simulink model "RealModel"  (R2016a)
(part 3 of 7)

x_dotdot = [x2, (0. + ((0.12348*cos(x1) - 0.9716*cos(x3))*(-0.4858*sin(2.*x1)*(0.12347999999999999*sin(x1) + 0.4858*cos(x3)*sin(2.*x1))*sin(x3)*(cos(x3)*(-0.0005*cos(2.*x1) - 0.7010000000000001*sin(2.*x1)) - 1.1102230246251565^-16*sin(x1)*sin(x3)) - 0.34006*sin(2.*x1)*sin(x3)*(cos(x3)*(-0.0005*cos(2.*x1) - 0.7010000000000001*sin(2.*x1)) - 1.1102230246251565^-16*sin(x1)*sin(x3))^2 + 0.34006*(2.0940000000000003 - 0.7010000000000001*cos(2.*x1) + 0.0005*sin(2.*x1))*sin(2.*x1)*sin(x3)*((1.7510000000000001 + 2.1684043449710084^-19*0) + cos(2.*x1)*((0.3505 - 5.421010862427521^-20*0) + (0.3505 - 5.421010862427521^-20*0)*cos(2.*x3)) + cos(2.*x3)*(0.343 - (0.00025 - 2.8760394919088917^-17*0)*sin(2.*x1)) - (0.00025 - 2.8760394919088917^-17*0)*sin(2.*x1) + 1.1102230246251562^-16*cos(x1)*sin(2.*x3)) + (2.0940000000000003 - 0.7010000000000001*cos(2.*x1) + 0.0005*sin(2.*x1))*(0.12347999999999999*sin(x1) + 0.4858*cos(x3)*sin(2.*x1))*(-0.12347999999999999*cos(x1)*sin(x3) + (-0.24289999999999998 - 0.24289999999999998*cos(2.*x1))*sin(2.*x3))) - (0. + (2.0940000000000003 - 0.7010000000000001*cos(2.*x1) + 0.0005*sin(2.*x1))*(-1.1102230246251565^-16*cos(x1)*cos(x3) - 1.4080000000000001*sin(x3)))*((0.8627035999999999 + cos(2.*x1)*(0.17003 - 0.17003*cos(2.*x3)) - 0.17003*cos(2.*x3))*(0.12347999999999999*sin(x1) + 0.4858*cos(x3)*sin(2.*x1)) + 0.34006*sin(2.*x1)*sin(x3)*(-0.12347999999999999*cos(x1)*sin(x3) - (0.2429 + 2.7105054312137602^-20*0)*(1. + 1.*cos(2.*x1))*sin(2.*x3))) - 0.12348*sin(x1)*sin(x3)*(-((0.8627035999999999 + cos(2.*x1)*(0.17003 - 0.17003*cos(2.*x3)) - 0.17003*cos(2.*x3))*(cos(x3)*(-0.0005*cos(2.*x1) - 0.7010000000000001*sin(2.*x1)) - 1.1102230246251565^-16*sin(x1)*sin(x3))^2) + (0.8627035999999999 + cos(2.*x1)*(0.17003 - 0.17003*cos(2.*x3)) - 0.17003*cos(2.*x3))*(2.0940000000000003 - 0.7010000000000001*cos(2.*x1) + 0.0005*sin(2.*x1))*((1.7510000000000001 + 2.1684043449710084^-19*0) + cos(2.*x1)*((0.3505 - 5.421010862427521^-20*0) + (0.3505 - 5.421010862427521^-20*0)*cos(2.*x3)) + cos(2.*x3)*(0.343 - (0.00025 - 2.8760394919088917^-17*0)*sin(2.*x1)) - (0.00025 - 2.8760394919088917^-17*0)*sin(2.*x1) + 1.1102230246251562^-16*cos(x1)*sin(2.*x3)) + 0.4858*sin(2.*x1)*sin(x3)*(cos(x3)*(-0.0005*cos(2.*x1) - 0.7010000000000001*sin(2.*x1)) - 1.1102230246251565^-16*sin(x1)*sin(x3))*(-0.12347999999999999*cos(x1)*sin(x3) - (0.2429 + 2.7105054312137602^-20*0)*(1. + 1.*cos(2.*x1))*sin(2.*x3)) - (2.0940000000000003 - 0.7010000000000001*cos(2.*x1) + 0.0005*sin(2.*x1))*(-0.12347999999999999*cos(x1)*sin(x3) + (-0.24289999999999998 - 0.24289999999999998*cos(2.*x1))*sin(2.*x3))*(-0.12347999999999999*cos(x1)*sin(x3) - (0.2429 + 2.7105054312137602^-20*0)*(1. + 1.*cos(2.*x1))*sin(2.*x3))))*((1.4288690166235203*cos(x1) + 1.6499158227686102*sin(x1))*u1 + 1.6499158227686104*sin(x1)*u2 + 1.6499158227686102*sin(x1)*u3 + 0.68012*sin(2.*x1)*x10*x2 + cos(x1)*(-1.4288690166235203*u3 - 0.12348*sin(x3)*x2^2) - 0.24696*cos(x3)*sin(x1)*x2*x4 - 0.9716000000000001*sin(2.*x1)*x2*x4 - 0.12348*cos(x1)*sin(x3)*x4^2 + ((0.12347999999999998*cos(x1) + 0.9716*cos(x1)^2*cos(x3) - 0.9716*cos(x3)*sin(x1)^2)*x2 - 0.4858*sin(2*x1)*sin(x3)*x4)*x6 + (-0.68012*cos(2.*x1)*sin(x3)*x2 - 0.34006*cos(x3)*sin(2.*x1)*x4)*x8) + (0.8627035999999999 + cos(2.*x1)*(0.17003 - 0.17003*cos(2.*x3)) - 0.17003*cos(2.*x3))*(-0.9715999999999999*cos(x1)^2 + 0.12347999999999999*cos(x1)*cos(x3) - 1.9431999999999998*sin(x1)^2)*(0.12347999999999999*sin(x1) + 0.4858*cos(x3)*sin(2.*x1))*(-1.1102230246251565^-16*cos(x1)*cos(x3) - 1.4080000000000001*sin(x3))*(-17.304840000000002*cos(x1)*sin(x3) + (-0.8164965809277263*cos(x1) - 0.9428090415820632*sin(x1))*u1 + (0.6123724356957947*cos(x1) - 0.9428090415820637*sin(x1))*u2 + 2.041241452319315*cos(x1)*u3 - 0.9428090415820632*sin(x1)*u3 - 0.9716*sin(2.*x1)*x10*x2 + 1.1102230246251565^-16*cos(x1)*x2^2 + (-1.3877787807814457^-17*cos(x1)*sin(x3)*x10 + (0.001*cos(2.*x1) + 1.4020000000000001*sin(2.*x1))*x2)*x4 + (-1.1102230246251565^-16*cos(x1)*cos(2.*x3) + ((0.343 - 1.4444474582904269^-34*0) + (0.35050000000000003 - 1.6263032587282571^-19*0)*cos(2.*x1) - (0.00025 - 1.3877787807814454^-16*0)*sin(2.*x1))*sin(2.*x3))*x6^2 + (0.34006000000000003*cos(x3)*sin(2.*x1)*x10 + (-0.9716 + 0.9716*cos(2.*x1))*sin(x3)*x2)*x8 + (-0.34006000000000003*cos(2.*x1)*cos(x3)*sin(x3) - 0.17003000000000001*sin(2.*x3))*x8^2 + x6*(0.4858*sin(2.*x1)*sin(x3)*x10 + (cos(x3)*(1.4080000000000001 - 1.4020000000000001*cos(2.*x1) + 0.001*sin(2.*x1)) - 2.220446049250313^-16*cos(x1)*sin(x3))*x2 + 1.1102230246251565^-16*sin(2.*x1)*sin(x3)*x4 + (0.12348*cos(x1)*cos(x3) + (0.4858 + 0.4858*cos(2.*x1))*cos(2.*x3))*x8)) + 0.4858*(0.12348*cos(x1) - 0.9716*cos(x3))*(0.12347999999999999 + 0.9715999999999999*cos(x1)*cos(x3))*sin(x1)*sin(2.*x1)*(0.12347999999999999*sin(x1) + 0.4858*cos(x3)*sin(2.*x1))*sin(x3)*(-17.304840000000002*cos(x1)*sin(x3) + (-0.8164965809277263*cos(x1) - 0.9428090415820632*sin(x1))*u1 + (0.6123724356957947*cos(x1) - 0.9428090415820637*sin(x1))*u2 + 2.041241452319315*cos(x1)*u3 - 0.9428090415820632*sin(x1)*u3 - 0.9716*sin(2.*x1)*x10*x2 + 1.1102230246251565^-16*cos(x1)*x2^2 + (-1.3877787807814457^-17*cos(x1)*sin(x3)*x10 + (0.001*cos(2.*x1) + 1.4020000000000001*sin(2.*x1))*x2)*x4 + (-1.1102230246251565^-16*cos(x1)*cos(2.*x3) + ((0.343 - 1.4444474582904269^-34*0) + (0.35050000000000003 - 1.6263032587282571^-19*0)*cos(2.*x1) - (0.00025 - 1.3877787807814454^-16*0)*sin(2.*x1))*sin(2.*x3))*x6^2 + (0.34006000000000003*cos(x3)*sin(2.*x1)*x10 + (-0.9716 + 0.9716*cos(2.*x1))*sin(x3)*x2)*x8 + (-0.34006000000000003*cos(2.*x1)*cos(x3)*sin(x3) - 0.17003000000000001*sin(2.*x3))*x8^2 + x6*(0.4858*sin(2.*x1)*sin(x3)*x10 + (cos(x3)*(1.4080000000000001 - 1.4020000000000001*cos(2.*x1) + 0.001*sin(2.*x1)) - 2.220446049250313^-16*cos(x1)*sin(x3))*x2 + 1.1102230246251565^-16*sin(2.*x1)*sin(x3)*x4 + (0.12348*cos(x1)*cos(x3) + (0.4858 + 0.4858*cos(2.*x1))*cos(2.*x3))*x8)) + 0.165201148*sin(2.*x1)^2*(0.12347999999999999*sin(x1) + 0.4858*cos(x3)*sin(2.*x1))*(-1.1102230246251565^-16*cos(x1)*cos(x3) - 1.4080000000000001*sin(x3))*sin(x3)^2*(-17.304840000000002*cos(x1)*sin(x3) + (-0.8164965809277263*cos(x1) - 0.9428090415820632*sin(x1))*u1 + (0.6123724356957947*cos(x1) - 0.9428090415820637*sin(x1))*u2 + 2.041241452319315*cos(x1)*u3 - 0.9428090415820632*sin(x1)*u3 - 0.9716*sin(2.*x1)*x10*x2 + 1.1102230246251565^-16*cos(x1)*x2^2 + (-1.3877787807814457^-17*cos(x1)*sin(x3)*x10 + (0.001*cos(2.*x1) + 1.4020000000000001*sin(2.*x1))*x2)*x4 + (-1.1102230246251565^-16*cos(x1)*cos(2.*x3) + ((0.343 - 1.4444474582904269^-34*0) + (0.35050000000000003 - 1.6263032587282571^-19*0)*cos(2.*x1) - (0.00025 - 1.3877787807814454^-16*0)*sin(2.*x1))*sin(2.*x3))*x6^2 + (0.34006000000000003*cos(x3)*sin(2.*x1)*x10 + (-0.9716 + 0.9716*cos(2.*x1))*sin(x3)*x2)*x8 + (-0.34006000000000003*cos(2.*x1)*cos(x3)*sin(x3) - 0.17003000000000001*sin(2.*x3))*x8^2 + x6*(0.4858*sin(2.*x1)*sin(x3)*x10 + (cos(x3)*(1.4080000000000001 - 1.4020000000000001*cos(2.*x1) + 0.001*sin(2.*x1)) - 2.220446049250313^-16*cos(x1)*sin(x3))*x2 + 1.1102230246251565^-16*sin(2.*x1)*sin(x3)*x4 + (0.12348*cos(x1)*cos(x3) + (0.4858 + 0.4858*cos(2.*x1))*cos(2.*x3))*x8)) - (1.0327336 - 0.34006*cos(2.*x1))*(0.8627035999999999 + cos(2.*x1)*(0.17003 - 0.17003*cos(2.*x3)) - 0.17003*cos(2.*x3))*(-1.1102230246251565^-16*cos(x1)*cos(x3) - 1.4080000000000001*sin(x3))*(cos(x3)*(-0.0005*cos(2.*x1) - 0.701*sin(2.*x1)) - 1.1102230246251564^-16*sin(x1)*sin(x3))*(-17.304840000000002*cos(x1)*sin(x3) + (-0.8164965809277263*cos(x1) - 0.9428090415820632*sin(x1))*u1 + (0.6123724356957947*cos(x1) - 0.9428090415820637*sin(x1))*u2 + 2.041241452319315*cos(x1)*u3 - 0.9428090415820632*sin(x1)*u3 - 0.9716*sin(2.*x1)*x10*x2 + 1.1102230246251565^-16*cos(x1)*x2^2 + (-1.3877787807814457^-17*cos(x1)*sin(x3)*x10 + (0.001*cos(2.*x1) + 1.4020000000000001*sin(2.*x1))*x2)*x4 + (-1.1102230246251565^-16*cos(x1)*cos(2.*x3) + ((0.343 - 1.4444474582904269^-34*0) + (0.35050000000000003 - 1.6263032587282571^-19*0)*cos(2.*x1) - (0.00025 - 1.3877787807814454^-16*0)*sin(2.*x1))*sin(2.*x3))*x6^2 + (0.34006000000000003*cos(x3)*sin(2.*x1)*x10 + (-0.9716 + 0.9716*cos(2.*x1))*sin(x3)*x2)*x8 + (-0.34006000000000003*cos(2.*x1)*cos(x3)*sin(x3) - 0.17003000000000001*sin(2.*x3))*x8^2 + x6*(0.4858*sin(2.*x1)*sin(x3)*x10 + (cos(x3)*(1.4080000000000001 - 1.4020000000000001*cos(2.*x1) + 0.001*sin(2.*x1)) - 2.220446049250313^-16*cos(x1)*sin(x3))*x2 + 1.1102230246251565^-16*sin(2.*x1)*sin(x3)*x4 + (0.12348*cos(x1)*cos(x3) + (0.4858 + 0.4858*cos(2.*x1))*cos(2.*x3))*x8)) - 0.12348*(0.12347999999999999 + 0.9715999999999999*cos(x1)*cos(x3))*(0.8627035999999999 + cos(2.*x1)*(0.17003 - 0.17003*cos(2.*x3)) - 0.17003*cos(2.*x3))*sin(x1)^2*sin(x3)*(cos(x3)*(-0.0005*cos(2.*x1) - 0.701*sin(2.*x1)) - 1.1102230246251564^-16*sin(x1)*sin(x3))*(-17.304840000000002*cos(x1)*sin(x3) + (-0.8164965809277263*cos(x1) - 0.9428090415820632*sin(x1))*u1 + (0.6123724356957947*cos(x1) - 0.9428090415820637*sin(x1))*u2 + 2.041241452319315*cos(x1)*u3 - 0.9428090415820632*sin(x1)*u3 - 0.9716*sin(2.*x1)*x10*x2 + 1.1102230246251565^-16*cos(x1)*x2^2 + (-1.3877787807814457^-17*cos(x1)*sin(x3)*x10 + (0.001*cos(2.*x1) + 1.4020000000000001*sin(2.*x1))*x2)*x4 + (-1.1102230246251565^-16*cos(x1)*cos(2.*x3) + ((0.343 - 1.4444474582904269^-34*0) + (0.35050000000000003 - 1.6263032587282571^-19*0)*cos(2.*x1) - (0.00025 - 1.3877787807814454^-16*0)*sin(2.*x1))*sin(2.*x3))*x6^2 + (0.34006000000000003*cos(x3)*sin(2.*x1)*x10 + (-0.9716 + 0.9716*cos(2.*x1))*sin(x3)*x2)*x8 + (-0.34006000000000003*cos(2.*x1)*cos(x3)*sin(x3) - 0.17003000000000001*sin(2.*x3))*x8^2 + x6*(0.4858*sin(2.*x1)*sin(x3)*x10 + (cos(x3)*(1.4080000000000001 - 1.4020000000000001*cos(2.*x1) + 0.001*sin(2.*x1)) - 2.220446049250313^-16*cos(x1)*sin(x3))*x2 + 1.1102230246251565^-16*sin(2.*x1)*sin(x3)*x4 + (0.12348*cos(x1)*cos(x3) + (0.4858 + 0.4858*cos(2.*x1))*cos(2.*x3))*x8)) + 0.34006*(0.12348*cos(x1) - 0.9716*cos(x3))*(0.12347999999999999 + 0.9715999999999999*cos(x1)*cos(x3))*sin(x1)*sin(2.*x1)*sin(x3)*(cos(x3)*(-0.0005*cos(2.*x1) - 0.701*sin(2.*x1)) - 1.1102230246251564^-16*sin(x1)*sin(x3))*(-17.304840000000002*cos(x1)*sin(x3) + (-0.8164965809277263*cos(x1) - 0.9428090415820632*sin(x1))*u1 + (0.6123724356957947*cos(x1) - 0.9428090415820637*sin(x1))*u2 + 2.041241452319315*cos(x1)*u3 - 0.9428090415820632*sin(x1)*u3 - 0.9716*sin(2.*x1)*x10*x2 + 1.1102230246251565^-16*cos(x1)*x2^2 + (-1.3877787807814457^-17*cos(x1)*sin(x3)*x10 + (0.001*cos(2.*x1) + 1.4020000000000001*sin(2.*x1))*x2)*x4 + (-1.1102230246251565^-16*cos(x1)*cos(2.*x3) + ((0.343 - 1.4444474582904269^-34*0) + (0.35050000000000003 - 1.6263032587282571^-19*0)*cos(2.*x1) - (0.00025 - 1.3877787807814454^-16*0)*sin(2.*x1))*sin(2.*x3))*x6^2 + (0.34006000000000003*cos(x3)*sin(2.*x1)*x10 + (-0.9716 + 0.9716*cos(2.*x1))*sin(x3)*x2)*x8 + (-0.34006000000000003*cos(2.*x1)*cos(x3)*sin(x3) - 0.17003000000000001*sin(2.*x3))*x8^2 + x6*(0.4858*sin(2.*x1)*sin(x3)*x10 + (cos(x3)*(1.4080000000000001 - 1.4020000000000001*cos(2.*x1) + 0.001*sin(2.*x1)) - 2.220446049250313^-16*cos(x1)*sin(x3))*x2 + 1.1102230246251565^-16*sin(2.*x1)*sin(x3)*x4 + (0.12348*cos(x1)*cos(x3) + (0.4858 + 0.4858*cos(2.*x1))*cos(2.*x3))*x8)) + 0.11564080359999998*sin(2.*x1)^2*(-1.1102230246251565^-16*cos(x1)*cos(x3) - 1.4080000000000001*sin(x3))*sin(x3)^2*(cos(x3)*(-0.0005*cos(2.*x1) - 0.701*sin(2.*x1)) - 1.1102230246251564^-16*sin(x1)*sin(x3))*(-17.304840000000002*cos(x1)*sin(x3) + (-0.8164965809277263*cos(x1) - 0.9428090415820632*sin(x1))*u1 + (0.6123724356957947*cos(x1) - 0.9428090415820637*sin(x1))*u2 + 2.041241452319315*cos(x1)*u3 - 0.9428090415820632*sin(x1)*u3 - 0.9716*sin(2.*x1)*x10*x2 + 1.1102230246251565^-16*cos(x1)*x2^2 + (-1.3877787807814457^-17*cos(x1)*sin(x3)*x10 + (0.001*cos(2.*x1) + 1.4020000000000001*sin(2.*x1))*x2)*x4 + (-1.1102230246251565^-16*cos(x1)*cos(2.*x3) + ((0.343 - 1.4444474582904269^-34*0) + (0.35050000000000003 - 1.6263032587282571^-19*0)*cos(2.*x1) - (0.00025 - 1.3877787807814454^-16*0)*sin(2.*x1))*sin(2.*x3))*x6^2 + (0.34006000000000003*cos(x3)*sin(2.*x1)*x10 + (-0.9716 + 0.9716*cos(2.*x1))*sin(x3)*x2)*x8 + (-0.34006000000000003*cos(2.*x1)*cos(x3)*sin(x3) - 0.17003000000000001*sin(2.*x3))*x8^2 + x6*(0.4858*sin(2.*x1)*sin(x3)*x10 + (cos(x3)*(1.4080000000000001 - 1.4020000000000001*cos(2.*x1) + 0.001*sin(2.*x1)) - 2.220446049250313^-16*cos(x1)*sin(x3))*x2 + 1.1102230246251565^-16*sin(2.*x1)*sin(x3)*x4 + (0.12348*cos(x1)*cos(x3) + (0.4858 + 0.4858*cos(2.*x1))*cos(2.*x3))*x8)) + 0.12348*(0.8627035999999999 + cos(2.*x1)*(0.17003 - 0.17003*cos(2.*x3)) - 0.17003*cos(2.*x3))*sin(x1)*(-0.9715999999999999*cos(x1)^2 + 0.12347999999999999*cos(x1)*cos(x3) - 1.9431999999999998*sin(x1)^2)*sin(x3)*((1.7510000000000001 + 2.1684043449710084^-19*0) + cos(2.*x1)*((0.3505 - 5.421010862427521^-20*0) + (0.3505 - 5.421010862427521^-20*0)*cos(2.*x3)) + cos(2.*x3)*(0.343 - (0.00025 - 2.8760394919088917^-17*0)*sin(2.*x1)) - (0.00025 - 2.8760394919088917^-17*0)*sin(2.*x1) + 1.1102230246251562^-16*cos(x1)*sin(2.*x3))*(-17.304840000000002*cos(x1)*sin(x3) + (-0.8164965809277263*cos(x1) - 0.9428090415820632*sin(x1))*u1 + (0.6123724356957947*cos(x1) - 0.9428090415820637*sin(x1))*u2 + 2.041241452319315*cos(x1)*u3 - 0.9428090415820632*sin(x1)*u3 - 0.9716*sin(2.*x1)*x10*x2 + 1.1102230246251565^-16*cos(x1)*x2^2 + (-1.3877787807814457^-17*cos(x1)*sin(x3)*x10 + (0.001*cos(2.*x1) + 1.4020000000000001*sin(2.*x1))*x2)*x4 + (-1.1102230246251565^-16*cos(x1)*cos(2.*x3) + ((0.343 - 1.4444474582904269^-34*0) + (0.35050000000000003 - 1.6263032587282571^-19*0)*cos(2.*x1) - (0.00025 - 1.3877787807814454^-16*0)*sin(2.*x1))*sin(2.*x3))*x6^2 + (0.34006000000000003*cos(x3)*sin(2.*x1)*x10 + (-0.9716 + 0.9716*cos(2.*x1))*sin(x3)*x2)*x8 + (-0.34006000000000003*cos(2.*x1)*cos(x3)*sin(x3) - 0.17003000000000001*sin(2.*x3))*x8^2 + x6*(0.4858*sin(2.*x1)*sin(x3)*x10 + (cos(x3)*(1.4080000000000001 - 1.4020000000000001*cos(2.*x1) + 0.001*sin(2.*x1)) - 2.220446049250313^-16*cos(x1)*sin(x3))*x2 + 1.1102230246251565^-16*sin(2.*x1)*sin(x3)*x4 + (0.12348*cos(x1)*cos(x3) + (0.4858 + 0.4858*cos(2.*x1))*cos(2.*x3))*x8)) - 0.4858*(1.0327336 - 0.34006*cos(2.*x1))*(0.12348*cos(x1) - 0.9716*cos(x3))*sin(2.*x1)*sin(x3)*((1.7510000000000001 + 2.1684043449710084^-19*0) + cos(2.*x1)*((0.3505 - 5.421010862427521^-20*0) + (0.3505 - 5.421010862427521^-20*0)*cos(2.*x3)) + cos(2.*x3)*(0.343 - (0.00025 - 2.8760394919088917^-17*0)*sin(2.*x1)) - (0.00025 - 2.8760394919088917^-17*0)*sin(2.*x1) + 1.1102230246251562^-16*cos(x1)*sin(2.*x3))*(-17.304840000000002*cos(x1)*sin(x3) + (-0.8164965809277263*cos(x1) - 0.9428090415820632*sin(x1))*u1 + (0.6123724356957947*cos(x1) - 0.9428090415820637*sin(x1))*u2 + 2.041241452319315*cos(x1)*u3 - 0.9428090415820632*sin(x1)*u3 - 0.9716*sin(2.*x1)*x10*x2 + 1.1102230246251565^-16*cos(x1)*x2^2 + (-1.3877787807814457^-17*cos(x1)*sin(x3)*x10 + (0.001*cos(2.*x1) + 1.4020000000000001*sin(2.*x1))*x2)*x4 + (-1.1102230246251565^-16*cos(x1)*cos(2.*x3) + ((0.343 - 1.4444474582904269^-34*0) + (0.35050000000000003 - 1.6263032587282571^-19*0)*cos(2.*x1) - (0.00025 - 1.3877787807814454^-16*0)*sin(2.*x1))*sin(2.*x3))*x6^2 + (0.34006000000000003*cos(x3)*sin(2.*x1)*x10 + (-0.9716 + 0.9716*cos(2.*x1))*sin(x3)*x2)*x8 + (-0.34006000000000003*cos(2.*x1)*cos(x3)*sin(x3) - 0.17003000000000001*sin(2.*x3))*x8^2 + x6*(0.4858*sin(2.*x1)*sin(x3)*x10 + (cos(x3)*(1.4080000000000001 - 1.4020000000000001*cos(2.*x1) + 0.001*sin(2.*x1)) - 2.220446049250313^-16*cos(x1)*sin(x3))*x2 + 1.1102230246251565^-16*sin(2.*x1)*sin(x3)*x4 + (0.12348*cos(x1)*cos(x3) + (0.4858 + 0.4858*cos(2.*x1))*cos(2.*x3))*x8)) - 0.34006*(0.12348*cos(x1) - 0.9716*cos(x3))*(-0.9715999999999999*cos(x1)^2 + 0.12347999999999999*cos(x1)*cos(x3) - 1.9431999999999998*sin(x1)^2)*sin(2.*x1)*sin(x3)*((1.7510000000000001 + 2.1684043449710084^-19*0) + cos(2.*x1)*((0.3505 - 5.421010862427521^-20*0) + (0.3505 - 5.421010862427521^-20*0)*cos(2.*x3)) + cos(2.*x3)*(0.343 - (0.00025 - 2.8760394919088917^-17*0)*sin(2.*x1)) - (0.00025 - 2.8760394919088917^-17*0)*sin(2.*x1) + 1.1102230246251562^-16*cos(x1)*sin(2.*x3))*(-17.304840000000002*cos(x1)*sin(x3) + (-0.8164965809277263*cos(x1) - 0.9428090415820632*sin(x1))*u1 + (0.6123724356957947*cos(x1) - 0.9428090415820637*sin(x1))*u2 + 2.041241452319315*cos(x1)*u3 - 0.9428090415820632*sin(x1)*u3 - 0.9716*sin(2.*x1)*x10*x2 + 1.1102230246251565^-16*cos(x1)*x2^2 + (-1.3877787807814457^-17*cos(x1)*sin(x3)*x10 + (0.001*cos(2.*x1) + 1.4020000000000001*sin(2.*x1))*x2)*x4 + (-1.1102230246251565^-16*cos(x1)*cos(2.*x3) + ((0.343 - 1.4444474582904269^-34*0) + (0.35050000000000003 - 1.6263032587282571^-19*0)*cos(2.*x1) - (0.00025 - 1.3877787807814454^-16*0)*sin(2.*x1))*sin(2.*x3))*x6^2 + (0.34006000000000003*cos(x3)*sin(2.*x1)*x10 + (-0.9716 + 0.9716*cos(2.*x1))*sin(x3)*x2)*x8 + (-0.34006000000000003*cos(2.*x1)*cos(x3)*sin(x3) - 0.17003000000000001*sin(2.*x3))*x8^2 + x6*(0.4858*sin(2.*x1)*sin(x3)*x10 + (cos(x3)*(1.4080000000000001 - 1.4020000000000001*cos(2.*x1) + 0.001*sin(2.*x1)) - 2.220446049250313^-16*cos(x1)*sin(x3))*x2 + 1.1102230246251565^-16*sin(2.*x1)*sin(x3)*x4 + (0.12348*cos(x1)*cos(x3) + (0.4858 + 0.4858*cos(2.*x1))*cos(2.*x3))*x8)) + 0.020399037755039998*sin(x1)*sin(2.*x1)^2*sin(x3)^3*((1.7510000000000001 + 2.1684043449710084^-19*0) + cos(2.*x1)*((0.3505 - 5.421010862427521^-20*0) + (0.3505 - 5.421010862427521^-20*0)*cos(2.*x3)) + cos(2.*x3)*(0.343 - (0.00025 - 2.8760394919088917^-17*0)*sin(2.*x1)) - (0.00025 - 2.8760394919088917^-17*0)*sin(2.*x1) + 1.1102230246251562^-16*cos(x1)*sin(2.*x3))*(-17.304840000000002*cos(x1)*sin(x3) + (-0.8164965809277263*cos(x1) - 0.9428090415820632*sin(x1))*u1 + (0.6123724356957947*cos(x1) - 0.9428090415820637*sin(x1))*u2 + 2.041241452319315*cos(x1)*u3 - 0.9428090415820632*sin(x1)*u3 - 0.9716*sin(2.*x1)*x10*x2 + 1.1102230246251565^-16*cos(x1)*x2^2 + (-1.3877787807814457^-17*cos(x1)*sin(x3)*x10 + (0.001*cos(2.*x1) + 1.4020000000000001*sin(2.*x1))*x2)*x4 + (-1.1102230246251565^-16*cos(x1)*cos(2.*x3) + ((0.343 - 1.4444474582904269^-34*0) + (0.35050000000000003 - 1.6263032587282571^-19*0)*cos(2.*x1) - (0.00025 - 1.3877787807814454^-16*0)*sin(2.*x1))*sin(2.*x3))*x6^2 + (0.34006000000000003*cos(x3)*sin(2.*x1)*x10 + (-0.9716 + 0.9716*cos(2.*x1))*sin(x3)*x2)*x8 + (-0.34006000000000003*cos(2.*x1)*cos(x3)*sin(x3) - 0.17003000000000001*sin(2.*x3))*x8^2 + x6*(0.4858*sin(2.*x1)*sin(x3)*x10 + (cos(x3)*(1.4080000000000001 - 1.4020000000000001*cos(2.*x1) + 0.001*sin(2.*x1)) - 2.220446049250313^-16*cos(x1)*sin(x3))*x2 + 1.1102230246251565^-16*sin(2.*x1)*sin(x3)*x4 + (0.12348*cos(x1)*cos(x3) + (0.4858 + 0.4858*cos(2.*x1))*cos(2.*x3))*x8)) - (0.12348*cos(x1) - 0.9716*cos(x3))*(-0.9715999999999999*cos(x1)^2 + 0.12347999999999999*cos(x1)*cos(x3) - 1.9431999999999998*sin(x1)^2)*(0.12347999999999999*sin(x1) + 0.4858*cos(x3)*sin(2.*x1))*(-0.12347999999999999*cos(x1)*sin(x3) + (-0.24289999999999998 - 0.24289999999999998*cos(2.*x1))*sin(2.*x3))*(-17.304840000000002*cos(x1)*sin(x3) + (-0.8164965809277263*cos(x1) - 0.9428090415820632*sin(x1))*u1 + (0.6123724356957947*cos(x1) - 0.9428090415820637*sin(x1))*u2 + 2.041241452319315*cos(x1)*u3 - 0.9428090415820632*sin(x1)*u3 - 0.9716*sin(2.*x1)*x10*x2 + 1.1102230246251565^-16*cos(x1)*x2^2 + (-1.3877787807814457^-17*cos(x1)*sin(x3)*x10 + (0.001*cos(2.*x1) + 1.4020000000000001*sin(2.*x1))*x2)*x4 + (-1.1102230246251565^-16*cos(x1)*cos(2.*x3) + ((0.343 - 1.4444474582904269^-34*0) + (0.35050000000000003 - 1.6263032587282571^-19*0)*cos(2.*x1) - (0.00025 - 1.3877787807814454^-16*0)*sin(2.*x1))*sin(2.*x3))*x6^2 + (0.34006000000000003*cos(x3)*sin(2.*x1)*x10 + (-0.9716 + 0.9716*cos(2.*x1))*sin(x3)*x2)*x8 + (-0.34006000000000003*cos(2.*x1)*cos(x3)*sin(x3) - 0.17003000000000001*sin(2.*x3))*x8^2 + x6*(0.4858*sin(2.*x1)*sin(x3)*x10 + (cos(x3)*(1.4080000000000001 - 1.4020000000000001*cos(2.*x1) + 0.001*sin(2.*x1)) - 2.220446049250313^-16*cos(x1)*sin(x3))*x2 + 1.1102230246251565^-16*sin(2.*x1)*sin(x3)*x4 + (0.12348*cos(x1)*cos(x3) + (0.4858 + 0.4858*cos(2.*x1))*cos(2.*x3))*x8)) + (1.0327336 - 0.34006*cos(2.*x1))*(0.12348*cos(x1) - 0.9716*cos(x3))*(cos(x3)*(-0.0005*cos(2.*x1) - 0.701*sin(2.*x1)) - 1.1102230246251564^-16*sin(x1)*sin(x3))*(-0.12347999999999999*cos(x1)*sin(x3) + (-0.24289999999999998 - 0.24289999999999998*cos(2.*x1))*sin(2.*x3))*(-17.304840000000002*cos(x1)*sin(x3) + (-0.8164965809277263*cos(x1) - 0.9428090415820632*sin(x1))*u1 + (0.6123724356957947*cos(x1) - 0.9428090415820637*sin(x1))*u2 + 2.041241452319315*cos(x1)*u3 - 0.9428090415820632*sin(x1)*u3 - 0.9716*sin(2.*x1)*x10*x2 + 1.1102230246251565^-16*cos(x1)*x2^2 + (-1.3877787807814457^-17*cos(x1)*sin(x3)*x10 + (0.001*cos(2.*x1) + 1.4020000000000001*sin(2.*x1))*x2)*x4 + (-1.1102230246251565^-16*cos(x1)*cos(2.*x3) + ((0.343 - 1.4444474582904269^-34*0) + (0.35050000000000003 - 1.6263032587282571^-19*0)*cos(2.*x1) - (0.00025 - 1.3877787807814454^-16*0)*sin(2.*x1))*sin(2.*x3))*x6^2 + (0.34006000000000003*cos(x3)*sin(2.*x1)*x10 + (-0.9716 + 0.9716*cos(2.*x1))*sin(x3)*x2)*x8 + (-0.34006000000000003*cos(2.*x1)*cos(x3)*sin(x3) - 0.17003000000000001*sin(2.*x3))*x8^2 + x6*(0.4858*sin(2.*x1)*sin(x3)*x10 + (cos(x3)*(1.4080000000000001 - 1.4020000000000001*cos(2.*x1) + 0.001*sin(2.*x1)) - 2.220446049250313^-16*cos(x1)*sin(x3))*x2 + 1.1102230246251565^-16*sin(2.*x1)*sin(x3)*x4 + (0.12348*cos(x1)*cos(x3) + (0.4858 + 0.4858*cos(2.*x1))*cos(2.*x3))*x8)) - 0.041990608799999996*sin(x1)*sin(2.*x1)*sin(x3)^2*(cos(x3)*(-0.0005*cos(2.*x1) - 0.701*sin(2.*x1)) - 1.1102230246251564^-16*sin(x1)*sin(x3))*(-0.12347999999999999*cos(x1)*sin(x3) + (-0.24289999999999998 - 0.24289999999999998*cos(2.*x1))*sin(2.*x3))*(-17.304840000000002*cos(x1)*sin(x3) + (-0.8164965809277263*cos(x1) - 0.9428090415820632*sin(x1))*u1 + (0.6123724356957947*cos(x1) - 0.9428090415820637*sin(x1))*u2 + 2.041241452319315*cos(x1)*u3 - 0.9428090415820632*sin(x1)*u3 - 0.9716*sin(2.*x1)*x10*x2 + 1.1102230246251565^-16*cos(x1)*x2^2 + (-1.3877787807814457^-17*cos(x1)*sin(x3)*x10 + (0.001*cos(2.*x1) + 1.4020000000000001*sin(2.*x1))*x2)*x4 + (-1.1102230246251565^-16*cos(x1)*cos(2.*x3) + ((0.343 - 1.4444474582904269^-34*0) + (0.35050000000000003 - 1.6263032587282571^-19*0)*cos(2.*x1) - (0.00025 - 1.3877787807814454^-16*0)*sin(2.*x1))*sin(2.*x3))*x6^2 + (0.34006000000000003*cos(x3)*sin(2.*x1)*x10 + (-0.9716 + 0.9716*cos(2.*x1))*sin(x3)*x2)*x8 + (-0.34006000000000003*cos(2.*x1)*cos(x3)*sin(x3) - 0.17003000000000001*sin(2.*x3))*x8^2 + x6*(0.4858*sin(2.*x1)*sin(x3)*x10 + (cos(x3)*(1.4080000000000001 - 1.4020000000000001*cos(2.*x1) + 0.001*sin(2.*x1)) - 2.220446049250313^-16*cos(x1)*sin(x3))*x2 + 1.1102230246251565^-16*sin(2.*x1)*sin(x3)*x4 + (0.12348*cos(x1)*cos(x3) + (0.4858 + 0.4858*cos(2.*x1))*cos(2.*x3))*x8)) + 0.4858*(1.0327336 - 0.34006*cos(2.*x1))*sin(2.*x1)*(-1.1102230246251565^-16*cos(x1)*cos(x3) - 1.4080000000000001*sin(x3))*sin(x3)*(-0.12347999999999999*cos(x1)*sin(x3) - (0.2429 + 2.7105054312137602^-20*0)*(1. + 1.*cos(2.*x1))*sin(2.*x3))*(-17.304840000000002*cos(x1)*sin(x3) + (-0.8164965809277263*cos(x1) - 0.9428090415820632*sin(x1))*u1 + (0.6123724356957947*cos(x1) - 0.9428090415820637*sin(x1))*u2 + 2.041241452319315*cos(x1)*u3 - 0.9428090415820632*sin(x1)*u3 - 0.9716*sin(2.*x1)*x10*x2 + 1.1102230246251565^-16*cos(x1)*x2^2 + (-1.3877787807814457^-17*cos(x1)*sin(x3)*x10 + (0.001*cos(2.*x1) + 1.4020000000000001*sin(2.*x1))*x2)*x4 + (-1.1102230246251565^-16*cos(x1)*cos(2.*x3) + ((0.343 - 1.4444474582904269^-34*0) + (0.35050000000000003 - 1.6263032587282571^-19*0)*cos(2.*x1) - (0.00025 - 1.3877787807814454^-16*0)*sin(2.*x1))*sin(2.*x3))*x6^2 + (0.34006000000000003*cos(x3)*sin(2.*x1)*x10 + (-0.9716 + 0.9716*cos(2.*x1))*sin(x3)*x2)*x8 + (-0.34006000000000003*cos(2.*x1)*cos(x3)*sin(x3) - 0.17003000000000001*sin(2.*x3))*x8^2 + x6*(0.4858*sin(2.*x1)*sin(x3)*x10 + (cos(x3)*(1.4080000000000001 - 1.4020000000000001*cos(2.*x1) + 0.001*sin(2.*x1)) - 2.220446049250313^-16*cos(x1)*sin(x3))*x2 + 1.1102230246251565^-16*sin(2.*x1)*sin(x3)*x4 + (0.12348*cos(x1)*cos(x3) + (0.4858 + 0.4858*cos(2.*x1))*cos(2.*x3))*x8)) + 0.34006*(-0.9715999999999999*cos(x1)^2 + 0.12347999999999999*cos(x1)*cos(x3) - 1.9431999999999998*sin(x1)^2)*sin(2.*x1)*(-1.1102230246251565^-16*cos(x1)*cos(x3) - 1.4080000000000001*sin(x3))*sin(x3)*(-0.12347999999999999*cos(x1)*sin(x3) - (0.2429 + 2.7105054312137602^-20*0)*(1. + 1.*cos(2.*x1))*sin(2.*x3))*(-17.304840000000002*cos(x1)*sin(x3) + (-0.8164965809277263*cos(x1) - 0.9428090415820632*sin(x1))*u1 + (0.6123724356957947*cos(x1) - 0.9428090415820637*sin(x1))*u2 + 2.041241452319315*cos(x1)*u3 - 0.9428090415820632*sin(x1)*u3 - 0.9716*sin(2.*x1)*x10*x2 + 1.1102230246251565^-16*cos(x1)*x2^2 + (-1.3877787807814457^-17*cos(x1)*sin(x3)*x10 + (0.001*cos(2.*x1) + 1.4020000000000001*sin(2.*x1))*x2)*x4 + (-1.1102230246251565^-16*cos(x1)*cos(2.*x3) + ((0.343 - 1.4444474582904269^-34*0) + (0.35050000000000003 - 1.6263032587282571^-19*0)*cos(2.*x1) - (0.00025 - 1.3877787807814454^-16*0)*sin(2.*x1))*sin(2.*x3))*x6^2 + (0.34006000000000003*cos(x3)*sin(2.*x1)*x10 + (-0.9716 + 0.9716*cos(2.*x1))*sin(x3)*x2)*x8 + (-0.34006000000000003*cos(2.*x1)*cos(x3)*sin(x3) - 0.17003000000000001*sin(2.*x3))*x8^2 + x6*(0.4858*sin(2.*x1)*sin(x3)*x10 + (cos(x3)*(1.4080000000000001 - 1.4020000000000001*cos(2.*x1) + 0.001*sin(2.*x1)) - 2.220446049250313^-16*cos(x1)*sin(x3))*x2 + 1.1102230246251565^-16*sin(2.*x1)*sin(x3)*x4 + (0.12348*cos(x1)*cos(x3) + (0.4858 + 0.4858*cos(2.*x1))*cos(2.*x3))*x8)) + 0.059986584*(0.12347999999999999 + 0.9715999999999999*cos(x1)*cos(x3))*sin(x1)^2*sin(2.*x1)*sin(x3)^2*(-0.12347999999999999*cos(x1)*sin(x3) - (0.2429 + 2.7105054312137602^-20*0)*(1. + 1.*cos(2.*x1))*sin(2.*x3))*(-17.304840000000002*cos(x1)*sin(x3) + (-0.8164965809277263*cos(x1) - 0.9428090415820632*sin(x1))*u1 + (0.6123724356957947*cos(x1) - 0.9428090415820637*sin(x1))*u2 + 2.041241452319315*cos(x1)*u3 - 0.9428090415820632*sin(x1)*u3 - 0.9716*sin(2.*x1)*x10*x2 + 1.1102230246251565^-16*cos(x1)*x2^2 + (-1.3877787807814457^-17*cos(x1)*sin(x3)*x10 + (0.001*cos(2.*x1) + 1.4020000000000001*sin(2.*x1))*x2)*x4 + (-1.1102230246251565^-16*cos(x1)*cos(2.*x3) + ((0.343 - 1.4444474582904269^-34*0) + (0.35050000000000003 - 1.6263032587282571^-19*0)*cos(2.*x1) - (0.00025 - 1.3877787807814454^-16*0)*sin(2.*x1))*sin(2.*x3))*x6^2 + (0.34006000000000003*cos(x3)*sin(2.*x1)*x10 + (-0.9716 + 0.9716*cos(2.*x1))*sin(x3)*x2)*x8 + (-0.34006000000000003*cos(2.*x1)*cos(x3)*sin(x3) - 0.17003000000000001*sin(2.*x3))*x8^2 + x6*(0.4858*sin(2.*x1)*sin(x3)*x10 + (cos(x3)*(1.4080000000000001 - 1.4020000000000001*cos(2.*x1) + 0.001*sin(2.*x1)) - 2.220446049250313^-16*cos(x1)*sin(x3))*x2 + 1.1102230246251565^-16*sin(2.*x1)*sin(x3)*x4 + (0.12348*cos(x1)*cos(x3) + (0.4858 + 0.4858*cos(2.*x1))*cos(2.*x3))*x8)) - 0.12348*sin(x1)*(-0.9715999999999999*cos(x1)^2 + 0.12347999999999999*cos(x1)*cos(x3) - 1.9431999999999998*sin(x1)^2)*sin(x3)*(-0.12347999999999999*cos(x1)*sin(x3) + (-0.24289999999999998 - 0.24289999999999998*cos(2.*x1))*sin(2.*x3))*(-0.12347999999999999*cos(x1)*sin(x3) - (0.2429 + 2.7105054312137602^-20*0)*(1. + 1.*cos(2.*x1))*sin(2.*x3))*(-17.304840000000002*cos(x1)*sin(x3) + (-0.8164965809277263*cos(x1) - 0.9428090415820632*sin(x1))*u1 + (0.6123724356957947*cos(x1) - 0.9428090415820637*sin(x1))*u2 + 2.041241452319315*cos(x1)*u3 - 0.9428090415820632*sin(x1)*u3 - 0.9716*sin(2.*x1)*x10*x2 + 1.1102230246251565^-16*cos(x1)*x2^2 + (-1.3877787807814457^-17*cos(x1)*sin(x3)*x10 + (0.001*cos(2.*x1) + 1.4020000000000001*sin(2.*x1))*x2)*x4 + (-1.1102230246251565^-16*cos(x1)*cos(2.*x3) + ((0.343 - 1.4444474582904269^-34*0) + (0.35050000000000003 - 1.6263032587282571^-19*0)*cos(2.*x1) - (0.00025 - 1.3877787807814454^-16*0)*sin(2.*x1))*sin(2.*x3))*x6^2 + (0.34006000000000003*cos(x3)*sin(2.*x1)*x10 + (-0.9716 + 0.9716*cos(2.*x1))*sin(x3)*x2)*x8 + (-0.34006000000000003*cos(2.*x1)*cos(x3)*sin(x3) - 0.17003000000000001*sin(2.*x3))*x8^2 + x6*(0.4858*sin(2.*x1)*sin(x3)*x10 + (cos(x3)*(1.4080000000000001 - 1.4020000000000001*cos(2.*x1) + 0.001*sin(2.*x1)) - 2.220446049250313^-16*cos(x1)*sin(x3))*x2 + 1.1102230246251565^-16*sin(2.*x1)*sin(x3)*x4 + (0.12348*cos(x1)*cos(x3) + (0.4858 + 0.4858*cos(2.*x1))*cos(2.*x3))*x8)) - (0.12348*cos(x1) - 0.9716*cos(x3))*(0.12347999999999999 + 0.9715999999999999*cos(x1)*cos(x3))*sin(x1)*(2.0940000000000003 - 0.7010000000000001*cos(2.*x1) + 0.0005*sin(2.*x1))*(0.12347999999999999*sin(x1) + 0.4858*cos(x3)*sin(2.*x1))*((0.8249579113843055*cos(x3) + (-1.649915822768611*cos(x1) + 1.4288690166235207*sin(x1))*sin(x3))*u1 + (-1.6499158227686117*cos(x3) - 1.6499158227686117*cos(x1)*sin(x3))*u2 + 0.8249579113843055*cos(x3)*u3 - 1.649915822768611*cos(x1)*sin(x3)*u3 - 1.4288690166235207*sin(x1)*sin(x3)*u3 - 0.68012*cos(2.*x1)*sin(x3)*x10*x2 - 0.12347999999999999*sin(x1)*x2^2 + 0.4858*cos(x3)*sin(2.*x1)*x4^2 + ((0.12347999999999999*sin(x1)*sin(x3) + 0.4858*sin(2.*x1)*sin(2.*x3))*x2 + (5.551115123125783^-17 - 0.12347999999999999*cos(x1)*cos(x3) + (-0.4858 - 0.4858*cos(2.*x1))*cos(2.*x3))*x4)*x6 - 0.68012*sin(2.*x1)*sin(x3)^2*x2*x8 + x4*(-0.34006*cos(x3)*sin(2.*x1)*x10 + (0.9716 + 0.9716*cos(2.*x1))*sin(x3)*x2 + (0.68012*cos(2.*x1)*cos(x3)*sin(x3) + 0.34006*sin(2*x3))*x8)) - 0.34006*(2.0940000000000003 - 0.7010000000000001*cos(2.*x1) + 0.0005*sin(2.*x1))*sin(2.*x1)*(0.12347999999999999*sin(x1) + 0.4858*cos(x3)*sin(2.*x1))*(-1.1102230246251565^-16*cos(x1)*cos(x3) - 1.4080000000000001*sin(x3))*sin(x3)*((0.8249579113843055*cos(x3) + (-1.649915822768611*cos(x1) + 1.4288690166235207*sin(x1))*sin(x3))*u1 + (-1.6499158227686117*cos(x3) - 1.6499158227686117*cos(x1)*sin(x3))*u2 + 0.8249579113843055*cos(x3)*u3 - 1.649915822768611*cos(x1)*sin(x3)*u3 - 1.4288690166235207*sin(x1)*sin(x3)*u3 - 0.68012*cos(2.*x1)*sin(x3)*x10*x2 - 0.12347999999999999*sin(x1)*x2^2 + 0.4858*cos(x3)*sin(2.*x1)*x4^2 + ((0.12347999999999999*sin(x1)*sin(x3) + 0.4858*sin(2.*x1)*sin(2.*x3))*x2 + (5.551115123125783^-17 - 0.12347999999999999*cos(x1)*cos(x3) + (-0.4858 - 0.4858*cos(2.*x1))*cos(2.*x3))*x4)*x6 - 0.68012*sin(2.*x1)*sin(x3)^2*x2*x8 + x4*(-0.34006*cos(x3)*sin(2.*x1)*x10 + (0.9716 + 0.9716*cos(2.*x1))*sin(x3)*x2 + (0.68012*cos(2.*x1)*cos(x3)*sin(x3) + 0.34006*sin(2*x3))*x8)) + (0.12348*cos(x1) - 0.9716*cos(x3))*(-0.9715999999999999*cos(x1)^2 + 0.12347999999999999*cos(x1)*cos(x3) - 1.9431999999999998*sin(x1)^2)*(0.12347999999999999*sin(x1) + 0.4858*cos(x3)*sin(2.*x1))*(cos(x3)*(-0.0005*cos(2.*x1) - 0.7010000000000001*sin(2.*x1)) - 1.1102230246251565^-16*sin(x1)*sin(x3))*((0.8249579113843055*cos(x3) + (-1.649915822768611*cos(x1) + 1.4288690166235207*sin(x1))*sin(x3))*u1 + (-1.6499158227686117*cos(x3) - 1.6499158227686117*cos(x1)*sin(x3))*u2 + 0.8249579113843055*cos(x3)*u3 - 1.649915822768611*cos(x1)*sin(x3)*u3 - 1.4288690166235207*sin(x1)*sin(x3)*u3 - 0.68012*cos(2.*x1)*sin(x3)*x10*x2 - 0.12347999999999999*sin(x1)*x2^2 + 0.4858*cos(x3)*sin(2.*x1)*x4^2 + ((0.12347999999999999*sin(x1)*sin(x3) + 0.4858*sin(2.*x1)*sin(2.*x3))*x2 + (5.551115123125783^-17 - 0.12347999999999999*cos(x1)*cos(x3) + (-0.4858 - 0.4858*cos(2.*x1))*cos(2.*x3))*x4)*x6 - 0.68012*sin(2.*x1)*sin(x3)^2*x2*x8 + x4*(-0.34006*cos(x3)*sin(2.*x1)*x10 + (0.9716 + 0.9716*cos(2.*x1))*sin(x3)*x2 + (0.68012*cos(2.*x1)*cos(x3)*sin(x3) + 0.34006*sin(2*x3))*x8)) - (1.0327336 - 0.34006*cos(2.*x1))*(0.12348*cos(x1) - 0.9716*cos(x3))*(cos(x3)*(-0.0005*cos(2.*x1) - 0.7010000000000001*sin(2.*x1)) - 1.1102230246251565^-16*sin(x1)*sin(x3))^2*((0.8249579113843055*cos(x3) + (-1.649915822768611*cos(x1) + 1.4288690166235207*sin(x1))*sin(x3))*u1 + (-1.6499158227686117*cos(x3) - 1.6499158227686117*cos(x1)*sin(x3))*u2 + 0.8249579113843055*cos(x3)*u3 - 1.649915822768611*cos(x1)*sin(x3)*u3 - 1.4288690166235207*sin(x1)*sin(x3)*u3 - 0.68012*cos(2.*x1)*sin(x3)*x10*x2 - 0.12347999999999999*sin(x1)*x2^2 + 0.4858*cos(x3)*sin(2.*x1)*x4^2 + ((0.12347999999999999*sin(x1)*sin(x3) + 0.4858*sin(2.*x1)*sin(2.*x3))*x2 + (5.551115123125783^-17 - 0.12347999999999999*cos(x1)*cos(x3) + (-0.4858 - 0.4858*cos(2.*x1))*cos(2.*x3))*x4)*x6 - 0.68012*sin(2.*x1)*sin(x3)^2*x2*x8 + x4*(-0.34006*cos(x3)*sin(2.*x1)*x10 + (0.9716 + 0.9716*cos(2.*x1))*sin(x3)*x2 + (0.68012*cos(2.*x1)*cos(x3)*sin(x3) + 0.34006*sin(2*x3))*x8)) + 0.041990608799999996*sin(x1)*sin(2.*x1)*sin(x3)^2*(cos(x3)*(-0.0005*cos(2.*x1) - 0.7010000000000001*sin(2.*x1)) - 1.1102230246251565^-16*sin(x1)*sin(x3))^2*((0.8249579113843055*cos(x3) + (-1.649915822768611*cos(x1) + 1.4288690166235207*sin(x1))*sin(x3))*u1 + (-1.6499158227686117*cos(x3) - 1.6499158227686117*cos(x1)*sin(x3))*u2 + 0.8249579113843055*cos(x3)*u3 - 1.649915822768611*cos(x1)*sin(x3)*u3 - 1.4288690166235207*sin(x1)*sin(x3)*u3 - 0.68012*cos(2.*x1)*sin(x3)*x10*x2 - 0.12347999999999999*sin(x1)*x2^2 + 0.4858*cos(x3)*sin(2.*x1)*x4^2 + ((0.12347999999999999*sin(x1)*sin(x3) + 0.4858*sin(2.*x1)*sin(2.*x3))*x2 + (5.551115123125783^-17 - 0.12347999999999999*cos(x1)*cos(x3) + (-0.4858 - 0.4858*cos(2.*x1))*cos(2.*x3))*x4)*x6 - 0.68012*sin(2.*x1)*sin(x3)^2*x2*x8 + x4*(-0.34006*cos(x3)*sin(2.*x1)*x10 + (0.9716 + 0.9716*cos(2.*x1))*sin(x3)*x2 + (0.68012*cos(2.*x1)*cos(x3)*sin(x3) + 0.34006*sin(2*x3))*x8)) + (1.0327336 - 0.34006*cos(2.*x1))*(0.12348*cos(x1) - 0.9716*cos(x3))*(2.0940000000000003 - 0.7010000000000001*cos(2.*x1) + 0.0005*sin(2.*x1))*((1.7510000000000001 + 2.1684043449710084^-19*0) + cos(2.*x1)*((0.3505 - 5.421010862427521^-20*0) + (0.3505 - 5.421010862427521^-20*0)*cos(2.*x3)) + cos(2.*x3)*(0.343 - (0.00025 - 2.8760394919088917^-17*0)*sin(2.*x1)) - (0.00025 - 2.8760394919088917^-17*0)*sin(2.*x1) + 1.1102230246251562^-16*cos(x1)*sin(2.*x3))*((0.8249579113843055*cos(x3) + (-1.649915822768611*cos(x1) + 1.4288690166235207*sin(x1))*sin(x3))*u1 + (-1.6499158227686117*cos(x3) - 1.6499158227686117*cos(x1)*sin(x3))*u2 + 0.8249579113843055*cos(x3)*u3 - 1.649915822768611*cos(x1)*sin(x3)*u3 - 1.4288690166235207*sin(x1)*sin(x3)*u3 - 0.68012*cos(2.*x1)*sin(x3)*x10*x2 - 0.12347999999999999*sin(x1)*x2^2 + 0.4858*cos(x3)*sin(2.*x1)*x4^2 + ((0.12347999999999999*sin(x1)*sin(x3) + 0.4858*sin(2.*x1)*sin(2.*x3))*x2 + (5.551115123125783^-17 - 0.12347999999999999*cos(x1)*cos(x3) + (-0.4858 - 0.4858*cos(2.*x1))*cos(2.*x3))*x4)*x6 - 0.68012*sin(2.*x1)*sin(x3)^2*x2*x8 + x4*(-0.34006*cos(x3)*sin(2.*x1)*x10 + (0.9716 + 0.9716*cos(2.*x1))*sin(x3)*x2 + (0.68012*cos(2.*x1)*cos(x3)*sin(x3) + 0.34006*sin(2*x3))*x8)) - 0.041990608799999996*sin(x1)*(2.0940000000000003 - 0.7010000000000001*cos(2.*x1) + 0.0005*sin(2.*x1))*sin(2.*x1)*sin(x3)^2*((1.7510000000000001 + 2.1684043449710084^-19*0) + cos(2.*x1)*((0.3505 - 5.421010862427521^-20*0) + (0.3505 - 5.421010862427521^-20*0)*cos(2.*x3)) + cos(2.*x3)*(0.343 - (0.00025 - 2.8760394919088917^-17*0)*sin(2.*x1)) - (0.00025 - 2.8760394919088917^-17*0)*sin(2.*x1) + 1.1102230246251562^-16*cos(x1)*sin(2.*x3))*((0.8249579113843055*cos(x3) + (-1.649915822768611*cos(x1) + 1.4288690166235207*sin(x1))*sin(x3))*u1 + (-1.6499158227686117*cos(x3) - 1.6499158227686117*cos(x1)*sin(x3))*u2 + 0.8249579113843055*cos(x3)*u3 - 1.649915822768611*cos(x1)*sin(x3)*u3 - 1.4288690166235207*sin(x1)*sin(x3)*u3 - 0.68012*cos(2.*x1)*sin(x3)*x10*x2 - 0.12347999999999999*sin(x1)*x2^2 + 0.4858*cos(x3)*sin(2.*x1)*x4^2 + ((0.12347999999999999*sin(x1)*sin(x3) + 0.4858*sin(2.*x1)*sin(2.*x3))*x2 + (5.551115123125783^-17 - 0.12347999999999999*cos(x1)*cos(x3) + (-0.4858 - 0.4858*cos(2.*x1))*cos(2.*x3))*x4)*x6 - 0.68012*sin(2.*x1)*sin(x3)^2*x2*x8 + x4*(-0.34006*cos(x3)*sin(2.*x1)*x10 + (0.9716 + 0.9716*cos(2.*x1))*sin(x3)*x2 + (0.68012*cos(2.*x1)*cos(x3)*sin(x3) + 0.34006*sin(2*x3))*x8)) - (1.0327336 - 0.34006*cos(2.*x1))*(2.0940000000000003 - 0.7010000000000001*cos(2.*x1) + 0.0005*sin(2.*x1))*(-1.1102230246251565^-16*cos(x1)*cos(x3) - 1.4080000000000001*sin(x3))*(-0.12347999999999999*cos(x1)*sin(x3) - (0.2429 + 2.7105054312137602^-20*0)*(1. + 1.*cos(2.*x1))*sin(2.*x3))*((0.8249579113843055*cos(x3) + (-1.649915822768611*cos(x1) + 1.4288690166235207*sin(x1))*sin(x3))*u1 + (-1.6499158227686117*cos(x3) - 1.6499158227686117*cos(x1)*sin(x3))*u2 + 0.8249579113843055*cos(x3)*u3 - 1.649915822768611*cos(x1)*sin(x3)*u3 - 1.4288690166235207*sin(x1)*sin(x3)*u3 - 0.68012*cos(2.*x1)*sin(x3)*x10*x2 - 0.12347999999999999*sin(x1)*x2^2 + 0.4858*cos(x3)*sin(2.*x1)*x4^2 + ((0.12347999999999999*sin(x1)*sin(x3) + 0.4858*sin(2.*x1)*sin(2.*x3))*x2 + (5.551115123125783^-17 - 0.12347999999999999*cos(x1)*cos(x3) + (-0.4858 - 0.4858*cos(2.*x1))*cos(2.*x3))*x4)*x6 - 0.68012*sin(2.*x1)*sin(x3)^2*x2*x8 + x4*(-0.34006*cos(x3)*sin(2.*x1)*x10 + (0.9716 + 0.9716*cos(2.*x1))*sin(x3)*x2 + (0.68012*cos(2.*x1)*cos(x3)*sin(x3) + 0.34006*sin(2*x3))*x8)) - 0.12348*(0.12347999999999999 + 0.9715999999999999*cos(x1)*cos(x3))*sin(x1)^2*(2.0940000000000003 - 0.7010000000000001*cos(2.*x1) + 0.0005*sin(2.*x1))*sin(x3)*(-0.12347999999999999*cos(x1)*sin(x3) - (0.2429 + 2.7105054312137602^-20*0)*(1. + 1.*cos(2.*x1))*sin(2.*x3))*((0.8249579113843055*cos(x3) + (-1.649915822768611*cos(x1) + 1.4288690166235207*sin(x1))*sin(x3))*u1 + (-1.6499158227686117*cos(x3) - 1.6499158227686117*cos(x1)*sin(x3))*u2 + 0.8249579113843055*cos(x3)*u3 - 1.649915822768611*cos(x1)*sin(x3)*u3 - 1.4288690166235207*sin(x1)*sin(x3)*u3 - 0.68012*cos(2.*x1)*sin(x3)*x10*x2 - 0.12347999999999999*sin(x1)*x2^2 + 0.4858*cos(x3)*sin(2.*x1)*x4^2 + ((0.12347999999999999*sin(x1)*sin(x3) + 0.4858*sin(2.*x1)*sin(2.*x3))*x2 + (5.551115123125783^-17 - 0.12347999999999999*cos(x1)*cos(x3) + (-0.4858 - 0.4858*cos(2.*x1))*cos(2.*x3))*x4)*x6 - 0.68012*sin(2.*x1)*sin(x3)^2*x2*x8 + x4*(-0.34006*cos(x3)*sin(2.*x1)*x10 + (0.9716 + 0.9716*cos(2.*x1))*sin(x3)*x2 + (0.68012*cos(2.*x1)*cos(x3)*sin(x3) + 0.34006*sin(2*x3))*x8)) + 0.12348*sin(x1)*(-0.9715999999999999*cos(x1)^2 + 0.12347999999999999*cos(x1)*cos(x3) - 1.9431999999999998*sin(x1)^2)*sin(x3)*(cos(x3)*(-0.0005*cos(2.*x1) - 0.7010000000000001*sin(2.*x1)) - 1.1102230246251565^-16*sin(x1)*sin(x3))*(-0.12347999999999999*cos(x1)*sin(x3) - (0.2429 + 2.7105054312137602^-20*0)*(1. + 1.*cos(2.*x1))*sin(2.*x3))*((0.8249579113843055*cos(x3) + (-1.649915822768611*cos(x1) + 1.4288690166235207*sin(x1))*sin(x3))*u1 + (-1.6499158227686117*cos(x3) - 1.6499158227686117*cos(x1)*sin(x3))*u2 + 0.8249579113843055*cos(x3)*u3 - 1.649915822768611*cos(x1)*sin(x3)*u3 - 1.4288690166235207*sin(x1)*sin(x3)*u3 - 0.68012*cos(2.*x1)*sin(x3)*x10*x2 - 0.12347999999999999*sin(x1)*x2^2 + 0.4858*cos(x3)*sin(2.*x1)*x4^2 + ((0.12347999999999999*sin(x1)*sin(x3) + 0.4858*sin(2.*x1)*sin(2.*x3))*x2 + (5.551115123125783^-17 - 0.12347999999999999*cos(x1)*cos(x3) + (-0.4858 - 0.4858*cos(2.*x1))*cos(2.*x3))*x4)*x6 - 0.68012*sin(2.*x1)*sin(x3)^2*x2*x8 + x4*(-0.34006*cos(x3)*sin(2.*x1)*x10 + (0.9716 + 0.9716*cos(2.*x1))*sin(x3)*x2 + (0.68012*cos(2.*x1)*cos(x3)*sin(x3) + 0.34006*sin(2*x3))*x8)) + (1.0327336 - 0.34006*cos(2.*x1))*(0.8627035999999999 + cos(2.*x1)*(0.17003 - 0.17003*cos(2.*x3)) - 0.17003*cos(2.*x3))*(2.0940000000000003 - 0.7010000000000001*cos(2.*x1) + 0.0005*sin(2.*x1))*(-1.1102230246251565^-16*cos(x1)*cos(x3) - 1.4080000000000001*sin(x3))*((cos(x3)*(0.942809041582063*cos(x1) - 0.8164965809277258*sin(x1)) + 0.4714045207910315*sin(x3))*u1 + (cos(x3)*(0.9428090415820635*cos(x1) + 0.6123724356957942*sin(x1)) - 2.0034692133618845*sin(x3))*u2 + (cos(x3)*(0.942809041582063*cos(x1) + 2.0412414523193148*sin(x1)) + 0.4714045207910315*sin(x3))*u3 + 1.1102230246251563^-16*cos(x3)*sin(x1)*x2^2 + (-1.1102230246251563^-16*cos(x3)*sin(x1) + (0.0004999999999999999*cos(2.*x1) + 0.701*sin(2.*x1))*sin(x3))*x4^2 + ((cos(2.*x1)*((-0.0004999999999999999 + 5.752078983817783^-17*0) - (0.0004999999999999999 - 5.752078983817783^-17*0)*cos(2.*x3)) - (0.701 - 1.0842021724855044^-19*0)*(1. + 1.*cos(2.*x3))*sin(2.*x1) - 1.110223024625156^-16*sin(x1)*sin(2.*x3))*x2 + (2.220446049250312^-16*cos(x1)*cos(2.*x3) + ((-0.6859999999999999 - 1.0842021724855043^-19*0) - (0.701 - 1.0842021724855044^-19*0)*cos(2.*x1) + (0.0004999999999999999 - 5.752078983817783^-17*0)*sin(2.*x1))*sin(2.*x3))*x4)*x6 + x4*(-0.4858*sin(2.*x1)*sin(x3)*x10 + cos(x3)*(-1.408 - 1.402*cos(2.*x1) + 0.0009999999999999998*sin(2.*x1))*x2 + (-0.12347999999999998*cos(x1)*cos(x3) + (-0.4858 - 0.4858*cos(2.*x1))*cos(2.*x3))*x8) + x2*((0.12347999999999996*cos(x1) + 0.9716*cos(2.*x1)*cos(x3))*x10 + (0.12347999999999996*sin(x1)*sin(x3) + 0.4858*sin(2*x1)*sin(2*x3))*x8)) + 0.12348*(0.12347999999999999 + 0.9715999999999999*cos(x1)*cos(x3))*(0.8627035999999999 + cos(2.*x1)*(0.17003 - 0.17003*cos(2.*x3)) - 0.17003*cos(2.*x3))*sin(x1)^2*(2.0940000000000003 - 0.7010000000000001*cos(2.*x1) + 0.0005*sin(2.*x1))*sin(x3)*((cos(x3)*(0.942809041582063*cos(x1) - 0.8164965809277258*sin(x1)) + 0.4714045207910315*sin(x3))*u1 + (cos(x3)*(0.9428090415820635*cos(x1) + 0.6123724356957942*sin(x1)) - 2.0034692133618845*sin(x3))*u2 + (cos(x3)*(0.942809041582063*cos(x1) + 2.0412414523193148*sin(x1)) + 0.4714045207910315*sin(x3))*u3 + 1.1102230246251563^-16*cos(x3)*sin(x1)*x2^2 + (-1.1102230246251563^-16*cos(x3)*sin(x1) + (0.0004999999999999999*cos(2.*x1) + 0.701*sin(2.*x1))*sin(x3))*x4^2 + ((cos(2.*x1)*((-0.0004999999999999999 + 5.752078983817783^-17*0) - (0.0004999999999999999 - 5.752078983817783^-17*0)*cos(2.*x3)) - (0.701 - 1.0842021724855044^-19*0)*(1. + 1.*cos(2.*x3))*sin(2.*x1) - 1.110223024625156^-16*sin(x1)*sin(2.*x3))*x2 + (2.220446049250312^-16*cos(x1)*cos(2.*x3) + ((-0.6859999999999999 - 1.0842021724855043^-19*0) - (0.701 - 1.0842021724855044^-19*0)*cos(2.*x1) + (0.0004999999999999999 - 5.752078983817783^-17*0)*sin(2.*x1))*sin(2.*x3))*x4)*x6 + x4*(-0.4858*sin(2.*x1)*sin(x3)*x10 + cos(x3)*(-1.408 - 1.402*cos(2.*x1) + 0.0009999999999999998*sin(2.*x1))*x2 + (-0.12347999999999998*cos(x1)*cos(x3) + (-0.4858 - 0.4858*cos(2.*x1))*cos(2.*x3))*x8) + x2*((0.12347999999999996*cos(x1) + 0.9716*cos(2.*x1)*cos(x3))*x10 + (0.12347999999999996*sin(x1)*sin(x3) + 0.4858*sin(2*x1)*sin(2*x3))*x8)) - 0.34006*(0.12348*cos(x1) - 0.9716*cos(x3))*(0.12347999999999999 + 0.9715999999999999*cos(x1)*cos(x3))*sin(x1)*(2.0940000000000003 - 0.7010000000000001*cos(2.*x1) + 0.0005*sin(2.*x1))*sin(2.*x1)*sin(x3)*((cos(x3)*(0.942809041582063*cos(x1) - 0.8164965809277258*sin(x1)) + 0.4714045207910315*sin(x3))*u1 + (cos(x3)*(0.9428090415820635*cos(x1) + 0.6123724356957942*sin(x1)) - 2.0034692133618845*sin(x3))*u2 + (cos(x3)*(0.942809041582063*cos(x1) + 2.0412414523193148*sin(x1)) + 0.4714045207910315*sin(x3))*u3 + 1.1102230246251563^-16*cos(x3)*sin(x1)*x2^2 + (-1.1102230246251563^-16*cos(x3)*sin(x1) + (0.0004999999999999999*cos(2.*x1) + 0.701*sin(2.*x1))*sin(x3))*x4^2 + ((cos(2.*x1)*((-0.0004999999999999999 + 5.752078983817783^-17*0) - (0.0004999999999999999 - 5.752078983817783^-17*0)*cos(2.*x3)) - (0.701 - 1.0842021724855044^-19*0)*(1. + 1.*cos(2.*x3))*sin(2.*x1) - 1.110223024625156^-16*sin(x1)*sin(2.*x3))*x2 + (2.220446049250312^-16*cos(x1)*cos(2.*x3) + ((-0.6859999999999999 - 1.0842021724855043^-19*0) - (0.701 - 1.0842021724855044^-19*0)*cos(2.*x1) + (0.0004999999999999999 - 5.752078983817783^-17*0)*sin(2.*x1))*sin(2.*x3))*x4)*x6 + x4*(-0.4858*sin(2.*x1)*sin(x3)*x10 + cos(x3)*(-1.408 - 1.402*cos(2.*x1) + 0.0009999999999999998*sin(2.*x1))*x2 + (-0.12347999999999998*cos(x1)*cos(x3) + (-0.4858 - 0.4858*cos(2.*x1))*cos(2.*x3))*x8) + x2*((0.12347999999999996*cos(x1) + 0.9716*cos(2.*x1)*cos(x3))*x10 + (0.12347999999999996*sin(x1)*sin(x3) + 0.4858*sin(2*x1)*sin(2*x3))*x8)) - 0.11564080359999998*(2.0940000000000003 - 0.7010000000000001*cos(2.*x1) + 0.0005*sin(2.*x1))*sin(2.*x1)^2*(-1.1102230246251565^-16*cos(x1)*cos(x3) - 1.4080000000000001*sin(x3))*sin(x3)^2*((cos(x3)*(0.942809041582063*cos(x1) - 0.8164965809277258*sin(x1)) + 0.4714045207910315*sin(x3))*u1 + (cos(x3)*(0.9428090415820635*cos(x1) + 0.6123724356957942*sin(x1)) - 2.0034692133618845*sin(x3))*u2 + (cos(x3)*(0.942809041582063*cos(x1) + 2.0412414523193148*sin(x1)) + 0.4714045207910315*sin(x3))*u3 + 1.1102230246251563^-16*cos(x3)*sin(x1)*x2^2 + (-1.1102230246251563^-16*cos(x3)*sin(x1) + (0.0004999999999999999*cos(2.*x1) + 0.701*sin(2.*x1))*sin(x3))*x4^2 + ((cos(2.*x1)*((-0.0004999999999999999 + 5.752078983817783^-17*0) - (0.0004999999999999999 - 5.752078983817783^-17*0)*cos(2.*x3)) - (0.701 - 1.0842021724855044^-19*0)*(1. + 1.*cos(2.*x3))*sin(2.*x1) - 1.110223024625156^-16*sin(x1)*sin(2.*x3))*x2 + (2.220446049250312^-16*cos(x1)*cos(2.*x3) + ((-0.6859999999999999 - 1.0842021724855043^-19*0) - (0.701 - 1.0842021724855044^-19*0)*cos(2.*x1) + (0.0004999999999999999 - 5.752078983817783^-17*0)*sin(2.*x1))*sin(2.*x3))*x4)*x6 + x4*(-0.4858*sin(2.*x1)*sin(x3)*x10 + cos(x3)*(-1.408 - 1.402*cos(2.*x1) + 0.0009999999999999998*sin(2.*x1))*x2 + (-0.12347999999999998*cos(x1)*cos(x3) + (-0.4858 - 0.4858*cos(2.*x1))*cos(2.*x3))*x8) + x2*((0.12347999999999996*cos(x1) + 0.9716*cos(2.*x1)*cos(x3))*x10 + (0.12347999999999996*sin(x1)*sin(x3) + 0.4858*sin(2*x1)*sin(2*x3))*x8)) - 0.12348*(0.8627035999999999 + cos(2.*x1)*(0.17003 - 0.17003*cos(2.*x3)) - 0.17003*cos(2.*x3))*sin(x1)*(-0.9715999999999999*cos(x1)^2 + 0.12347999999999999*cos(x1)*cos(x3) - 1.9431999999999998*sin(x1)^2)*sin(x3)*(cos(x3)*(-0.0005*cos(2.*x1) - 0.7010000000000001*sin(2.*x1)) - 1.1102230246251565^-16*sin(x1)*sin(x3))*((cos(x3)*(0.942809041582063*cos(x1) - 0.8164965809277258*sin(x1)) + 0.4714045207910315*sin(x3))*u1 + (cos(x3)*(0.9428090415820635*cos(x1) + 0.6123724356957942*sin(x1)) - 2.0034692133618845*sin(x3))*u2 + (cos(x3)*(0.942809041582063*cos(x1) + 2.0412414523193148*sin(x1)) + 0.4714045207910315*sin(x3))*u3 + 1.1102230246251563^-16*cos(x3)*sin(x1)*x2^2 + (-1.1102230246251563^-16*cos(x3)*sin(x1) + (0.0004999999999999999*cos(2.*x1) + 0.701*sin(2.*x1))*sin(x3))*x4^2 + ((cos(2.*x1)*((-0.0004999999999999999 + 5.752078983817783^-17*0) - (0.0004999999999999999 - 5.752078983817783^-17*0)*cos(2.*x3)) - (0.701 - 1.0842021724855044^-19*0)*(1. + 1.*cos(2.*x3))*sin(2.*x1) - 1.110223024625156^-16*sin(x1)*sin(2.*x3))*x2 + (2.220446049250312^-16*cos(x1)*cos(2.*x3) + ((-0.6859999999999999 - 1.0842021724855043^-19*0) - (0.701 - 1.0842021724855044^-19*0)*cos(2.*x1) + (0.0004999999999999999 - 5.752078983817783^-17*0)*sin(2.*x1))*sin(2.*x3))*x4)*x6 + x4*(-0.4858*sin(2.*x1)*sin(x3)*x10 + cos(x3)*(-1.408 - 1.402*cos(2.*x1) + 0.0009999999999999998*sin(2.*x1))*x2 + (-0.12347999999999998*cos(x1)*cos(x3) + (-0.4858 - 0.4858*cos(2.*x1))*cos(2.*x3))*x8) + x2*((0.12347999999999996*cos(x1) + 0.9716*cos(2.*x1)*cos(x3))*x10 + (0.12347999999999996*sin(x1)*sin(x3) + 0.4858*sin(2*x1)*sin(2*x3))*x8)) + 0.4858*(1.0327336 - 0.34006*cos(2.*x1))*(0.12348*cos(x1) - 0.9716*cos(x3))*sin(2.*x1)*sin(x3)*(cos(x3)*(-0.0005*cos(2.*x1) - 0.7010000000000001*sin(2.*x1)) - 1.1102230246251565^-16*sin(x1)*sin(x3))*((cos(x3)*(0.942809041582063*cos(x1) - 0.8164965809277258*sin(x1)) + 0.4714045207910315*sin(x3))*u1 + (cos(x3)*(0.9428090415820635*cos(x1) + 0.6123724356957942*sin(x1)) - 2.0034692133618845*sin(x3))*u2 + (cos(x3)*(0.942809041582063*cos(x1) + 2.0412414523193148*sin(x1)) + 0.4714045207910315*sin(x3))*u3 + 1.1102230246251563^-16*cos(x3)*sin(x1)*x2^2 + (-1.1102230246251563^-16*cos(x3)*sin(x1) + (0.0004999999999999999*cos(2.*x1) + 0.701*sin(2.*x1))*sin(x3))*x4^2 + ((cos(2.*x1)*((-0.0004999999999999999 + 5.752078983817783^-17*0) - (0.0004999999999999999 - 5.752078983817783^-17*0)*cos(2.*x3)) - (0.701 - 1.0842021724855044^-19*0)*(1. + 1.*cos(2.*x3))*sin(2.*x1) - 1.110223024625156^-16*sin(x1)*sin(2.*x3))*x2 + (2.220446049250312^-16*cos(x1)*cos(2.*x3) + ((-0.6859999999999999 - 1.0842021724855043^-19*0) - (0.701 - 1.0842021724855044^-19*0)*cos(2.*x1) + (0.0004999999999999999 - 5.752078983817783^-17*0)*sin(2.*x1))*sin(2.*x3))*x4)*x6 + x4*(-0.4858*sin(2.*x1)*sin(x3)*x10 + cos(x3)*(-1.408 - 1.402*cos(2.*x1) + 0.0009999999999999998*sin(2.*x1))*x2 + (-0.12347999999999998*cos(x1)*cos(x3) + (-0.4858 - 0.4858*cos(2.*x1))*cos(2.*x3))*x8) + x2*((0.12347999999999996*cos(x1) + 0.9716*cos(2.*x1)*cos(x3))*x10 + (0.12347999999999996*sin(x1)*sin(x3) + 0.4858*sin(2*x1)*sin(2*x3))*x8)) + 0.34006*(0.12348*cos(x1) - 0.9716*cos(x3))*(-0.9715999999999999*cos(x1)^2 + 0.12347999999999999*cos(x1)*cos(x3) - 1.9431999999999998*sin(x1)^2)*sin(2.*x1)*sin(x3)*(cos(x3)*(-0.0005*cos(2.*x1) - 0.7010000000000001*sin(2.*x1)) - 1.1102230246251565^-16*sin(x1)*sin(x3))*((cos(x3)*(0.942809041582063*cos(x1) - 0.8164965809277258*sin(x1)) + 0.4714045207910315*sin(x3))*u1 + (cos(x3)*(0.9428090415820635*cos(x1) + 0.6123724356957942*sin(x1)) - 2.0034692133618845*sin(x3))*u2 + (cos(x3)*(0.942809041582063*cos(x1) + 2.0412414523193148*sin(x1)) + 0.4714045207910315*sin(x3))*u3 + 1.1102230246251563^-16*cos(x3)*sin(x1)*x2^2 + (-1.1102230246251563^-16*cos(x3)*sin(x1) + (0.0004999999999999999*cos(2.*x1) + 0.701*sin(2.*x1))*sin(x3))*x4^2 + ((cos(2.*x1)*((-0.0004999999999999999 + 5.752078983817783^-17*0) - (0.0004999999999999999 - 5.752078983817783^-17*0)*cos(2.*x3)) - (0.701 - 1.0842021724855044^-19*0)*(1. + 1.*cos(2.*x3))*sin(2.*x1) - 1.110223024625156^-16*sin(x1)*sin(2.*x3))*x2 + (2.220446049250312^-16*cos(x1)*cos(2.*x3) + ((-0.6859999999999999 - 1.0842021724855043^-19*0) - (0.701 - 1.0842021724855044^-19*0)*cos(2.*x1) + (0.0004999999999999999 - 5.752078983817783^-17*0)*sin(2.*x1))*sin(2.*x3))*x4)*x6 + x4*(-0.4858*sin(2.*x1)*sin(x3)*x10 + cos(x3)*(-1.408 - 1.402*cos(2.*x1) + 0.0009999999999999998*sin(2.*x1))*x2 + (-0.12347999999999998*cos(x1)*cos(x3) + (-0.4858 - 0.4858*cos(2.*x1))*cos(2.*x3))*x8) + x2*((0.12347999999999996*cos(x1) + 0.9716*cos(2.*x1)*cos(x3))*x10 + (0.12347999999999996*sin(x1)*sin(x3) + 0.4858*sin(2*x1)*sin(2*x3))*x8)) - 0.020399037755039998*sin(x1)*sin(2.*x1)^2*sin(x3)^3*(cos(x3)*(-0.0005*cos(2.*x1) - 0.7010000000000001*sin(2.*x1)) - 1.1102230246251565^-16*sin(x1)*sin(x3))*((cos(x3)*(0.942809041582063*cos(x1) - 0.8164965809277258*sin(x1)) + 0.4714045207910315*sin(x3))*u1 + (cos(x3)*(0.9428090415820635*cos(x1) + 0.6123724356957942*sin(x1)) - 2.0034692133618845*sin(x3))*u2 + (cos(x3)*(0.942809041582063*cos(x1) + 2.0412414523193148*sin(x1)) + 0.4714045207910315*sin(x3))*u3 + 1.1102230246251563^-16*cos(x3)*sin(x1)*x2^2 + (-1.1102230246251563^-16*cos(x3)*sin(x1) + (0.0004999999999999999*cos(2.*x1) + 0.701*sin(2.*x1))*sin(x3))*x4^2 + ((cos(2.*x1)*((-0.0004999999999999999 + 5.752078983817783^-17*0) - (0.0004999999999999999 - 5.752078983817783^-17*0)*cos(2.*x3)) - (0.701 - 1.0842021724855044^-19*0)*(1. + 1.*cos(2.*x3))*sin(2.*x1) - 1.110223024625156^-16*sin(x1)*sin(2.*x3))*x2 + (2.220446049250312^-16*cos(x1)*cos(2.*x3) + ((-0.6859999999999999 - 1.0842021724855043^-19*0) - (0.701 - 1.0842021724855044^-19*0)*cos(2.*x1) + (0.0004999999999999999 - 5.752078983817783^-17*0)*sin(2.*x1))*sin(2.*x3))*x4)*x6 + x4*(-0.4858*sin(2.*x1)*sin(x3)*x10 + cos(x3)*(-1.408 - 1.402*cos(2.*x1) + 0.0009999999999999998*sin(2.*x1))*x2 + (-0.12347999999999998*cos(x1)*cos(x3) + (-0.4858 - 0.4858*cos(2.*x1))*cos(2.*x3))*x8) + x2*((0.12347999999999996*cos(x1) + 0.9716*cos(2.*x1)*cos(x3))*x10 + (0.12347999999999996*sin(x1)*sin(x3) + 0.4858*sin(2*x1)*sin(2*x3))*x8)) - (1.0327336 - 0.34006*cos(2.*x1))*(0.12348*cos(x1) - 0.9716*cos(x3))*(2.0940000000000003 - 0.7010000000000001*cos(2.*x1) + 0.0005*sin(2.*x1))*(-0.12347999999999999*cos(x1)*sin(x3) + (-0.24289999999999998 - 0.24289999999999998*cos(2.*x1))*sin(2.*x3))*((cos(x3)*(0.942809041582063*cos(x1) - 0.8164965809277258*sin(x1)) + 0.4714045207910315*sin(x3))*u1 + (cos(x3)*(0.9428090415820635*cos(x1) + 0.6123724356957942*sin(x1)) - 2.0034692133618845*sin(x3))*u2 + (cos(x3)*(0.942809041582063*cos(x1) + 2.0412414523193148*sin(x1)) + 0.4714045207910315*sin(x3))*u3 + 1.1102230246251563^-16*cos(x3)*sin(x1)*x2^2 + (-1.1102230246251563^-16*cos(x3)*sin(x1) + (0.0004999999999999999*cos(2.*x1) + 0.701*sin(2.*x1))*sin(x3))*x4^2 + ((cos(2.*x1)*((-0.0004999999999999999 + 5.752078983817783^-17*0) - (0.0004999999999999999 - 5.752078983817783^-17*0)*cos(2.*x3)) - (0.701 - 1.0842021724855044^-19*0)*(1. + 1.*cos(2.*x3))*sin(2.*x1) - 1.110223024625156^-16*sin(x1)*sin(2.*x3))*x2 + (2.220446049250312^-16*cos(x1)*cos(2.*x3) + ((-0.6859999999999999 - 1.0842021724855043^-19*0) - (0.701 - 1.0842021724855044^-19*0)*cos(2.*x1) + (0.0004999999999999999 - 5.752078983817783^-17*0)*sin(2.*x1))*sin(2.*x3))*x4)*x6 + x4*(-0.4858*sin(2.*x1)*sin(x3)*x10 + cos(x3)*(-1.408 - 1.402*cos(2.*x1) + 0.0009999999999999998*sin(2.*x1))*x2 + (-0.12347999999999998*cos(x1)*cos(x3) + (-0.4858 - 0.4858*cos(2.*x1))*cos(2.*x3))*x8) + x2*((0.12347999999999996*cos(x1) + 0.9716*cos(2.*x1)*cos(x3))*x10 + (0.12347999999999996*sin(x1)*sin(x3) + 0.4858*sin(2*x1)*sin(2*x3))*x8)) + 0.041990608799999996*sin(x1)*(2.0940000000000003 - 0.7010000000000001*cos(2.*x1) + 0.0005*sin(2.*x1))*sin(2.*x1)*sin(x3)^2*(-0.12347999999999999*cos(x1)*sin(x3) + (-0.24289999999999998 - 0.24289999999999998*cos(2.*x1))*sin(2.*x3))*((cos(x3)*(0.942809041582063*cos(x1) - 0.8164965809277258*sin(x1)) + 0.4714045207910315*sin(x3))*u1 + (cos(x3)*(0.9428090415820635*cos(x1) + 0.6123724356957942*sin(x1)) - 2.0034692133618845*sin(x3))*u2 + (cos(x3)*(0.942809041582063*cos(x1) + 2.0412414523193148*sin(x1)) + 0.4714045207910315*sin(x3))*u3 + 1.1102230246251563^-16*cos(x3)*sin(x1)*x2^2 + (-1.1102230246251563^-16*cos(x3)*sin(x1) + (0.0004999999999999999*cos(2.*x1) + 0.701*sin(2.*x1))*sin(x3))*x4^2 + ((cos(2.*x1)*((-0.0004999999999999999 + 5.752078983817783^-17*0) - (0.0004999999999999999 - 5.752078983817783^-17*0)*cos(2.*x3)) - (0.701 - 1.0842021724855044^-19*0)*(1. + 1.*cos(2.*x3))*sin(2.*x1) - 1.110223024625156^-16*sin(x1)*sin(2.*x3))*x2 + (2.220446049250312^-16*cos(x1)*cos(2.*x3) + ((-0.6859999999999999 - 1.0842021724855043^-19*0) - (0.701 - 1.0842021724855044^-19*0)*cos(2.*x1) + (0.0004999999999999999 - 5.752078983817783^-17*0)*sin(2.*x1))*sin(2.*x3))*x4)*x6 + x4*(-0.4858*sin(2.*x1)*sin(x3)*x10 + cos(x3)*(-1.408 - 1.402*cos(2.*x1) + 0.0009999999999999998*sin(2.*x1))*x2 + (-0.12347999999999998*cos(x1)*cos(x3) + (-0.4858 - 0.4858*cos(2.*x1))*cos(2.*x3))*x8) + x2*((0.12347999999999996*cos(x1) + 0.9716*cos(2.*x1)*cos(x3))*x10 + (0.12347999999999996*sin(x1)*sin(x3) + 0.4858*sin(2*x1)*sin(2*x3))*x8)) + (0.12347999999999999 + 0.9715999999999999*cos(x1)*cos(x3))*(0.8627035999999999 + cos(2.*x1)*(0.17003 - 0.17003*cos(2.*x3)) - 0.17003*cos(2.*x3))*sin(x1)*(2.0940000000000003 - 0.7010000000000001*cos(2.*x1) + 0.0005*sin(2.*x1))*(0.12347999999999999*sin(x1) + 0.4858*cos(x3)*sin(2.*x1))*(-17.30484*cos(x3)*sin(x1) - 0.47140452079103157*u1 + 2.003469213361885*u2 - 0.47140452079103157*u3 - 0.34006000000000003*sin(2.*x1)*x10^2 + ((-1.3877787807814455^-17*cos(x3)*sin(x1) + 0.9715999999999999*sin(2.*x1))*x10 - 1.1102230246251564^-16*cos(x1)*x2)*x4 + (-0.0005*cos(2.*x1) - 0.701*sin(2.*x1))*x4^2 + (0.0005*cos(x1)^2*cos(x3)^2 + 1.4019999999999997*cos(x1)*cos(x3)^2*sin(x1) + sin(x1)*(-0.0005*cos(x3)^2*sin(x1) + 5.551115123125783^-17*sin(2.*x3)))*x6^2 + sin(x3)*(cos(2.*x1)*(0.6801200000000001*x10 - 0.9715999999999999*x4) + 0.9715999999999999*x4)*x8 + 0.34006000000000003*sin(2.*x1)*sin(x3)^2*x8^2 + x6*((-0.12347999999999999*cos(x1) - 0.9715999999999999*cos(2.*x1)*cos(x3))*x10 + (cos(x3)*(-1.408 + 1.4019999999999997*cos(2*x1) - 0.001*sin(2*x1)) + 2.220446049250313^-16*cos(x1)*sin(x3))*x4 + (-0.12347999999999999*sin(x1)*sin(x3) - 0.48579999999999995*sin(2.*x1)*sin(2.*x3))*x8)) - (0.8627035999999999 + cos(2.*x1)*(0.17003 - 0.17003*cos(2.*x3)) - 0.17003*cos(2.*x3))*(-0.9715999999999999*cos(x1)^2 + 0.12347999999999999*cos(x1)*cos(x3) - 1.9431999999999998*sin(x1)^2)*(0.12347999999999999*sin(x1) + 0.4858*cos(x3)*sin(2.*x1))*(cos(x3)*(-0.0005*cos(2.*x1) - 0.7010000000000001*sin(2.*x1)) - 1.1102230246251565^-16*sin(x1)*sin(x3))*(-17.30484*cos(x3)*sin(x1) - 0.47140452079103157*u1 + 2.003469213361885*u2 - 0.47140452079103157*u3 - 0.34006000000000003*sin(2.*x1)*x10^2 + ((-1.3877787807814455^-17*cos(x3)*sin(x1) + 0.9715999999999999*sin(2.*x1))*x10 - 1.1102230246251564^-16*cos(x1)*x2)*x4 + (-0.0005*cos(2.*x1) - 0.701*sin(2.*x1))*x4^2 + (0.0005*cos(x1)^2*cos(x3)^2 + 1.4019999999999997*cos(x1)*cos(x3)^2*sin(x1) + sin(x1)*(-0.0005*cos(x3)^2*sin(x1) + 5.551115123125783^-17*sin(2.*x3)))*x6^2 + sin(x3)*(cos(2.*x1)*(0.6801200000000001*x10 - 0.9715999999999999*x4) + 0.9715999999999999*x4)*x8 + 0.34006000000000003*sin(2.*x1)*sin(x3)^2*x8^2 + x6*((-0.12347999999999999*cos(x1) - 0.9715999999999999*cos(2.*x1)*cos(x3))*x10 + (cos(x3)*(-1.408 + 1.4019999999999997*cos(2*x1) - 0.001*sin(2*x1)) + 2.220446049250313^-16*cos(x1)*sin(x3))*x4 + (-0.12347999999999999*sin(x1)*sin(x3) - 0.48579999999999995*sin(2.*x1)*sin(2.*x3))*x8)) - 0.165201148*sin(2.*x1)^2*(0.12347999999999999*sin(x1) + 0.4858*cos(x3)*sin(2.*x1))*sin(x3)^2*(cos(x3)*(-0.0005*cos(2.*x1) - 0.7010000000000001*sin(2.*x1)) - 1.1102230246251565^-16*sin(x1)*sin(x3))*(-17.30484*cos(x3)*sin(x1) - 0.47140452079103157*u1 + 2.003469213361885*u2 - 0.47140452079103157*u3 - 0.34006000000000003*sin(2.*x1)*x10^2 + ((-1.3877787807814455^-17*cos(x3)*sin(x1) + 0.9715999999999999*sin(2.*x1))*x10 - 1.1102230246251564^-16*cos(x1)*x2)*x4 + (-0.0005*cos(2.*x1) - 0.701*sin(2.*x1))*x4^2 + (0.0005*cos(x1)^2*cos(x3)^2 + 1.4019999999999997*cos(x1)*cos(x3)^2*sin(x1) + sin(x1)*(-0.0005*cos(x3)^2*sin(x1) + 5.551115123125783^-17*sin(2.*x3)))*x6^2 + sin(x3)*(cos(2.*x1)*(0.6801200000000001*x10 - 0.9715999999999999*x4) + 0.9715999999999999*x4)*x8 + 0.34006000000000003*sin(2.*x1)*sin(x3)^2*x8^2 + x6*((-0.12347999999999999*cos(x1) - 0.9715999999999999*cos(2.*x1)*cos(x3))*x10 + (cos(x3)*(-1.408 + 1.4019999999999997*cos(2*x1) - 0.001*sin(2*x1)) + 2.220446049250313^-16*cos(x1)*sin(x3))*x4 + (-0.12347999999999999*sin(x1)*sin(x3) - 0.48579999999999995*sin(2.*x1)*sin(2.*x3))*x8)) + (1.0327336 - 0.34006*cos(2.*x1))*(0.8627035999999999 + cos(2.*x1)*(0.17003 - 0.17003*cos(2.*x3)) - 0.17003*cos(2.*x3))*(cos(x3)*(-0.0005*cos(2.*x1) - 0.7010000000000001*sin(2.*x1)) - 1.1102230246251565^-16*sin(x1)*sin(x3))^2*(-17.30484*cos(x3)*sin(x1) - 0.47140452079103157*u1 + 2.003469213361885*u2 - 0.47140452079103157*u3 - 0.34006000000000003*sin(2.*x1)*x10^2 + ((-1.3877787807814455^-17*cos(x3)*sin(x1) + 0.9715999999999999*sin(2.*x1))*x10 - 1.1102230246251564^-16*cos(x1)*x2)*x4 + (-0.0005*cos(2.*x1) - 0.701*sin(2.*x1))*x4^2 + (0.0005*cos(x1)^2*cos(x3)^2 + 1.4019999999999997*cos(x1)*cos(x3)^2*sin(x1) + sin(x1)*(-0.0005*cos(x3)^2*sin(x1) + 5.551115123125783^-17*sin(2.*x3)))*x6^2 + sin(x3)*(cos(2.*x1)*(0.6801200000000001*x10 - 0.9715999999999999*x4) + 0.9715999999999999*x4)*x8 + 0.34006000000000003*sin(2.*x1)*sin(x3)^2*x8^2 + x6*((-0.12347999999999999*cos(x1) - 0.9715999999999999*cos(2.*x1)*cos(x3))*x10 + (cos(x3)*(-1.408 + 1.4019999999999997*cos(2*x1) - 0.001*sin(2*x1)) + 2.220446049250313^-16*cos(x1)*sin(x3))*x4 + (-0.12347999999999999*sin(x1)*sin(x3) - 0.48579999999999995*sin(2.*x1)*sin(2.*x3))*x8)) - 0.11564080359999998*sin(2.*x1)^2*sin(x3)^2*(cos(x3)*(-0.0005*cos(2.*x1) - 0.7010000000000001*sin(2.*x1)) - 1.1102230246251565^-16*sin(x1)*sin(x3))^2*(-17.30484*cos(x3)*sin(x1) - 0.47140452079103157*u1 + 2.003469213361885*u2 - 0.47140452079103157*u3 - 0.34006000000000003*sin(2.*x1)*x10^2 + ((-1.3877787807814455^-17*cos(x3)*sin(x1) + 0.9715999999999999*sin(2.*x1))*x10 - 1.1102230246251564^-16*cos(x1)*x2)*x4 + (-0.0005*cos(2.*x1) - 0.701*sin(2.*x1))*x4^2 + (0.0005*cos(x1)^2*cos(x3)^2 + 1.4019999999999997*cos(x1)*cos(x3)^2*sin(x1) + sin(x1)*(-0.0005*cos(x3)^2*sin(x1) + 5.551115123125783^-17*sin(2.*x3)))*x6^2 + sin(x3)*(cos(2.*x1)*(0.6801200000000001*x10 - 0.9715999999999999*x4) + 0.9715999999999999*x4)*x8 + 0.34006000000000003*sin(2.*x1)*sin(x3)^2*x8^2 + x6*((-0.12347999999999999*cos(x1) - 0.9715999999999999*cos(2.*x1)*cos(x3))*x10 + (cos(x3)*(-1.408 + 1.4019999999999997*cos(2*x1) - 0.001*sin(2*x1)) + 2.220446049250313^-16*cos(x1)*sin(x3))*x4 + (-0.12347999999999999*sin(x1)*sin(x3) - 0.48579999999999995*sin(2.*x1)*sin(2.*x3))*x8)) - (1.0327336 - 0.34006*cos(2.*x1))*(0.8627035999999999 + cos(2.*x1)*(0.17003 - 0.17003*cos(2.*x3)) - 0.17003*cos(2.*x3))*(2.0940000000000003 - 0.7010000000000001*cos(2.*x1) + 0.0005*sin(2.*x1))*((1.7510000000000001 + 2.1684043449710084^-19*0) + cos(2.*x1)*((0.3505 - 5.421010862427521^-20*0) + (0.3505 - 5.421010862427521^-20*0)*cos(2.*x3)) + cos(2.*x3)*(0.343 - (0.00025 - 2.8760394919088917^-17*0)*sin(2.*x1)) - (0.00025 - 2.8760394919088917^-17*0)*sin(2.*x1) + 1.1102230246251562^-16*cos(x1)*sin(2.*x3))*(-17.30484*cos(x3)*sin(x1) - 0.47140452079103157*u1 + 2.003469213361885*u2 - 0.47140452079103157*u3 - 0.34006000000000003*sin(2.*x1)*x10^2 + ((-1.3877787807814455^-17*cos(x3)*sin(x1) + 0.9715999999999999*sin(2.*x1))*x10 - 1.1102230246251564^-16*cos(x1)*x2)*x4 + (-0.0005*cos(2.*x1) - 0.701*sin(2.*x1))*x4^2 + (0.0005*cos(x1)^2*cos(x3)^2 + 1.4019999999999997*cos(x1)*cos(x3)^2*sin(x1) + sin(x1)*(-0.0005*cos(x3)^2*sin(x1) + 5.551115123125783^-17*sin(2.*x3)))*x6^2 + sin(x3)*(cos(2.*x1)*(0.6801200000000001*x10 - 0.9715999999999999*x4) + 0.9715999999999999*x4)*x8 + 0.34006000000000003*sin(2.*x1)*sin(x3)^2*x8^2 + x6*((-0.12347999999999999*cos(x1) - 0.9715999999999999*cos(2.*x1)*cos(x3))*x10 + (cos(x3)*(-1.408 + 1.4019999999999997*cos(2*x1) - 0.001*sin(2*x1)) + 2.220446049250313^-16*cos(x1)*sin(x3))*x4 + (-0.12347999999999999*sin(x1)*sin(x3) - 0.48579999999999995*sin(2.*x1)*sin(2.*x3))*x8)) + 0.11564080359999998*(2.0940000000000003 - 0.7010000000000001*cos(2.*x1) + 0.0005*sin(2.*x1))*sin(2.*x1)^2*sin(x3)^2*((1.7510000000000001 + 2.1684043449710084^-19*0) + cos(2.*x1)*((0.3505 - 5.421010862427521^-20*0) + (0.3505 - 5.421010862427521^-20*0)*cos(2.*x3)) + cos(2.*x3)*(0.343 - (0.00025 - 2.8760394919088917^-17*0)*sin(2.*x1)) - (0.00025 - 2.8760394919088917^-17*0)*sin(2.*x1) + 1.1102230246251562^-16*cos(x1)*sin(2.*x3))*(-17.30484*cos(x3)*sin(x1) - 0.47140452079103157*u1 + 2.003469213361885*u2 - 0.47140452079103157*u3 - 0.34006000000000003*sin(2.*x1)*x10^2 + ((-1.3877787807814455^-17*cos(x3)*sin(x1) + 0.9715999999999999*sin(2.*x1))*x10 - 1.1102230246251564^-16*cos(x1)*x2)*x4 + (-0.0005*cos(2.*x1) - 0.701*sin(2.*x1))*x4^2 + (0.0005*cos(x1)^2*cos(x3)^2 + 1.4019999999999997*cos(x1)*cos(x3)^2*sin(x1) + sin(x1)*(-0.0005*cos(x3)^2*sin(x1) + 5.551115123125783^-17*sin(2.*x3)))*x6^2 + sin(x3)*(cos(2.*x1)*(0.6801200000000001*x10 - 0.9715999999999999*x4) + 0.9715999999999999*x4)*x8 + 0.34006000000000003*sin(2.*x1)*sin(x3)^2*x8^2 + x6*((-0.12347999999999999*cos(x1) - 0.9715999999999999*cos(2.*x1)*cos(x3))*x10 + (cos(x3)*(-1.408 + 1.4019999999999997*cos(2*x1) - 0.001*sin(2*x1)) + 2.220446049250313^-16*cos(x1)*sin(x3))*x4 + (-0.12347999999999999*sin(x1)*sin(x3) - 0.48579999999999995*sin(2.*x1)*sin(2.*x3))*x8)) + 0.34006*(2.0940000000000003 - 0.7010000000000001*cos(2.*x1) + 0.0005*sin(2.*x1))*sin(2.*x1)*(0.12347999999999999*sin(x1) + 0.4858*cos(x3)*sin(2.*x1))*sin(x3)*(-0.12347999999999999*cos(x1)*sin(x3) + (-0.24289999999999998 - 0.24289999999999998*cos(2.*x1))*sin(2.*x3))*(-17.30484*cos(x3)*sin(x1) - 0.47140452079103157*u1 + 2.003469213361885*u2 - 0.47140452079103157*u3 - 0.34006000000000003*sin(2.*x1)*x10^2 + ((-1.3877787807814455^-17*cos(x3)*sin(x1) + 0.9715999999999999*sin(2.*x1))*x10 - 1.1102230246251564^-16*cos(x1)*x2)*x4 + (-0.0005*cos(2.*x1) - 0.701*sin(2.*x1))*x4^2 + (0.0005*cos(x1)^2*cos(x3)^2 + 1.4019999999999997*cos(x1)*cos(x3)^2*sin(x1) + sin(x1)*(-0.0005*cos(x3)^2*sin(x1) + 5.551115123125783^-17*sin(2.*x3)))*x6^2 + sin(x3)*(cos(2.*x1)*(0.6801200000000001*x10 - 0.9715999999999999*x4) + 0.9715999999999999*x4)*x8 + 0.34006000000000003*sin(2.*x1)*sin(x3)^2*x8^2 + x6*((-0.12347999999999999*cos(x1) - 0.9715999999999999*cos(2.*x1)*cos(x3))*x10 + (cos(x3)*(-1.408 + 1.4019999999999997*cos(2*x1) - 0.001*sin(2*x1)) + 2.220446049250313^-16*cos(x1)*sin(x3))*x4 + (-0.12347999999999999*sin(x1)*sin(x3) - 0.48579999999999995*sin(2.*x1)*sin(2.*x3))*x8)) + 0.34006*(0.12347999999999999 + 0.9715999999999999*cos(x1)*cos(x3))*sin(x1)*(2.0940000000000003 - 0.7010000000000001*cos(2.*x1) + 0.0005*sin(2.*x1))*sin(2.*x1)*sin(x3)*(-0.12347999999999999*cos(x1)*sin(x3) - (0.2429 + 2.7105054312137602^-20*0)*(1. + 1.*cos(2.*x1))*sin(2.*x3))*(-17.30484*cos(x3)*sin(x1) - 0.47140452079103157*u1 + 2.003469213361885*u2 - 0.47140452079103157*u3 - 0.34006000000000003*sin(2.*x1)*x10^2 + ((-1.3877787807814455^-17*cos(x3)*sin(x1) + 0.9715999999999999*sin(2.*x1))*x10 - 1.1102230246251564^-16*cos(x1)*x2)*x4 + (-0.0005*cos(2.*x1) - 0.701*sin(2.*x1))*x4^2 + (0.0005*cos(x1)^2*cos(x3)^2 + 1.4019999999999997*cos(x1)*cos(x3)^2*sin(x1) + sin(x1)*(-0.0005*cos(x3)^2*sin(x1) + 5.551115123125783^-17*sin(2.*x3)))*x6^2 + sin(x3)*(cos(2.*x1)*(0.6801200000000001*x10 - 0.9715999999999999*x4) + 0.9715999999999999*x4)*x8 + 0.34006000000000003*sin(2.*x1)*sin(x3)^2*x8^2 + x6*((-0.12347999999999999*cos(x1) - 0.9715999999999999*cos(2.*x1)*cos(x3))*x10 + (cos(x3)*(-1.408 + 1.4019999999999997*cos(2*x1) - 0.001*sin(2*x1)) + 2.220446049250313^-16*cos(x1)*sin(x3))*x4 + (-0.12347999999999999*sin(x1)*sin(x3) - 0.48579999999999995*sin(2.*x1)*sin(2.*x3))*x8)) - 0.4858*(1.0327336 - 0.34006*cos(2.*x1))*sin(2.*x1)*sin(x3)*(cos(x3)*(-0.0005*cos(2.*x1) - 0.7010000000000001*sin(2.*x1)) - 1.1102230246251565^-16*sin(x1)*sin(x3))*(-0.12347999999999999*cos(x1)*sin(x3) - (0.2429 + 2.7105054312137602^-20*0)*(1. + 1.*cos(2.*x1))*sin(2.*x3))*(-17.30484*cos(x3)*sin(x1) - 0.47140452079103157*u1 + 2.003469213361885*u2 - 0.47140452079103157*u3 - 0.34006000000000003*sin(2.*x1)*x10^2 + ((-1.3877787807814455^-17*cos(x3)*sin(x1) + 0.9715999999999999*sin(2.*x1))*x10 - 1.1102230246251564^-16*cos(x1)*x2)*x4 + (-0.0005*cos(2.*x1) - 0.701*sin(2.*x1))*x4^2 + (0.0005*cos(x1)^2*cos(x3)^2 + 1.4019999999999997*cos(x1)*cos(x3)^2*sin(x1) + sin(x1)*(-0.0005*cos(x3)^2*sin(x1) + 5.551115123125783^-17*sin(2.*x3)))*x6^2 + sin(x3)*(cos(2.*x1)*(0.6801200000000001*x10 - 0.9715999999999999*x4) + 0.9715999999999999*x4)*x8 + 0.34006000000000003*sin(2.*x1)*sin(x3)^2*x8^2 + x6*((-0.12347999999999999*cos(x1) - 0.9715999999999999*cos(2.*x1)*cos(x3))*x10 + (cos(x3)*(-1.408 + 1.4019999999999997*cos(2*x1) - 0.001*sin(2*x1)) + 2.220446049250313^-16*cos(x1)*sin(x3))*x4 + (-0.12347999999999999*sin(x1)*sin(x3) - 0.48579999999999995*sin(2.*x1)*sin(2.*x3))*x8)) - 0.34006*(-0.9715999999999999*cos(x1)^2 + 0.12347999999999999*cos(x1)*cos(x3) - 1.9431999999999998*sin(x1)^2)*sin(2.*x1)*sin(x3)*(cos(x3)*(-0.0005*cos(2.*x1) - 0.7010000000000001*sin(2.*x1)) - 1.1102230246251565^-16*sin(x1)*sin(x3))*(-0.12347999999999999*cos(x1)*sin(x3) - (0.2429 + 2.7105054312137602^-20*0)*(1. + 1.*cos(2.*x1))*sin(2.*x3))*(-17.30484*cos(x3)*sin(x1) - 0.47140452079103157*u1 + 2.003469213361885*u2 - 0.47140452079103157*u3 - 0.34006000000000003*sin(2.*x1)*x10^2 + ((-1.3877787807814455^-17*cos(x3)*sin(x1) + 0.9715999999999999*sin(2.*x1))*x10 - 1.1102230246251564^-16*cos(x1)*x2)*x4 + (-0.0005*cos(2.*x1) - 0.701*sin(2.*x1))*x4^2 + (0.0005*cos(x1)^2*cos(x3)^2 + 1.4019999999999997*cos(x1)*cos(x3)^2*sin(x1) + sin(x1)*(-0.0005*cos(x3)^2*sin(x1) + 5.551115123125783^-17*sin(2.*x3)))*x6^2 + sin(x3)*(cos(2.*x1)*(0.6801200000000001*x10 - 0.9715999999999999*x4) + 0.9715999999999999*x4)*x8 + 0.34006000000000003*sin(2.*x1)*sin(x3)^2*x8^2 + x6*((-0.12347999999999999*cos(x1) - 0.9715999999999999*cos(2.*x1)*cos(x3))*x10 + (cos(x3)*(-1.408 + 1.4019999999999997*cos(2*x1) - 0.001*sin(2*x1)) + 2.220446049250313^-16*cos(x1)*sin(x3))*x4 + (-0.12347999999999999*sin(x1)*sin(x3) - 0.48579999999999995*sin(2.*x1)*sin(2.*x3))*x8)) + (1.0327336 - 0.34006*cos(2.*x1))*(2.0940000000000003 - 0.7010000000000001*cos(2.*x1) + 0.0005*sin(2.*x1))*(-0.12347999999999999*cos(x1)*sin(x3) + (-0.24289999999999998 - 0.24289999999999998*cos(2.*x1))*sin(2.*x3))*(-0.12347999999999999*cos(x1)*sin(x3) - (0.2429 + 2.7105054312137602^-20*0)*(1. + 1.*cos(2.*x1))*sin(2.*x3))*(-17.30484*cos(x3)*sin(x1) - 0.47140452079103157*u1 + 2.003469213361885*u2 - 0.47140452079103157*u3 - 0.34006000000000003*sin(2.*x1)*x10^2 + ((-1.3877787807814455^-17*cos(x3)*sin(x1) + 0.9715999999999999*sin(2.*x1))*x10 - 1.1102230246251564^-16*cos(x1)*x2)*x4 + (-0.0005*cos(2.*x1) - 0.701*sin(2.*x1))*x4^2 + (0.0005*cos(x1)^2*cos(x3)^2 + 1.4019999999999997*cos(x1)*cos(x3)^2*sin(x1) + sin(x1)*(-0.0005*cos(x3)^2*sin(x1) + 5.551115123125783^-17*sin(2.*x3)))*x6^2 + sin(x3)*(cos(2.*x1)*(0.6801200000000001*x10 - 0.9715999999999999*x4) + 0.9715999999999999*x4)*x8 + 0.34006000000000003*sin(2.*x1)*sin(x3)^2*x8^2 + x6*((-0.12347999999999999*cos(x1) - 0.9715999999999999*cos(2.*x1)*cos(x3))*x10 + (cos(x3)*(-1.408 + 1.4019999999999997*cos(2*x1) - 0.001*sin(2*x1)) + 2.220446049250313^-16*cos(x1)*sin(x3))*x4 + (-0.12347999999999999*sin(x1)*sin(x3) - 0.48579999999999995*sin(2.*x1)*sin(2.*x3))*x8)) + (-1.4574 + 0.4858*cos(2.*x1) + 0.12348*cos(x1)*cos(x3))*(0. + (0.8627035999999999 + cos(2.*x1)*(0.17003 - 0.17003*cos(2.*x3)) - 0.17003*cos(2.*x3))*(-1.1102230246251565^-16*cos(x1)*cos(x3) - 1.4080000000000001*sin(x3))*(cos(x3)*(-0.0005*cos(2.*x1) - 0.701*sin(2.*x1)) - 1.1102230246251564^-16*sin(x1)*sin(x3))*((1.4288690166235203*cos(x1) + 1.6499158227686102*sin(x1))*u1 + 1.6499158227686104*sin(x1)*u2 + 1.6499158227686102*sin(x1)*u3 + 0.68012*sin(2.*x1)*x10*x2 + cos(x1)*(-1.4288690166235203*u3 - 0.12348*sin(x3)*x2^2) - 0.24696*cos(x3)*sin(x1)*x2*x4 - 0.9716000000000001*sin(2.*x1)*x2*x4 - 0.12348*cos(x1)*sin(x3)*x4^2 + ((0.12347999999999998*cos(x1) + 0.9716*cos(x1)^2*cos(x3) - 0.9716*cos(x3)*sin(x1)^2)*x2 - 0.4858*sin(2*x1)*sin(x3)*x4)*x6 + (-0.68012*cos(2.*x1)*sin(x3)*x2 - 0.34006*cos(x3)*sin(2.*x1)*x4)*x8) - (0.12348*cos(x1) - 0.9716*cos(x3))*(cos(x3)*(-0.0005*cos(2.*x1) - 0.701*sin(2.*x1)) - 1.1102230246251564^-16*sin(x1)*sin(x3))*(-0.12347999999999999*cos(x1)*sin(x3) + (-0.24289999999999998 - 0.24289999999999998*cos(2.*x1))*sin(2.*x3))*((1.4288690166235203*cos(x1) + 1.6499158227686102*sin(x1))*u1 + 1.6499158227686104*sin(x1)*u2 + 1.6499158227686102*sin(x1)*u3 + 0.68012*sin(2.*x1)*x10*x2 + cos(x1)*(-1.4288690166235203*u3 - 0.12348*sin(x3)*x2^2) - 0.24696*cos(x3)*sin(x1)*x2*x4 - 0.9716000000000001*sin(2.*x1)*x2*x4 - 0.12348*cos(x1)*sin(x3)*x4^2 + ((0.12347999999999998*cos(x1) + 0.9716*cos(x1)^2*cos(x3) - 0.9716*cos(x3)*sin(x1)^2)*x2 - 0.4858*sin(2*x1)*sin(x3)*x4)*x6 + (-0.68012*cos(2.*x1)*sin(x3)*x2 - 0.34006*cos(x3)*sin(2.*x1)*x4)*x8) + (0.12348*cos(x1) - 0.9716*cos(x3))*(0.12347999999999999 + 0.9715999999999999*cos(x1)*cos(x3))*sin(x1)*(cos(x3)*(-0.0005*cos(2.*x1) - 0.701*sin(2.*x1)) - 1.1102230246251564^-16*sin(x1)*sin(x3))*((0.8249579113843055*cos(x3) + (-1.649915822768611*cos(x1) + 1.4288690166235207*sin(x1))*sin(x3))*u1 + (-1.6499158227686117*cos(x3) - 1.6499158227686117*cos(x1)*sin(x3))*u2 + 0.8249579113843055*cos(x3)*u3 - 1.649915822768611*cos(x1)*sin(x3)*u3 - 1.4288690166235207*sin(x1)*sin(x3)*u3 - 0.68012*cos(2.*x1)*sin(x3)*x10*x2 - 0.12347999999999999*sin(x1)*x2^2 + 0.4858*cos(x3)*sin(2.*x1)*x4^2 + ((0.12347999999999999*sin(x1)*sin(x3) + 0.4858*sin(2.*x1)*sin(2.*x3))*x2 + (5.551115123125783^-17 - 0.12347999999999999*cos(x1)*cos(x3) + (-0.4858 - 0.4858*cos(2.*x1))*cos(2.*x3))*x4)*x6 - 0.68012*sin(2.*x1)*sin(x3)^2*x2*x8 + x4*(-0.34006*cos(x3)*sin(2.*x1)*x10 + (0.9716 + 0.9716*cos(2.*x1))*sin(x3)*x2 + (0.68012*cos(2.*x1)*cos(x3)*sin(x3) + 0.34006*sin(2*x3))*x8)) + 0.34006*sin(2.*x1)*(-1.1102230246251565^-16*cos(x1)*cos(x3) - 1.4080000000000001*sin(x3))*sin(x3)*(cos(x3)*(-0.0005*cos(2.*x1) - 0.701*sin(2.*x1)) - 1.1102230246251564^-16*sin(x1)*sin(x3))*((0.8249579113843055*cos(x3) + (-1.649915822768611*cos(x1) + 1.4288690166235207*sin(x1))*sin(x3))*u1 + (-1.6499158227686117*cos(x3) - 1.6499158227686117*cos(x1)*sin(x3))*u2 + 0.8249579113843055*cos(x3)*u3 - 1.649915822768611*cos(x1)*sin(x3)*u3 - 1.4288690166235207*sin(x1)*sin(x3)*u3 - 0.68012*cos(2.*x1)*sin(x3)*x10*x2 - 0.12347999999999999*sin(x1)*x2^2 + 0.4858*cos(x3)*sin(2.*x1)*x4^2 + ((0.12347999999999999*sin(x1)*sin(x3) + 0.4858*sin(2.*x1)*sin(2.*x3))*x2 + (5.551115123125783^-17 - 0.12347999999999999*cos(x1)*cos(x3) + (-0.4858 - 0.4858*cos(2.*x1))*cos(2.*x3))*x4)*x6 - 0.68012*sin(2.*x1)*sin(x3)^2*x2*x8 + x4*(-0.34006*cos(x3)*sin(2.*x1)*x10 + (0.9716 + 0.9716*cos(2.*x1))*sin(x3)*x2 + (0.68012*cos(2.*x1)*cos(x3)*sin(x3) + 0.34006*sin(2*x3))*x8)) - (0.8627035999999999 + cos(2.*x1)*(0.17003 - 0.17003*cos(2.*x3)) - 0.17003*cos(2.*x3))*(-0.9715999999999999*cos(x1)^2 + 0.12347999999999999*cos(x1)*cos(x3) - 1.9431999999999998*sin(x1)^2)*(-1.1102230246251565^-16*cos(x1)*cos(x3) - 1.4080000000000001*sin(x3))*((cos(x3)*(0.942809041582063*cos(x1) - 0.8164965809277258*sin(x1)) + 0.4714045207910315*sin(x3))*u1 + (cos(x3)*(0.9428090415820635*cos(x1) + 0.6123724356957942*sin(x1)) - 2.0034692133618845*sin(x3))*u2 + (cos(x3)*(0.942809041582063*cos(x1) + 2.0412414523193148*sin(x1)) + 0.4714045207910315*sin(x3))*u3 + 1.1102230246251563^-16*cos(x3)*sin(x1)*x2^2 + (-1.1102230246251563^-16*cos(x3)*sin(x1) + (0.0004999999999999999*cos(2.*x1) + 0.701*sin(2.*x1))*sin(x3))*x4^2 + ((cos(2.*x1)*((-0.0004999999999999999 + 5.752078983817783^-17*0) - (0.0004999999999999999 - 5.752078983817783^-17*0)*cos(2.*x3)) - (0.701 - 1.0842021724855044^-19*0)*(1. + 1.*cos(2.*x3))*sin(2.*x1) - 1.110223024625156^-16*sin(x1)*sin(2.*x3))*x2 + (2.220446049250312^-16*cos(x1)*cos(2.*x3) + ((-0.6859999999999999 - 1.0842021724855043^-19*0) - (0.701 - 1.0842021724855044^-19*0)*cos(2.*x1) + (0.0004999999999999999 - 5.752078983817783^-17*0)*sin(2.*x1))*sin(2.*x3))*x4)*x6 + x4*(-0.4858*sin(2.*x1)*sin(x3)*x10 + cos(x3)*(-1.408 - 1.402*cos(2.*x1) + 0.0009999999999999998*sin(2.*x1))*x2 + (-0.12347999999999998*cos(x1)*cos(x3) + (-0.4858 - 0.4858*cos(2.*x1))*cos(2.*x3))*x8) + x2*((0.12347999999999996*cos(x1) + 0.9716*cos(2.*x1)*cos(x3))*x10 + (0.12347999999999996*sin(x1)*sin(x3) + 0.4858*sin(2*x1)*sin(2*x3))*x8)) - 0.4858*(0.12348*cos(x1) - 0.9716*cos(x3))*(0.12347999999999999 + 0.9715999999999999*cos(x1)*cos(x3))*sin(x1)*sin(2.*x1)*sin(x3)*((cos(x3)*(0.942809041582063*cos(x1) - 0.8164965809277258*sin(x1)) + 0.4714045207910315*sin(x3))*u1 + (cos(x3)*(0.9428090415820635*cos(x1) + 0.6123724356957942*sin(x1)) - 2.0034692133618845*sin(x3))*u2 + (cos(x3)*(0.942809041582063*cos(x1) + 2.0412414523193148*sin(x1)) + 0.4714045207910315*sin(x3))*u3 + 1.1102230246251563^-16*cos(x3)*sin(x1)*x2^2 + (-1.1102230246251563^-16*cos(x3)*sin(x1) + (0.0004999999999999999*cos(2.*x1) + 0.701*sin(2.*x1))*sin(x3))*x4^2 + ((cos(2.*x1)*((-0.0004999999999999999 + 5.752078983817783^-17*0) - (0.0004999999999999999 - 5.752078983817783^-17*0)*cos(2.*x3)) - (0.701 - 1.0842021724855044^-19*0)*(1. + 1.*cos(2.*x3))*sin(2.*x1) - 1.110223024625156^-16*sin(x1)*sin(2.*x3))*x2 + (2.220446049250312^-16*cos(x1)*cos(2.*x3) + ((-0.6859999999999999 - 1.0842021724855043^-19*0) - (0.701 - 1.0842021724855044^-19*0)*cos(2.*x1) + (0.0004999999999999999 - 5.752078983817783^-17*0)*sin(2.*x1))*sin(2.*x3))*x4)*x6 + x4*(-0.4858*sin(2.*x1)*sin(x3)*x10 + cos(x3)*(-1.408 - 1.402*cos(2.*x1) + 0.0009999999999999998*sin(2.*x1))*x2 + (-0.12347999999999998*cos(x1)*cos(x3) + (-0.4858 - 0.4858*cos(2.*x1))*cos(2.*x3))*x8) + x2*((0.12347999999999996*cos(x1) + 0.9716*cos(2.*x1)*cos(x3))*x10 + (0.12347999999999996*sin(x1)*sin(x3) + 0.4858*sin(2*x1)*sin(2*x3))*x8)) - 0.165201148*sin(2.*x1)^2*(-1.1102230246251565^-16*cos(x1)*cos(x3) - 1.4080000000000001*sin(x3))*sin(x3)^2*((cos(x3)*(0.942809041582063*cos(x1) - 0.8164965809277258*sin(x1)) + 0.4714045207910315*sin(x3))*u1 + (cos(x3)*(0.9428090415820635*cos(x1) + 0.6123724356957942*sin(x1)) - 2.0034692133618845*sin(x3))*u2 + (cos(x3)*(0.942809041582063*cos(x1) + 2.0412414523193148*sin(x1)) + 0.4714045207910315*sin(x3))*u3 + 1.1102230246251563^-16*cos(x3)*sin(x1)*x2^2 + (-1.1102230246251563^-16*cos(x3)*sin(x1) + (0.0004999999999999999*cos(2.*x1) + 0.701*sin(2.*x1))*sin(x3))*x4^2 + ((cos(2.*x1)*((-0.0004999999999999999 + 5.752078983817783^-17*0) - (0.0004999999999999999 - 5.752078983817783^-17*0)*cos(2.*x3)) - (0.701 - 1.0842021724855044^-19*0)*(1. + 1.*cos(2.*x3))*sin(2.*x1) - 1.110223024625156^-16*sin(x1)*sin(2.*x3))*x2 + (2.220446049250312^-16*cos(x1)*cos(2.*x3) + ((-0.6859999999999999 - 1.0842021724855043^-19*0) - (0.701 - 1.0842021724855044^-19*0)*cos(2.*x1) + (0.0004999999999999999 - 5.752078983817783^-17*0)*sin(2.*x1))*sin(2.*x3))*x4)*x6 + x4*(-0.4858*sin(2.*x1)*sin(x3)*x10 + cos(x3)*(-1.408 - 1.402*cos(2.*x1) + 0.0009999999999999998*sin(2.*x1))*x2 + (-0.12347999999999998*cos(x1)*cos(x3) + (-0.4858 - 0.4858*cos(2.*x1))*cos(2.*x3))*x8) + x2*((0.12347999999999996*cos(x1) + 0.9716*cos(2.*x1)*cos(x3))*x10 + (0.12347999999999996*sin(x1)*sin(x3) + 0.4858*sin(2*x1)*sin(2*x3))*x8)) + (0.12348*cos(x1) - 0.9716*cos(x3))*(-0.9715999999999999*cos(x1)^2 + 0.12347999999999999*cos(x1)*cos(x3) - 1.9431999999999998*sin(x1)^2)*(-0.12347999999999999*cos(x1)*sin(x3) + (-0.24289999999999998 - 0.24289999999999998*cos(2.*x1))*sin(2.*x3))*((cos(x3)*(0.942809041582063*cos(x1) - 0.8164965809277258*sin(x1)) + 0.4714045207910315*sin(x3))*u1 + (cos(x3)*(0.9428090415820635*cos(x1) + 0.6123724356957942*sin(x1)) - 2.0034692133618845*sin(x3))*u2 + (cos(x3)*(0.942809041582063*cos(x1) + 2.0412414523193148*sin(x1)) + 0.4714045207910315*sin(x3))*u3 + 1.1102230246251563^-16*cos(x3)*sin(x1)*x2^2 + (-1.1102230246251563^-16*cos(x3)*sin(x1) + (0.0004999999999999999*cos(2.*x1) + 0.701*sin(2.*x1))*sin(x3))*x4^2 + ((cos(2.*x1)*((-0.0004999999999999999 + 5.752078983817783^-17*0) - (0.0004999999999999999 - 5.752078983817783^-17*0)*cos(2.*x3)) - (0.701 - 1.0842021724855044^-19*0)*(1. + 1.*cos(2.*x3))*sin(2.*x1) - 1.110223024625156^-16*sin(x1)*sin(2.*x3))*x2 + (2.220446049250312^-16*cos(x1)*cos(2.*x3) + ((-0.6859999999999999 - 1.0842021724855043^-19*0) - (0.701 - 1.0842021724855044^-19*0)*cos(2.*x1) + (0.0004999999999999999 - 5.752078983817783^-17*0)*sin(2.*x1))*sin(2.*x3))*x4)*x6 + x4*(-0.4858*sin(2.*x1)*sin(x3)*x10 + cos(x3)*(-1.408 - 1.402*cos(2.*x1) + 0.0009999999999999998*sin(2.*x1))*x2 + (-0.12347999999999998*cos(x1)*cos(x3) + (-0.4858 - 0.4858*cos(2.*x1))*cos(2.*x3))*x8) + x2*((0.12347999999999996*cos(x1) + 0.9716*cos(2.*x1)*cos(x3))*x10 + (0.12347999999999996*sin(x1)*sin(x3) + 0.4858*sin(2*x1)*sin(2*x3))*x8)) - (0.12347999999999999 + 0.9715999999999999*cos(x1)*cos(x3))*(0.8627035999999999 + cos(2.*x1)*(0.17003 - 0.17003*cos(2.*x3)) - 0.17003*cos(2.*x3))*sin(x1)*(cos(x3)*(-0.0005*cos(2.*x1) - 0.701*sin(2.*x1)) - 1.1102230246251564^-16*sin(x1)*sin(x3))*(-17.30484*cos(x3)*sin(x1) - 0.47140452079103157*u1 + 2.003469213361885*u2 - 0.47140452079103157*u3 - 0.34006000000000003*sin(2.*x1)*x10^2 + ((-1.3877787807814455^-17*cos(x3)*sin(x1) + 0.9715999999999999*sin(2.*x1))*x10 - 1.1102230246251564^-16*cos(x1)*x2)*x4 + (-0.0005*cos(2.*x1) - 0.701*sin(2.*x1))*x4^2 + (0.0005*cos(x1)^2*cos(x3)^2 + 1.4019999999999997*cos(x1)*cos(x3)^2*sin(x1) + sin(x1)*(-0.0005*cos(x3)^2*sin(x1) + 5.551115123125783^-17*sin(2.*x3)))*x6^2 + sin(x3)*(cos(2.*x1)*(0.6801200000000001*x10 - 0.9715999999999999*x4) + 0.9715999999999999*x4)*x8 + 0.34006000000000003*sin(2.*x1)*sin(x3)^2*x8^2 + x6*((-0.12347999999999999*cos(x1) - 0.9715999999999999*cos(2.*x1)*cos(x3))*x10 + (cos(x3)*(-1.408 + 1.4019999999999997*cos(2*x1) - 0.001*sin(2*x1)) + 2.220446049250313^-16*cos(x1)*sin(x3))*x4 + (-0.12347999999999999*sin(x1)*sin(x3) - 0.48579999999999995*sin(2.*x1)*sin(2.*x3))*x8)) - 0.34006*sin(2.*x1)*sin(x3)*(cos(x3)*(-0.0005*cos(2.*x1) - 0.701*sin(2.*x1)) - 1.1102230246251564^-16*sin(x1)*sin(x3))*(-0.12347999999999999*cos(x1)*sin(x3) + (-0.24289999999999998 - 0.24289999999999998*cos(2.*x1))*sin(2.*x3))*(-17.30484*cos(x3)*sin(x1) - 0.47140452079103157*u1 + 2.003469213361885*u2 - 0.47140452079103157*u3 - 0.34006000000000003*sin(2.*x1)*x10^2 + ((-1.3877787807814455^-17*cos(x3)*sin(x1) + 0.9715999999999999*sin(2.*x1))*x10 - 1.1102230246251564^-16*cos(x1)*x2)*x4 + (-0.0005*cos(2.*x1) - 0.701*sin(2.*x1))*x4^2 + (0.0005*cos(x1)^2*cos(x3)^2 + 1.4019999999999997*cos(x1)*cos(x3)^2*sin(x1) + sin(x1)*(-0.0005*cos(x3)^2*sin(x1) + 5.551115123125783^-17*sin(2.*x3)))*x6^2 + sin(x3)*(cos(2.*x1)*(0.6801200000000001*x10 - 0.9715999999999999*x4) + 0.9715999999999999*x4)*x8 + 0.34006000000000003*sin(2.*x1)*sin(x3)^2*x8^2 + x6*((-0.12347999999999999*cos(x1) - 0.9715999999999999*cos(2.*x1)*cos(x3))*x10 + (cos(x3)*(-1.408 + 1.4019999999999997*cos(2*x1) - 0.001*sin(2*x1)) + 2.220446049250313^-16*cos(x1)*sin(x3))*x4 + (-0.12347999999999999*sin(x1)*sin(x3) - 0.48579999999999995*sin(2.*x1)*sin(2.*x3))*x8)) + ((1.7510000000000001 + 2.1684043449710084^-19*0) + cos(2.*x1)*((0.3505 - 5.421010862427521^-20*0) + (0.3505 - 5.421010862427521^-20*0)*cos(2.*x3)) + cos(2.*x3)*(0.343 - (0.00025 - 2.8760394919088917^-17*0)*sin(2.*x1)) - (0.00025 - 2.8760394919088917^-17*0)*sin(2.*x1) + 1.1102230246251562^-16*cos(x1)*sin(2.*x3))*(0. + 0.4858*(0.12348*cos(x1) - 0.9716*cos(x3))*sin(2.*x1)*sin(x3)*((1.4288690166235203*cos(x1) + 1.6499158227686102*sin(x1))*u1 + 1.6499158227686104*sin(x1)*u2 + 1.6499158227686102*sin(x1)*u3 + 0.68012*sin(2.*x1)*x10*x2 + cos(x1)*(-1.4288690166235203*u3 - 0.12348*sin(x3)*x2^2) - 0.24696*cos(x3)*sin(x1)*x2*x4 - 0.9716000000000001*sin(2.*x1)*x2*x4 - 0.12348*cos(x1)*sin(x3)*x4^2 + ((0.12347999999999998*cos(x1) + 0.9716*cos(x1)^2*cos(x3) - 0.9716*cos(x3)*sin(x1)^2)*x2 - 0.4858*sin(2*x1)*sin(x3)*x4)*x6 + (-0.68012*cos(2.*x1)*sin(x3)*x2 - 0.34006*cos(x3)*sin(2.*x1)*x4)*x8) - (0.12348*cos(x1) - 0.9716*cos(x3))*(-0.9715999999999999*cos(x1)^2 + 0.12347999999999999*cos(x1)*cos(x3) - 1.9431999999999998*sin(x1)^2)*((0.8249579113843055*cos(x3) + (-1.649915822768611*cos(x1) + 1.4288690166235207*sin(x1))*sin(x3))*u1 + (-1.6499158227686117*cos(x3) - 1.6499158227686117*cos(x1)*sin(x3))*u2 + 0.8249579113843055*cos(x3)*u3 - 1.649915822768611*cos(x1)*sin(x3)*u3 - 1.4288690166235207*sin(x1)*sin(x3)*u3 - 0.68012*cos(2.*x1)*sin(x3)*x10*x2 - 0.12347999999999999*sin(x1)*x2^2 + 0.4858*cos(x3)*sin(2.*x1)*x4^2 + ((0.12347999999999999*sin(x1)*sin(x3) + 0.4858*sin(2.*x1)*sin(2.*x3))*x2 + (5.551115123125783^-17 - 0.12347999999999999*cos(x1)*cos(x3) + (-0.4858 - 0.4858*cos(2.*x1))*cos(2.*x3))*x4)*x6 - 0.68012*sin(2.*x1)*sin(x3)^2*x2*x8 + x4*(-0.34006*cos(x3)*sin(2.*x1)*x10 + (0.9716 + 0.9716*cos(2.*x1))*sin(x3)*x2 + (0.68012*cos(2.*x1)*cos(x3)*sin(x3) + 0.34006*sin(2*x3))*x8)) + (0.8627035999999999 + cos(2.*x1)*(0.17003 - 0.17003*cos(2.*x3)) - 0.17003*cos(2.*x3))*(-0.9715999999999999*cos(x1)^2 + 0.12347999999999999*cos(x1)*cos(x3) - 1.9431999999999998*sin(x1)^2)*(-17.30484*cos(x3)*sin(x1) - 0.47140452079103157*u1 + 2.003469213361885*u2 - 0.47140452079103157*u3 - 0.34006000000000003*sin(2.*x1)*x10^2 + ((-1.3877787807814455^-17*cos(x3)*sin(x1) + 0.9715999999999999*sin(2.*x1))*x10 - 1.1102230246251564^-16*cos(x1)*x2)*x4 + (-0.0005*cos(2.*x1) - 0.701*sin(2.*x1))*x4^2 + (0.0005*cos(x1)^2*cos(x3)^2 + 1.4019999999999997*cos(x1)*cos(x3)^2*sin(x1) + sin(x1)*(-0.0005*cos(x3)^2*sin(x1) + 5.551115123125783^-17*sin(2.*x3)))*x6^2 + sin(x3)*(cos(2.*x1)*(0.6801200000000001*x10 - 0.9715999999999999*x4) + 0.9715999999999999*x4)*x8 + 0.34006000000000003*sin(2.*x1)*sin(x3)^2*x8^2 + x6*((-0.12347999999999999*cos(x1) - 0.9715999999999999*cos(2.*x1)*cos(x3))*x10 + (cos(x3)*(-1.408 + 1.4019999999999997*cos(2*x1) - 0.001*sin(2*x1)) + 2.220446049250313^-16*cos(x1)*sin(x3))*x4 + (-0.12347999999999999*sin(x1)*sin(x3) - 0.48579999999999995*sin(2.*x1)*sin(2.*x3))*x8)) + 0.165201148*sin(2.*x1)^2*sin(x3)^2*(-17.30484*cos(x3)*sin(x1) - 0.47140452079103157*u1 + 2.003469213361885*u2 - 0.47140452079103157*u3 - 0.34006000000000003*sin(2.*x1)*x10^2 + ((-1.3877787807814455^-17*cos(x3)*sin(x1) + 0.9715999999999999*sin(2.*x1))*x10 - 1.1102230246251564^-16*cos(x1)*x2)*x4 + (-0.0005*cos(2.*x1) - 0.701*sin(2.*x1))*x4^2 + (0.0005*cos(x1)^2*cos(x3)^2 + 1.4019999999999997*cos(x1)*cos(x3)^2*sin(x1) + sin(x1)*(-0.0005*cos(x3)^2*sin(x1) + 5.551115123125783^-17*sin(2.*x3)))*x6^2 + sin(x3)*(cos(2.*x1)*(0.6801200000000001*x10 - 0.9715999999999999*x4) + 0.9715999999999999*x4)*x8 + 0.34006000000000003*sin(2.*x1)*sin(x3)^2*x8^2 + x6*((-0.12347999999999999*cos(x1) - 0.9715999999999999*cos(2.*x1)*cos(x3))*x10 + (cos(x3)*(-1.408 + 1.4019999999999997*cos(2*x1) - 0.001*sin(2*x1)) + 2.220446049250313^-16*cos(x1)*sin(x3))*x4 + (-0.12347999999999999*sin(x1)*sin(x3) - 0.48579999999999995*sin(2.*x1)*sin(2.*x3))*x8))) + (-0.12347999999999999*cos(x1)*sin(x3) - (0.2429 + 2.7105054312137602^-20*0)*(1. + 1.*cos(2.*x1))*sin(2.*x3))*(0. - 0.4858*sin(2.*x1)*(-1.1102230246251565^-16*cos(x1)*cos(x3) - 1.4080000000000001*sin(x3))*sin(x3)*((1.4288690166235203*cos(x1) + 1.6499158227686102*sin(x1))*u1 + 1.6499158227686104*sin(x1)*u2 + 1.6499158227686102*sin(x1)*u3 + 0.68012*sin(2.*x1)*x10*x2 + cos(x1)*(-1.4288690166235203*u3 - 0.12348*sin(x3)*x2^2) - 0.24696*cos(x3)*sin(x1)*x2*x4 - 0.9716000000000001*sin(2.*x1)*x2*x4 - 0.12348*cos(x1)*sin(x3)*x4^2 + ((0.12347999999999998*cos(x1) + 0.9716*cos(x1)^2*cos(x3) - 0.9716*cos(x3)*sin(x1)^2)*x2 - 0.4858*sin(2*x1)*sin(x3)*x4)*x6 + (-0.68012*cos(2.*x1)*sin(x3)*x2 - 0.34006*cos(x3)*sin(2.*x1)*x4)*x8) + (-0.9715999999999999*cos(x1)^2 + 0.12347999999999999*cos(x1)*cos(x3) - 1.9431999999999998*sin(x1)^2)*(-1.1102230246251565^-16*cos(x1)*cos(x3) - 1.4080000000000001*sin(x3))*((0.8249579113843055*cos(x3) + (-1.649915822768611*cos(x1) + 1.4288690166235207*sin(x1))*sin(x3))*u1 + (-1.6499158227686117*cos(x3) - 1.6499158227686117*cos(x1)*sin(x3))*u2 + 0.8249579113843055*cos(x3)*u3 - 1.649915822768611*cos(x1)*sin(x3)*u3 - 1.4288690166235207*sin(x1)*sin(x3)*u3 - 0.68012*cos(2.*x1)*sin(x3)*x10*x2 - 0.12347999999999999*sin(x1)*x2^2 + 0.4858*cos(x3)*sin(2.*x1)*x4^2 + ((0.12347999999999999*sin(x1)*sin(x3) + 0.4858*sin(2.*x1)*sin(2.*x3))*x2 + (5.551115123125783^-17 - 0.12347999999999999*cos(x1)*cos(x3) + (-0.4858 - 0.4858*cos(2.*x1))*cos(2.*x3))*x4)*x6 - 0.68012*sin(2.*x1)*sin(x3)^2*x2*x8 + x4*(-0.34006*cos(x3)*sin(2.*x1)*x10 + (0.9716 + 0.9716*cos(2.*x1))*sin(x3)*x2 + (0.68012*cos(2.*x1)*cos(x3)*sin(x3) + 0.34006*sin(2*x3))*x8)) + 0.4858*(0.12347999999999999 + 0.9715999999999999*cos(x1)*cos(x3))*sin(x1)*sin(2.*x1)*sin(x3)*(-17.30484*cos(x3)*sin(x1) - 0.47140452079103157*u1 + 2.003469213361885*u2 - 0.47140452079103157*u3 - 0.34006000000000003*sin(2.*x1)*x10^2 + ((-1.3877787807814455^-17*cos(x3)*sin(x1) + 0.9715999999999999*sin(2.*x1))*x10 - 1.1102230246251564^-16*cos(x1)*x2)*x4 + (-0.0005*cos(2.*x1) - 0.701*sin(2.*x1))*x4^2 + (0.0005*cos(x1)^2*cos(x3)^2 + 1.4019999999999997*cos(x1)*cos(x3)^2*sin(x1) + sin(x1)*(-0.0005*cos(x3)^2*sin(x1) + 5.551115123125783^-17*sin(2.*x3)))*x6^2 + sin(x3)*(cos(2.*x1)*(0.6801200000000001*x10 - 0.9715999999999999*x4) + 0.9715999999999999*x4)*x8 + 0.34006000000000003*sin(2.*x1)*sin(x3)^2*x8^2 + x6*((-0.12347999999999999*cos(x1) - 0.9715999999999999*cos(2.*x1)*cos(x3))*x10 + (cos(x3)*(-1.408 + 1.4019999999999997*cos(2*x1) - 0.001*sin(2*x1)) + 2.220446049250313^-16*cos(x1)*sin(x3))*x4 + (-0.12347999999999999*sin(x1)*sin(x3) - 0.48579999999999995*sin(2.*x1)*sin(2.*x3))*x8)) - (-0.9715999999999999*cos(x1)^2 + 0.12347999999999999*cos(x1)*cos(x3) - 1.9431999999999998*sin(x1)^2)*(-0.12347999999999999*cos(x1)*sin(x3) + (-0.24289999999999998 - 0.24289999999999998*cos(2.*x1))*sin(2.*x3))*(-17.30484*cos(x3)*sin(x1) - 0.47140452079103157*u1 + 2.003469213361885*u2 - 0.47140452079103157*u3 - 0.34006000000000003*sin(2.*x1)*x10^2 + ((-1.3877787807814455^-17*cos(x3)*sin(x1) + 0.9715999999999999*sin(2.*x1))*x10 - 1.1102230246251564^-16*cos(x1)*x2)*x4 + (-0.0005*cos(2.*x1) - 0.701*sin(2.*x1))*x4^2 + (0.0005*cos(x1)^2*cos(x3)^2 + 1.4019999999999997*cos(x1)*cos(x3)^2*sin(x1) + sin(x1)*(-0.0005*cos(x3)^2*sin(x1) + 5.551115123125783^-17*sin(2.*x3)))*x6^2 + sin(x3)*(cos(2.*x1)*(0.6801200000000001*x10 - 0.9715999999999999*x4) + 0.9715999999999999*x4)*x8 + 0.34006000000000003*sin(2.*x1)*sin(x3)^2*x8^2 + x6*((-0.12347999999999999*cos(x1) - 0.9715999999999999*cos(2.*x1)*cos(x3))*x10 + (cos(x3)*(-1.408 + 1.4019999999999997*cos(2*x1) - 0.001*sin(2*x1)) + 2.220446049250313^-16*cos(x1)*sin(x3))*x4 + (-0.12347999999999999*sin(x1)*sin(x3) - 0.48579999999999995*sin(2.*x1)*sin(2.*x3))*x8)))) + 0.4858*sin(2.*x1)*sin(x3)*(0. + 0.34006*sin(2.*x1)*(-1.1102230246251565^-16*cos(x1)*cos(x3) - 1.4080000000000001*sin(x3))*sin(x3)*(cos(x3)*(-0.0005*cos(2.*x1) - 0.701*sin(2.*x1)) - 1.1102230246251564^-16*sin(x1)*sin(x3))*((1.4288690166235203*cos(x1) + 1.6499158227686102*sin(x1))*u1 + 1.6499158227686104*sin(x1)*u2 + 1.6499158227686102*sin(x1)*u3 + 0.68012*sin(2.*x1)*x10*x2 + cos(x1)*(-1.4288690166235203*u3 - 0.12348*sin(x3)*x2^2) - 0.24696*cos(x3)*sin(x1)*x2*x4 - 0.9716000000000001*sin(2.*x1)*x2*x4 - 0.12348*cos(x1)*sin(x3)*x4^2 + ((0.12347999999999998*cos(x1) + 0.9716*cos(x1)^2*cos(x3) - 0.9716*cos(x3)*sin(x1)^2)*x2 - 0.4858*sin(2*x1)*sin(x3)*x4)*x6 + (-0.68012*cos(2.*x1)*sin(x3)*x2 - 0.34006*cos(x3)*sin(2.*x1)*x4)*x8) - 0.12348*sin(x1)*sin(x3)*(cos(x3)*(-0.0005*cos(2.*x1) - 0.701*sin(2.*x1)) - 1.1102230246251564^-16*sin(x1)*sin(x3))*(-0.12347999999999999*cos(x1)*sin(x3) + (-0.24289999999999998 - 0.24289999999999998*cos(2.*x1))*sin(2.*x3))*((1.4288690166235203*cos(x1) + 1.6499158227686102*sin(x1))*u1 + 1.6499158227686104*sin(x1)*u2 + 1.6499158227686102*sin(x1)*u3 + 0.68012*sin(2.*x1)*x10*x2 + cos(x1)*(-1.4288690166235203*u3 - 0.12348*sin(x3)*x2^2) - 0.24696*cos(x3)*sin(x1)*x2*x4 - 0.9716000000000001*sin(2.*x1)*x2*x4 - 0.12348*cos(x1)*sin(x3)*x4^2 + ((0.12347999999999998*cos(x1) + 0.9716*cos(x1)^2*cos(x3) - 0.9716*cos(x3)*sin(x1)^2)*x2 - 0.4858*sin(2*x1)*sin(x3)*x4)*x6 + (-0.68012*cos(2.*x1)*sin(x3)*x2 - 0.34006*cos(x3)*sin(2.*x1)*x4)*x8) + (1.0327336 - 0.34006*cos(2.*x1))*(-1.1102230246251565^-16*cos(x1)*cos(x3) - 1.4080000000000001*sin(x3))*(cos(x3)*(-0.0005*cos(2.*x1) - 0.701*sin(2.*x1)) - 1.1102230246251564^-16*sin(x1)*sin(x3))*((0.8249579113843055*cos(x3) + (-1.649915822768611*cos(x1) + 1.4288690166235207*sin(x1))*sin(x3))*u1 + (-1.6499158227686117*cos(x3) - 1.6499158227686117*cos(x1)*sin(x3))*u2 + 0.8249579113843055*cos(x3)*u3 - 1.649915822768611*cos(x1)*sin(x3)*u3 - 1.4288690166235207*sin(x1)*sin(x3)*u3 - 0.68012*cos(2.*x1)*sin(x3)*x10*x2 - 0.12347999999999999*sin(x1)*x2^2 + 0.4858*cos(x3)*sin(2.*x1)*x4^2 + ((0.12347999999999999*sin(x1)*sin(x3) + 0.4858*sin(2.*x1)*sin(2.*x3))*x2 + (5.551115123125783^-17 - 0.12347999999999999*cos(x1)*cos(x3) + (-0.4858 - 0.4858*cos(2.*x1))*cos(2.*x3))*x4)*x6 - 0.68012*sin(2.*x1)*sin(x3)^2*x2*x8 + x4*(-0.34006*cos(x3)*sin(2.*x1)*x10 + (0.9716 + 0.9716*cos(2.*x1))*sin(x3)*x2 + (0.68012*cos(2.*x1)*cos(x3)*sin(x3) + 0.34006*sin(2*x3))*x8)) + 0.12348*(0.12347999999999999 + 0.9715999999999999*cos(x1)*cos(x3))*sin(x1)^2*sin(x3)*(cos(x3)*(-0.0005*cos(2.*x1) - 0.701*sin(2.*x1)) - 1.1102230246251564^-16*sin(x1)*sin(x3))*((0.8249579113843055*cos(x3) + (-1.649915822768611*cos(x1) + 1.4288690166235207*sin(x1))*sin(x3))*u1 + (-1.6499158227686117*cos(x3) - 1.6499158227686117*cos(x1)*sin(x3))*u2 + 0.8249579113843055*cos(x3)*u3 - 1.649915822768611*cos(x1)*sin(x3)*u3 - 1.4288690166235207*sin(x1)*sin(x3)*u3 - 0.68012*cos(2.*x1)*sin(x3)*x10*x2 - 0.12347999999999999*sin(x1)*x2^2 + 0.4858*cos(x3)*sin(2.*x1)*x4^2 + ((0.12347999999999999*sin(x1)*sin(x3) + 0.4858*sin(2.*x1)*sin(2.*x3))*x2 + (5.551115123125783^-17 - 0.12347999999999999*cos(x1)*cos(x3) + (-0.4858 - 0.4858*cos(2.*x1))*cos(2.*x3))*x4)*x6 - 0.68012*sin(2.*x1)*sin(x3)^2*x2*x8 + x4*(-0.34006*cos(x3)*sin(2.*x1)*x10 + (0.9716 + 0.9716*cos(2.*x1))*sin(x3)*x2 + (0.68012*cos(2.*x1)*cos(x3)*sin(x3) + 0.34006*sin(2*x3))*x8)) - 0.4858*(1.0327336 - 0.34006*cos(2.*x1))*sin(2.*x1)*(-1.1102230246251565^-16*cos(x1)*cos(x3) - 1.4080000000000001*sin(x3))*sin(x3)*((cos(x3)*(0.942809041582063*cos(x1) - 0.8164965809277258*sin(x1)) + 0.4714045207910315*sin(x3))*u1 + (cos(x3)*(0.9428090415820635*cos(x1) + 0.6123724356957942*sin(x1)) - 2.0034692133618845*sin(x3))*u2 + (cos(x3)*(0.942809041582063*cos(x1) + 2.0412414523193148*sin(x1)) + 0.4714045207910315*sin(x3))*u3 + 1.1102230246251563^-16*cos(x3)*sin(x1)*x2^2 + (-1.1102230246251563^-16*cos(x3)*sin(x1) + (0.0004999999999999999*cos(2.*x1) + 0.701*sin(2.*x1))*sin(x3))*x4^2 + ((cos(2.*x1)*((-0.0004999999999999999 + 5.752078983817783^-17*0) - (0.0004999999999999999 - 5.752078983817783^-17*0)*cos(2.*x3)) - (0.701 - 1.0842021724855044^-19*0)*(1. + 1.*cos(2.*x3))*sin(2.*x1) - 1.110223024625156^-16*sin(x1)*sin(2.*x3))*x2 + (2.220446049250312^-16*cos(x1)*cos(2.*x3) + ((-0.6859999999999999 - 1.0842021724855043^-19*0) - (0.701 - 1.0842021724855044^-19*0)*cos(2.*x1) + (0.0004999999999999999 - 5.752078983817783^-17*0)*sin(2.*x1))*sin(2.*x3))*x4)*x6 + x4*(-0.4858*sin(2.*x1)*sin(x3)*x10 + cos(x3)*(-1.408 - 1.402*cos(2.*x1) + 0.0009999999999999998*sin(2.*x1))*x2 + (-0.12347999999999998*cos(x1)*cos(x3) + (-0.4858 - 0.4858*cos(2.*x1))*cos(2.*x3))*x8) + x2*((0.12347999999999996*cos(x1) + 0.9716*cos(2.*x1)*cos(x3))*x10 + (0.12347999999999996*sin(x1)*sin(x3) + 0.4858*sin(2*x1)*sin(2*x3))*x8)) - 0.34006*(-0.9715999999999999*cos(x1)^2 + 0.12347999999999999*cos(x1)*cos(x3) - 1.9431999999999998*sin(x1)^2)*sin(2.*x1)*(-1.1102230246251565^-16*cos(x1)*cos(x3) - 1.4080000000000001*sin(x3))*sin(x3)*((cos(x3)*(0.942809041582063*cos(x1) - 0.8164965809277258*sin(x1)) + 0.4714045207910315*sin(x3))*u1 + (cos(x3)*(0.9428090415820635*cos(x1) + 0.6123724356957942*sin(x1)) - 2.0034692133618845*sin(x3))*u2 + (cos(x3)*(0.942809041582063*cos(x1) + 2.0412414523193148*sin(x1)) + 0.4714045207910315*sin(x3))*u3 + 1.1102230246251563^-16*cos(x3)*sin(x1)*x2^2 + (-1.1102230246251563^-16*cos(x3)*sin(x1) + (0.0004999999999999999*cos(2.*x1) + 0.701*sin(2.*x1))*sin(x3))*x4^2 + ((cos(2.*x1)*((-0.0004999999999999999 + 5.752078983817783^-17*0) - (0.0004999999999999999 - 5.752078983817783^-17*0)*cos(2.*x3)) - (0.701 - 1.0842021724855044^-19*0)*(1. + 1.*cos(2.*x3))*sin(2.*x1) - 1.110223024625156^-16*sin(x1)*sin(2.*x3))*x2 + (2.220446049250312^-16*cos(x1)*cos(2.*x3) + ((-0.6859999999999999 - 1.0842021724855043^-19*0) - (0.701 - 1.0842021724855044^-19*0)*cos(2.*x1) + (0.0004999999999999999 - 5.752078983817783^-17*0)*sin(2.*x1))*sin(2.*x3))*x4)*x6 + x4*(-0.4858*sin(2.*x1)*sin(x3)*x10 + cos(x3)*(-1.408 - 1.402*cos(2.*x1) + 0.0009999999999999998*sin(2.*x1))*x2 + (-0.12347999999999998*cos(x1)*cos(x3) + (-0.4858 - 0.4858*cos(2.*x1))*cos(2.*x3))*x8) + x2*((0.12347999999999996*cos(x1) + 0.9716*cos(2.*x1)*cos(x3))*x10 + (0.12347999999999996*sin(x1)*sin(x3) + 0.4858*sin(2*x1)*sin(2*x3))*x8)) - 0.059986584*(0.12347999999999999 + 0.9715999999999999*cos(x1)*cos(x3))*sin(x1)^2*sin(2.*x1)*sin(x3)^2*((cos(x3)*(0.942809041582063*cos(x1) - 0.8164965809277258*sin(x1)) + 0.4714045207910315*sin(x3))*u1 + (cos(x3)*(0.9428090415820635*cos(x1) + 0.6123724356957942*sin(x1)) - 2.0034692133618845*sin(x3))*u2 + (cos(x3)*(0.942809041582063*cos(x1) + 2.0412414523193148*sin(x1)) + 0.4714045207910315*sin(x3))*u3 + 1.1102230246251563^-16*cos(x3)*sin(x1)*x2^2 + (-1.1102230246251563^-16*cos(x3)*sin(x1) + (0.0004999999999999999*cos(2.*x1) + 0.701*sin(2.*x1))*sin(x3))*x4^2 + ((cos(2.*x1)*((-0.0004999999999999999 + 5.752078983817783^-17*0) - (0.0004999999999999999 - 5.752078983817783^-17*0)*cos(2.*x3)) - (0.701 - 1.0842021724855044^-19*0)*(1. + 1.*cos(2.*x3))*sin(2.*x1) - 1.110223024625156^-16*sin(x1)*sin(2.*x3))*x2 + (2.220446049250312^-16*cos(x1)*cos(2.*x3) + ((-0.6859999999999999 - 1.0842021724855043^-19*0) - (0.701 - 1.0842021724855044^-19*0)*cos(2.*x1) + (0.0004999999999999999 - 5.752078983817783^-17*0)*sin(2.*x1))*sin(2.*x3))*x4)*x6 + x4*(-0.4858*sin(2.*x1)*sin(x3)*x10 + cos(x3)*(-1.408 - 1.402*cos(2.*x1) + 0.0009999999999999998*sin(2.*x1))*x2 + (-0.12347999999999998*cos(x1)*cos(x3) + (-0.4858 - 0.4858*cos(2.*x1))*cos(2.*x3))*x8) + x2*((0.12347999999999996*cos(x1) + 0.9716*cos(2.*x1)*cos(x3))*x10 + (0.12347999999999996*sin(x1)*sin(x3) + 0.4858*sin(2*x1)*sin(2*x3))*x8)) + 0.12348*sin(x1)*(-0.9715999999999999*cos(x1)^2 + 0.12347999999999999*cos(x1)*cos(x3) - 1.9431999999999998*sin(x1)^2)*sin(x3)*(-0.12347999999999999*cos(x1)*sin(x3) + (-0.24289999999999998 - 0.24289999999999998*cos(2.*x1))*sin(2.*x3))*((cos(x3)*(0.942809041582063*cos(x1) - 0.8164965809277258*sin(x1)) + 0.4714045207910315*sin(x3))*u1 + (cos(x3)*(0.9428090415820635*cos(x1) + 0.6123724356957942*sin(x1)) - 2.0034692133618845*sin(x3))*u2 + (cos(x3)*(0.942809041582063*cos(x1) + 2.0412414523193148*sin(x1)) + 0.4714045207910315*sin(x3))*u3 + 1.1102230246251563^-16*cos(x3)*sin(x1)*x2^2 + (-1.1102230246251563^-16*cos(x3)*sin(x1) + (0.0004999999999999999*cos(2.*x1) + 0.701*sin(2.*x1))*sin(x3))*x4^2 + ((cos(2.*x1)*((-0.0004999999999999999 + 5.752078983817783^-17*0) - (0.0004999999999999999 - 5.752078983817783^-17*0)*cos(2.*x3)) - (0.701 - 1.0842021724855044^-19*0)*(1. + 1.*cos(2.*x3))*sin(2.*x1) - 1.110223024625156^-16*sin(x1)*sin(2.*x3))*x2 + (2.220446049250312^-16*cos(x1)*cos(2.*x3) + ((-0.6859999999999999 - 1.0842021724855043^-19*0) - (0.701 - 1.0842021724855044^-19*0)*cos(2.*x1) + (0.0004999999999999999 - 5.752078983817783^-17*0)*sin(2.*x1))*sin(2.*x3))*x4)*x6 + x4*(-0.4858*sin(2.*x1)*sin(x3)*x10 + cos(x3)*(-1.408 - 1.402*cos(2.*x1) + 0.0009999999999999998*sin(2.*x1))*x2 + (-0.12347999999999998*cos(x1)*cos(x3) + (-0.4858 - 0.4858*cos(2.*x1))*cos(2.*x3))*x8) + x2*((0.12347999999999996*cos(x1) + 0.9716*cos(2.*x1)*cos(x3))*x10 + (0.12347999999999996*sin(x1)*sin(x3) + 0.4858*sin(2*x1)*sin(2*x3))*x8)) - 0.34006*(0.12347999999999999 + 0.9715999999999999*cos(x1)*cos(x3))*sin(x1)*sin(2.*x1)*sin(x3)*(cos(x3)*(-0.0005*cos(2.*x1) - 0.701*sin(2.*x1)) - 1.1102230246251564^-16*sin(x1)*sin(x3))*(-17.30484*cos(x3)*sin(x1) - 0.47140452079103157*u1 + 2.003469213361885*u2 - 0.47140452079103157*u3 - 0.34006000000000003*sin(2.*x1)*x10^2 + ((-1.3877787807814455^-17*cos(x3)*sin(x1) + 0.9715999999999999*sin(2.*x1))*x10 - 1.1102230246251564^-16*cos(x1)*x2)*x4 + (-0.0005*cos(2.*x1) - 0.701*sin(2.*x1))*x4^2 + (0.0005*cos(x1)^2*cos(x3)^2 + 1.4019999999999997*cos(x1)*cos(x3)^2*sin(x1) + sin(x1)*(-0.0005*cos(x3)^2*sin(x1) + 5.551115123125783^-17*sin(2.*x3)))*x6^2 + sin(x3)*(cos(2.*x1)*(0.6801200000000001*x10 - 0.9715999999999999*x4) + 0.9715999999999999*x4)*x8 + 0.34006000000000003*sin(2.*x1)*sin(x3)^2*x8^2 + x6*((-0.12347999999999999*cos(x1) - 0.9715999999999999*cos(2.*x1)*cos(x3))*x10 + (cos(x3)*(-1.408 + 1.4019999999999997*cos(2*x1) - 0.001*sin(2*x1)) + 2.220446049250313^-16*cos(x1)*sin(x3))*x4 + (-0.12347999999999999*sin(x1)*sin(x3) - 0.48579999999999995*sin(2.*x1)*sin(2.*x3))*x8)) - (1.0327336 - 0.34006*cos(2.*x1))*(cos(x3)*(-0.0005*cos(2.*x1) - 0.701*sin(2.*x1)) - 1.1102230246251564^-16*sin(x1)*sin(x3))*(-0.12347999999999999*cos(x1)*sin(x3) + (-0.24289999999999998 - 0.24289999999999998*cos(2.*x1))*sin(2.*x3))*(-17.30484*cos(x3)*sin(x1) - 0.47140452079103157*u1 + 2.003469213361885*u2 - 0.47140452079103157*u3 - 0.34006000000000003*sin(2.*x1)*x10^2 + ((-1.3877787807814455^-17*cos(x3)*sin(x1) + 0.9715999999999999*sin(2.*x1))*x10 - 1.1102230246251564^-16*cos(x1)*x2)*x4 + (-0.0005*cos(2.*x1) - 0.701*sin(2.*x1))*x4^2 + (0.0005*cos(x1)^2*cos(x3)^2 + 1.4019999999999997*cos(x1)*cos(x3)^2*sin(x1) + sin(x1)*(-0.0005*cos(x3)^2*sin(x1) + 5.551115123125783^-17*sin(2.*x3)))*x6^2 + sin(x3)*(cos(2.*x1)*(0.6801200000000001*x10 - 0.9715999999999999*x4) + 0.9715999999999999*x4)*x8 + 0.34006000000000003*sin(2.*x1)*sin(x3)^2*x8^2 + x6*((-0.12347999999999999*cos(x1) - 0.9715999999999999*cos(2.*x1)*cos(x3))*x10 + (cos(x3)*(-1.408 + 1.4019999999999997*cos(2*x1) - 0.001*sin(2*x1)) + 2.220446049250313^-16*cos(x1)*sin(x3))*x4 + (-0.12347999999999999*sin(x1)*sin(x3) - 0.48579999999999995*sin(2.*x1)*sin(2.*x3))*x8)) + ((1.7510000000000001 + 2.1684043449710084^-19*0) + cos(2.*x1)*((0.3505 - 5.421010862427521^-20*0) + (0.3505 - 5.421010862427521^-20*0)*cos(2.*x3)) + cos(2.*x3)*(0.343 - (0.00025 - 2.8760394919088917^-17*0)*sin(2.*x1)) - (0.00025 - 2.8760394919088917^-17*0)*sin(2.*x1) + 1.1102230246251562^-16*cos(x1)*sin(2.*x3))*(0. + 0.059986584*sin(x1)*sin(2.*x1)*sin(x3)^2*((1.4288690166235203*cos(x1) + 1.6499158227686102*sin(x1))*u1 + 1.6499158227686104*sin(x1)*u2 + 1.6499158227686102*sin(x1)*u3 + 0.68012*sin(2.*x1)*x10*x2 + cos(x1)*(-1.4288690166235203*u3 - 0.12348*sin(x3)*x2^2) - 0.24696*cos(x3)*sin(x1)*x2*x4 - 0.9716000000000001*sin(2.*x1)*x2*x4 - 0.12348*cos(x1)*sin(x3)*x4^2 + ((0.12347999999999998*cos(x1) + 0.9716*cos(x1)^2*cos(x3) - 0.9716*cos(x3)*sin(x1)^2)*x2 - 0.4858*sin(2*x1)*sin(x3)*x4)*x6 + (-0.68012*cos(2.*x1)*sin(x3)*x2 - 0.34006*cos(x3)*sin(2.*x1)*x4)*x8) - 0.12348*sin(x1)*(-0.9715999999999999*cos(x1)^2 + 0.12347999999999999*cos(x1)*cos(x3) - 1.9431999999999998*sin(x1)^2)*sin(x3)*((0.8249579113843055*cos(x3) + (-1.649915822768611*cos(x1) + 1.4288690166235207*sin(x1))*sin(x3))*u1 + (-1.6499158227686117*cos(x3) - 1.6499158227686117*cos(x1)*sin(x3))*u2 + 0.8249579113843055*cos(x3)*u3 - 1.649915822768611*cos(x1)*sin(x3)*u3 - 1.4288690166235207*sin(x1)*sin(x3)*u3 - 0.68012*cos(2.*x1)*sin(x3)*x10*x2 - 0.12347999999999999*sin(x1)*x2^2 + 0.4858*cos(x3)*sin(2.*x1)*x4^2 + ((0.12347999999999999*sin(x1)*sin(x3) + 0.4858*sin(2.*x1)*sin(2.*x3))*x2 + (5.551115123125783^-17 - 0.12347999999999999*cos(x1)*cos(x3) + (-0.4858 - 0.4858*cos(2.*x1))*cos(2.*x3))*x4)*x6 - 0.68012*sin(2.*x1)*sin(x3)^2*x2*x8 + x4*(-0.34006*cos(x3)*sin(2.*x1)*x10 + (0.9716 + 0.9716*cos(2.*x1))*sin(x3)*x2 + (0.68012*cos(2.*x1)*cos(x3)*sin(x3) + 0.34006*sin(2*x3))*x8)) + 0.4858*(1.0327336 - 0.34006*cos(2.*x1))*sin(2.*x1)*sin(x3)*(-17.30484*cos(x3)*sin(x1) - 0.47140452079103157*u1 + 2.003469213361885*u2 - 0.47140452079103157*u3 - 0.34006000000000003*sin(2.*x1)*x10^2 + ((-1.3877787807814455^-17*cos(x3)*sin(x1) + 0.9715999999999999*sin(2.*x1))*x10 - 1.1102230246251564^-16*cos(x1)*x2)*x4 + (-0.0005*cos(2.*x1) - 0.701*sin(2.*x1))*x4^2 + (0.0005*cos(x1)^2*cos(x3)^2 + 1.4019999999999997*cos(x1)*cos(x3)^2*sin(x1) + sin(x1)*(-0.0005*cos(x3)^2*sin(x1) + 5.551115123125783^-17*sin(2.*x3)))*x6^2 + sin(x3)*(cos(2.*x1)*(0.6801200000000001*x10 - 0.9715999999999999*x4) + 0.9715999999999999*x4)*x8 + 0.34006000000000003*sin(2.*x1)*sin(x3)^2*x8^2 + x6*((-0.12347999999999999*cos(x1) - 0.9715999999999999*cos(2.*x1)*cos(x3))*x10 + (cos(x3)*(-1.408 + 1.4019999999999997*cos(2*x1) - 0.001*sin(2*x1)) + 2.220446049250313^-16*cos(x1)*sin(x3))*x4 + (-0.12347999999999999*sin(x1)*sin(x3) - 0.48579999999999995*sin(2.*x1)*sin(2.*x3))*x8)) + 0.34006*(-0.9715999999999999*cos(x1)^2 + 0.12347999999999999*cos(x1)*cos(x3) - 1.9431999999999998*sin(x1)^2)*sin(2.*x1)*sin(x3)*(-17.30484*cos(x3)*sin(x1) - 0.47140452079103157*u1 + 2.003469213361885*u2 - 0.47140452079103157*u3 - 0.34006000000000003*sin(2.*x1)*x10^2 + ((-1.3877787807814455^-17*cos(x3)*sin(x1) + 0.9715999999999999*sin(2.*x1))*x10 - 1.1102230246251564^-16*cos(x1)*x2)*x4 + (-0.0005*cos(2.*x1) - 0.701*sin(2.*x1))*x4^2 + (0.0005*cos(x1)^2*cos(x3)^2 + 1.4019999999999997*cos(x1)*cos(x3)^2*sin(x1) + sin(x1)*(-0.0005*cos(x3)^2*sin(x1) + 5.551115123125783^-17*sin(2.*x3)))*x6^2 + sin(x3)*(cos(2.*x1)*(0.6801200000000001*x10 - 0.9715999999999999*x4) + 0.9715999999999999*x4)*x8 + 0.34006000000000003*sin(2.*x1)*sin(x3)^2*x8^2 + x6*((-0.12347999999999999*cos(x1) - 0.9715999999999999*cos(2.*x1)*cos(x3))*x10 + (cos(x3)*(-1.408 + 1.4019999999999997*cos(2*x1) - 0.001*sin(2*x1)) + 2.220446049250313^-16*cos(x1)*sin(x3))*x4 + (-0.12347999999999999*sin(x1)*sin(x3) - 0.48579999999999995*sin(2.*x1)*sin(2.*x3))*x8))) + (0.12347999999999999*sin(x1) + 0.4858*cos(x3)*sin(2.*x1))*(0. + 0.4858*sin(2.*x1)*(-1.1102230246251565^-16*cos(x1)*cos(x3) - 1.4080000000000001*sin(x3))*sin(x3)*((1.4288690166235203*cos(x1) + 1.6499158227686102*sin(x1))*u1 + 1.6499158227686104*sin(x1)*u2 + 1.6499158227686102*sin(x1)*u3 + 0.68012*sin(2.*x1)*x10*x2 + cos(x1)*(-1.4288690166235203*u3 - 0.12348*sin(x3)*x2^2) - 0.24696*cos(x3)*sin(x1)*x2*x4 - 0.9716000000000001*sin(2.*x1)*x2*x4 - 0.12348*cos(x1)*sin(x3)*x4^2 + ((0.12347999999999998*cos(x1) + 0.9716*cos(x1)^2*cos(x3) - 0.9716*cos(x3)*sin(x1)^2)*x2 - 0.4858*sin(2*x1)*sin(x3)*x4)*x6 + (-0.68012*cos(2.*x1)*sin(x3)*x2 - 0.34006*cos(x3)*sin(2.*x1)*x4)*x8) - (-0.9715999999999999*cos(x1)^2 + 0.12347999999999999*cos(x1)*cos(x3) - 1.9431999999999998*sin(x1)^2)*(-1.1102230246251565^-16*cos(x1)*cos(x3) - 1.4080000000000001*sin(x3))*((0.8249579113843055*cos(x3) + (-1.649915822768611*cos(x1) + 1.4288690166235207*sin(x1))*sin(x3))*u1 + (-1.6499158227686117*cos(x3) - 1.6499158227686117*cos(x1)*sin(x3))*u2 + 0.8249579113843055*cos(x3)*u3 - 1.649915822768611*cos(x1)*sin(x3)*u3 - 1.4288690166235207*sin(x1)*sin(x3)*u3 - 0.68012*cos(2.*x1)*sin(x3)*x10*x2 - 0.12347999999999999*sin(x1)*x2^2 + 0.4858*cos(x3)*sin(2.*x1)*x4^2 + ((0.12347999999999999*sin(x1)*sin(x3) + 0.4858*sin(2.*x1)*sin(2.*x3))*x2 + (5.551115123125783^-17 - 0.12347999999999999*cos(x1)*cos(x3) + (-0.4858 - 0.4858*cos(2.*x1))*cos(2.*x3))*x4)*x6 - 0.68012*sin(2.*x1)*sin(x3)^2*x2*x8 + x4*(-0.34006*cos(x3)*sin(2.*x1)*x10 + (0.9716 + 0.9716*cos(2.*x1))*sin(x3)*x2 + (0.68012*cos(2.*x1)*cos(x3)*sin(x3) + 0.34006*sin(2*x3))*x8)) - 0.4858*(0.12347999999999999 + 0.9715999999999999*cos(x1)*cos(x3))*sin(x1)*sin(2.*x1)*sin(x3)*(-17.30484*cos(x3)*sin(x1) - 0.47140452079103157*u1 + 2.003469213361885*u2 - 0.47140452079103157*u3 - 0.34006000000000003*sin(2.*x1)*x10^2 + ((-1.3877787807814455^-17*cos(x3)*sin(x1) + 0.9715999999999999*sin(2.*x1))*x10 - 1.1102230246251564^-16*cos(x1)*x2)*x4 + (-0.0005*cos(2.*x1) - 0.701*sin(2.*x1))*x4^2 + (0.0005*cos(x1)^2*cos(x3)^2 + 1.4019999999999997*cos(x1)*cos(x3)^2*sin(x1) + sin(x1)*(-0.0005*cos(x3)^2*sin(x1) + 5.551115123125783^-17*sin(2.*x3)))*x6^2 + sin(x3)*(cos(2.*x1)*(0.6801200000000001*x10 - 0.9715999999999999*x4) + 0.9715999999999999*x4)*x8 + 0.34006000000000003*sin(2.*x1)*sin(x3)^2*x8^2 + x6*((-0.12347999999999999*cos(x1) - 0.9715999999999999*cos(2.*x1)*cos(x3))*x10 + (cos(x3)*(-1.408 + 1.4019999999999997*cos(2*x1) - 0.001*sin(2*x1)) + 2.220446049250313^-16*cos(x1)*sin(x3))*x4 + (-0.12347999999999999*sin(x1)*sin(x3) - 0.48579999999999995*sin(2.*x1)*sin(2.*x3))*x8)) + (-0.9715999999999999*cos(x1)^2 + 0.12347999999999999*cos(x1)*cos(x3) - 1.9431999999999998*sin(x1)^2)*(-0.12347999999999999*cos(x1)*sin(x3) + (-0.24289999999999998 - 0.24289999999999998*cos(2.*x1))*sin(2.*x3))*(-17.30484*cos(x3)*sin(x1) - 0.47140452079103157*u1 + 2.003469213361885*u2 - 0.47140452079103157*u3 - 0.34006000000000003*sin(2.*x1)*x10^2 + ((-1.3877787807814455^-17*cos(x3)*sin(x1) + 0.9715999999999999*sin(2.*x1))*x10 - 1.1102230246251564^-16*cos(x1)*x2)*x4 + (-0.0005*cos(2.*x1) - 0.701*sin(2.*x1))*x4^2 + (0.0005*cos(x1)^2*cos(x3)^2 + 1.4019999999999997*cos(x1)*cos(x3)^2*sin(x1) + sin(x1)*(-0.0005*cos(x3)^2*sin(x1) + 5.551115123125783^-17*sin(2.*x3)))*x6^2 + sin(x3)*(cos(2.*x1)*(0.6801200000000001*x10 - 0.9715999999999999*x4) + 0.9715999999999999*x4)*x8 + 0.34006000000000003*sin(2.*x1)*sin(x3)^2*x8^2 + x6*((-0.12347999999999999*cos(x1) - 0.9715999999999999*cos(2.*x1)*cos(x3))*x10 + (cos(x3)*(-1.408 + 1.4019999999999997*cos(2*x1) - 0.001*sin(2*x1)) + 2.220446049250313^-16*cos(x1)*sin(x3))*x4 + (-0.12347999999999999*sin(x1)*sin(x3) - 0.48579999999999995*sin(2.*x1)*sin(2.*x3))*x8)))))/(0. - 1.408*(0.12347999999999999 + 0.9715999999999999*cos(x1)*cos(x3))*(0.8627035999999999 + cos(2.*x1)*(0.17003 - 0.17003*cos(2.*x3)) - 0.17003*cos(2.*x3))*sin(x1)*(2.0940000000000003 - 0.7010000000000001*cos(2.*x1) + 0.0005*sin(2.*x1))*(0.12347999999999999*sin(x1) + 0.4858*cos(x3)*sin(2.*x1)) - 1.1102230246251565^-16*(0.8627035999999999 + cos(2.*x1)*(0.17003 - 0.17003*cos(2.*x3)) - 0.17003*cos(2.*x3))*sin(x1)*(-0.9715999999999999*cos(x1)^2 + 0.12347999999999999*cos(x1)*cos(x3) - 1.9431999999999998*sin(x1)^2)*(0.12347999999999999*sin(x1) + 0.4858*cos(x3)*sin(2.*x1))*(-1.1102230246251565^-16*cos(x1)*cos(x3) - 1.4080000000000001*sin(x3)) + (-1.4574 + 0.4858*cos(2.*x1) + 0.12348*cos(x1)*cos(x3))*(0.8627035999999999 + cos(2.*x1)*(0.17003 - 0.17003*cos(2.*x3)) - 0.17003*cos(2.*x3))*(-0.9715999999999999*cos(x1)^2 + 0.12347999999999999*cos(x1)*cos(x3) - 1.9431999999999998*sin(x1)^2)*(-1.1102230246251565^-16*cos(x1)*cos(x3) - 1.4080000000000001*sin(x3))^2 - 0.12348*(0.8627035999999999 + cos(2.*x1)*(0.17003 - 0.17003*cos(2.*x3)) - 0.17003*cos(2.*x3))*sin(x1)*(2.0940000000000003 - 0.7010000000000001*cos(2.*x1) + 0.0005*sin(2.*x1))*(0.12347999999999999*sin(x1) + 0.4858*cos(x3)*sin(2.*x1))*(-1.1102230246251565^-16*cos(x1)*cos(x3) - 1.4080000000000001*sin(x3))*sin(x3) + 0.4858*(0.12347999999999999*cos(x1) - 0.9715999999999999*cos(x3))*(-0.9715999999999999*cos(x1)^2 + 0.12347999999999999*cos(x1)*cos(x3) - 1.9431999999999998*sin(x1)^2)*sin(2.*x1)*(0.12347999999999999*sin(x1) + 0.4858*cos(x3)*sin(2.*x1))*(-1.1102230246251565^-16*cos(x1)*cos(x3) - 1.4080000000000001*sin(x3))*sin(x3) + 0.34006*(0.12347999999999999*cos(x1) - 0.9715999999999999*cos(x3))*(2.0940000000000003 - 0.7010000000000001*cos(2.*x1) + 0.0005*sin(2.*x1))*sin(2.*x1)*(0.12347999999999999*sin(x1) + 0.4858*cos(x3)*sin(2.*x1))*(-1.1102230246251565^-16*cos(x1)*cos(x3) - 1.4080000000000001*sin(x3))*sin(x3) + 0.33229030912*(0.12347999999999999 + 0.9715999999999999*cos(x1)*cos(x3))*sin(x1)*sin(2.*x1)^2*(0.12347999999999999*sin(x1) + 0.4858*cos(x3)*sin(2.*x1))*sin(x3)^2 - 1.8341011820410812^-17*sin(x1)*sin(2.*x1)^2*(0.12347999999999999*sin(x1) + 0.4858*cos(x3)*sin(2.*x1))*(-1.1102230246251565^-16*cos(x1)*cos(x3) - 1.4080000000000001*sin(x3))*sin(x3)^2 + 0.165201148*(-1.4574 + 0.4858*cos(2.*x1) + 0.12348*cos(x1)*cos(x3))*sin(2.*x1)^2*(-1.1102230246251565^-16*cos(x1)*cos(x3) - 1.4080000000000001*sin(x3))^2*sin(x3)^2 + 0.165201148*(-0.9715999999999999*cos(x1)^2 + 0.12347999999999999*cos(x1)*cos(x3) - 1.9431999999999998*sin(x1)^2)*sin(2.*x1)^2*(-1.1102230246251565^-16*cos(x1)*cos(x3) - 1.4080000000000001*sin(x3))^2*sin(x3)^2 + 0.11564080359999998*(2.0940000000000003 - 0.7010000000000001*cos(2.*x1) + 0.0005*sin(2.*x1))*sin(2.*x1)^2*(-1.1102230246251565^-16*cos(x1)*cos(x3) - 1.4080000000000001*sin(x3))^2*sin(x3)^2 + 0.029141482507200004*sin(x1)*sin(2.*x1)^2*(0.12347999999999999*sin(x1) + 0.4858*cos(x3)*sin(2.*x1))*(-1.1102230246251565^-16*cos(x1)*cos(x3) - 1.4080000000000001*sin(x3))*sin(x3)^3 + 1.408*(0.8627035999999999 + cos(2.*x1)*(0.17003 - 0.17003*cos(2.*x3)) - 0.17003*cos(2.*x3))*(-0.9715999999999999*cos(x1)^2 + 0.12347999999999999*cos(x1)*cos(x3) - 1.9431999999999998*sin(x1)^2)*(0.12347999999999999*sin(x1) + 0.4858*cos(x3)*sin(2.*x1))*(cos(x3)*(-0.0005*cos(2.*x1) - 0.7010000000000001*sin(2.*x1)) - 1.1102230246251565^-16*sin(x1)*sin(x3)) + 0.23260321638399997*sin(2.*x1)^2*(0.12347999999999999*sin(x1) + 0.4858*cos(x3)*sin(2.*x1))*sin(x3)^2*(cos(x3)*(-0.0005*cos(2.*x1) - 0.7010000000000001*sin(2.*x1)) - 1.1102230246251565^-16*sin(x1)*sin(x3)) + 0.16282225146879997*sin(2.*x1)^2*sin(x3)^2*(cos(x3)*(-0.0005*cos(2.*x1) - 0.7010000000000001*sin(2.*x1)) - 1.1102230246251565^-16*sin(x1)*sin(x3))^2 + 1.408*(-1.4574 + 0.4858*cos(2.*x1) + 0.12348*cos(x1)*cos(x3))*(0.12347999999999999 + 0.9715999999999999*cos(x1)*cos(x3))*(0.8627035999999999 + cos(2.*x1)*(0.17003 - 0.17003*cos(2.*x3)) - 0.17003*cos(2.*x3))*sin(x1)*(cos(x3)*(-0.0005*cos(2.*x1) - 0.701*sin(2.*x1)) - 1.1102230246251564^-16*sin(x1)*sin(x3)) + 0.12348*(-1.4574 + 0.4858*cos(2.*x1) + 0.12348*cos(x1)*cos(x3))*(0.8627035999999999 + cos(2.*x1)*(0.17003 - 0.17003*cos(2.*x3)) - 0.17003*cos(2.*x3))*sin(x1)*(-1.1102230246251565^-16*cos(x1)*cos(x3) - 1.4080000000000001*sin(x3))*sin(x3)*(cos(x3)*(-0.0005*cos(2.*x1) - 0.701*sin(2.*x1)) - 1.1102230246251564^-16*sin(x1)*sin(x3)) - 0.34006*(0.12347999999999999*cos(x1) - 0.9715999999999999*cos(x3))*(-1.4574 + 0.4858*cos(2.*x1) + 0.12348*cos(x1)*cos(x3))*sin(2.*x1)*(-1.1102230246251565^-16*cos(x1)*cos(x3) - 1.4080000000000001*sin(x3))*sin(x3)*(cos(x3)*(-0.0005*cos(2.*x1) - 0.701*sin(2.*x1)) - 1.1102230246251564^-16*sin(x1)*sin(x3)) + 0.23260321638399997*(0.12347999999999999 + 0.9715999999999999*cos(x1)*cos(x3))*sin(x1)*sin(2.*x1)^2*sin(x3)^2*(cos(x3)*(-0.0005*cos(2.*x1) - 0.701*sin(2.*x1)) - 1.1102230246251564^-16*sin(x1)*sin(x3)) - 1.2838708274287567^-17*sin(x1)*sin(2.*x1)^2*(-1.1102230246251565^-16*cos(x1)*cos(x3) - 1.4080000000000001*sin(x3))*sin(x3)^2*(cos(x3)*(-0.0005*cos(2.*x1) - 0.701*sin(2.*x1)) - 1.1102230246251564^-16*sin(x1)*sin(x3)) + 0.020399037755039998*sin(x1)*sin(2.*x1)^2*(-1.1102230246251565^-16*cos(x1)*cos(x3) - 1.4080000000000001*sin(x3))*sin(x3)^3*(cos(x3)*(-0.0005*cos(2.*x1) - 0.701*sin(2.*x1)) - 1.1102230246251564^-16*sin(x1)*sin(x3)) - 1.408*(-1.4574 + 0.4858*cos(2.*x1) + 0.12348*cos(x1)*cos(x3))*(0.8627035999999999 + cos(2.*x1)*(0.17003 - 0.17003*cos(2.*x3)) - 0.17003*cos(2.*x3))*(-0.9715999999999999*cos(x1)^2 + 0.12347999999999999*cos(x1)*cos(x3) - 1.9431999999999998*sin(x1)^2)*((1.7510000000000001 + 2.1684043449710084^-19*0) + cos(2.*x1)*((0.3505 - 5.421010862427521^-20*0) + (0.3505 - 5.421010862427521^-20*0)*cos(2.*x3)) + cos(2.*x3)*(0.343 - (0.00025 - 2.8760394919088917^-17*0)*sin(2.*x1)) - (0.00025 - 2.8760394919088917^-17*0)*sin(2.*x1) + 1.1102230246251562^-16*cos(x1)*sin(2.*x3)) - 0.23260321638399997*(-1.4574 + 0.4858*cos(2.*x1) + 0.12348*cos(x1)*cos(x3))*sin(2.*x1)^2*sin(x3)^2*((1.7510000000000001 + 2.1684043449710084^-19*0) + cos(2.*x1)*((0.3505 - 5.421010862427521^-20*0) + (0.3505 - 5.421010862427521^-20*0)*cos(2.*x3)) + cos(2.*x3)*(0.343 - (0.00025 - 2.8760394919088917^-17*0)*sin(2.*x1)) - (0.00025 - 2.8760394919088917^-17*0)*sin(2.*x1) + 1.1102230246251562^-16*cos(x1)*sin(2.*x3)) - 0.23260321638399997*(-0.9715999999999999*cos(x1)^2 + 0.12347999999999999*cos(x1)*cos(x3) - 1.9431999999999998*sin(x1)^2)*sin(2.*x1)^2*sin(x3)^2*((1.7510000000000001 + 2.1684043449710084^-19*0) + cos(2.*x1)*((0.3505 - 5.421010862427521^-20*0) + (0.3505 - 5.421010862427521^-20*0)*cos(2.*x3)) + cos(2.*x3)*(0.343 - (0.00025 - 2.8760394919088917^-17*0)*sin(2.*x1)) - (0.00025 - 2.8760394919088917^-17*0)*sin(2.*x1) + 1.1102230246251562^-16*cos(x1)*sin(2.*x3)) - 0.16282225146879997*(2.0940000000000003 - 0.7010000000000001*cos(2.*x1) + 0.0005*sin(2.*x1))*sin(2.*x1)^2*sin(x3)^2*((1.7510000000000001 + 2.1684043449710084^-19*0) + cos(2.*x1)*((0.3505 - 5.421010862427521^-20*0) + (0.3505 - 5.421010862427521^-20*0)*cos(2.*x3)) + cos(2.*x3)*(0.343 - (0.00025 - 2.8760394919088917^-17*0)*sin(2.*x1)) - (0.00025 - 2.8760394919088917^-17*0)*sin(2.*x1) + 1.1102230246251562^-16*cos(x1)*sin(2.*x3)) - 0.6840064*(-0.9715999999999999*cos(x1)^2 + 0.12347999999999999*cos(x1)*cos(x3) - 1.9431999999999998*sin(x1)^2)*sin(2.*x1)*(0.12347999999999999*sin(x1) + 0.4858*cos(x3)*sin(2.*x1))*sin(x3)*(-0.12347999999999999*cos(x1)*sin(x3) + (-0.24289999999999998 - 0.24289999999999998*cos(2.*x1))*sin(2.*x3)) - 0.4788044799999999*(2.0940000000000003 - 0.7010000000000001*cos(2.*x1) + 0.0005*sin(2.*x1))*sin(2.*x1)*(0.12347999999999999*sin(x1) + 0.4858*cos(x3)*sin(2.*x1))*sin(x3)*(-0.12347999999999999*cos(x1)*sin(x3) + (-0.24289999999999998 - 0.24289999999999998*cos(2.*x1))*sin(2.*x3)) + 0.4788044799999999*(-1.4574 + 0.4858*cos(2.*x1) + 0.12348*cos(x1)*cos(x3))*sin(2.*x1)*sin(x3)*(cos(x3)*(-0.0005*cos(2.*x1) - 0.701*sin(2.*x1)) - 1.1102230246251564^-16*sin(x1)*sin(x3))*(-0.12347999999999999*cos(x1)*sin(x3) + (-0.24289999999999998 - 0.24289999999999998*cos(2.*x1))*sin(2.*x3)) - (0.12347999999999999*cos(x1) - 0.9715999999999999*cos(x3))*(-1.4574 + 0.4858*cos(2.*x1) + 0.12348*cos(x1)*cos(x3))*(-0.9715999999999999*cos(x1)^2 + 0.12347999999999999*cos(x1)*cos(x3) - 1.9431999999999998*sin(x1)^2)*(-1.1102230246251565^-16*cos(x1)*cos(x3) - 1.4080000000000001*sin(x3))*(-0.12347999999999999*cos(x1)*sin(x3) - (0.2429 + 2.7105054312137602^-20*0)*(1. + 1.*cos(2.*x1))*sin(2.*x3)) - 0.6840064*(-1.4574 + 0.4858*cos(2.*x1) + 0.12348*cos(x1)*cos(x3))*(0.12347999999999999 + 0.9715999999999999*cos(x1)*cos(x3))*sin(x1)*sin(2.*x1)*sin(x3)*(-0.12347999999999999*cos(x1)*sin(x3) - (0.2429 + 2.7105054312137602^-20*0)*(1. + 1.*cos(2.*x1))*sin(2.*x3)) - 0.4788044799999999*(0.12347999999999999 + 0.9715999999999999*cos(x1)*cos(x3))*sin(x1)*(2.0940000000000003 - 0.7010000000000001*cos(2.*x1) + 0.0005*sin(2.*x1))*sin(2.*x1)*sin(x3)*(-0.12347999999999999*cos(x1)*sin(x3) - (0.2429 + 2.7105054312137602^-20*0)*(1. + 1.*cos(2.*x1))*sin(2.*x3)) - 3.775424417540307^-17*sin(x1)*(-0.9715999999999999*cos(x1)^2 + 0.12347999999999999*cos(x1)*cos(x3) - 1.9431999999999998*sin(x1)^2)*sin(2.*x1)*(-1.1102230246251565^-16*cos(x1)*cos(x3) - 1.4080000000000001*sin(x3))*sin(x3)*(-0.12347999999999999*cos(x1)*sin(x3) - (0.2429 + 2.7105054312137602^-20*0)*(1. + 1.*cos(2.*x1))*sin(2.*x3)) - 0.059986584*(-1.4574 + 0.4858*cos(2.*x1) + 0.12348*cos(x1)*cos(x3))*sin(x1)*sin(2.*x1)*(-1.1102230246251565^-16*cos(x1)*cos(x3) - 1.4080000000000001*sin(x3))*sin(x3)^2*(-0.12347999999999999*cos(x1)*sin(x3) - (0.2429 + 2.7105054312137602^-20*0)*(1. + 1.*cos(2.*x1))*sin(2.*x3)) - 0.041990608799999996*sin(x1)*(2.0940000000000003 - 0.7010000000000001*cos(2.*x1) + 0.0005*sin(2.*x1))*sin(2.*x1)*(-1.1102230246251565^-16*cos(x1)*cos(x3) - 1.4080000000000001*sin(x3))*sin(x3)^2*(-0.12347999999999999*cos(x1)*sin(x3) - (0.2429 + 2.7105054312137602^-20*0)*(1. + 1.*cos(2.*x1))*sin(2.*x3)) + 0.4788044799999999*(-0.9715999999999999*cos(x1)^2 + 0.12347999999999999*cos(x1)*cos(x3) - 1.9431999999999998*sin(x1)^2)*sin(2.*x1)*sin(x3)*(cos(x3)*(-0.0005*cos(2.*x1) - 0.7010000000000001*sin(2.*x1)) - 1.1102230246251565^-16*sin(x1)*sin(x3))*(-0.12347999999999999*cos(x1)*sin(x3) - (0.2429 + 2.7105054312137602^-20*0)*(1. + 1.*cos(2.*x1))*sin(2.*x3)) + 1.408*(-1.4574 + 0.4858*cos(2.*x1) + 0.12348*cos(x1)*cos(x3))*(-0.9715999999999999*cos(x1)^2 + 0.12347999999999999*cos(x1)*cos(x3) - 1.9431999999999998*sin(x1)^2)*(-0.12347999999999999*cos(x1)*sin(x3) + (-0.24289999999999998 - 0.24289999999999998*cos(2.*x1))*sin(2.*x3))*(-0.12347999999999999*cos(x1)*sin(x3) - (0.2429 + 2.7105054312137602^-20*0)*(1. + 1.*cos(2.*x1))*sin(2.*x3)) + (0.12348*cos(x1) - 0.9716*cos(x3))*((0.12347999999999999*cos(x1) - 0.9715999999999999*cos(x3))*(0.12347999999999999 + 0.9715999999999999*cos(x1)*cos(x3))*sin(x1)*(2.0940000000000003 - 0.7010000000000001*cos(2.*x1) + 0.0005*sin(2.*x1))*(0.12347999999999999*sin(x1) + 0.4858*cos(x3)*sin(2.*x1)) - 5.3934634536290106^-17*(0.12347999999999999 + 0.9715999999999999*cos(x1)*cos(x3))*sin(x1)^2*sin(2.*x1)*(0.12347999999999999*sin(x1) + 0.4858*cos(x3)*sin(2.*x1))*sin(x3) + 0.34006*(0.12347999999999999 + 0.9715999999999999*cos(x1)*cos(x3))*sin(x1)*(2.0940000000000003 - 0.7010000000000001*cos(2.*x1) + 0.0005*sin(2.*x1))*sin(2.*x1)*(-1.1102230246251564^-16*cos(x1)*cos(x3) - 1.408*sin(x3))*sin(x3) - 3.775424417540307^-17*(0.12347999999999999 + 0.9715999999999999*cos(x1)*cos(x3))*sin(x1)^2*sin(2.*x1)*sin(x3)*(cos(x3)*(-0.0005*cos(2.*x1) - 0.701*sin(2.*x1)) - 1.1102230246251564^-16*sin(x1)*sin(x3)) + (cos(x3)*(-0.0005*cos(2.*x1) - 0.7010000000000001*sin(2.*x1)) - 1.1102230246251565^-16*sin(x1)*sin(x3))*(-((0.12347999999999999*cos(x1) - 0.9715999999999999*cos(x3))*(-0.9715999999999999*cos(x1)^2 + 0.12347999999999999*cos(x1)*cos(x3) - 1.9431999999999998*sin(x1)^2)*(0.12347999999999999*sin(x1) + 0.4858*cos(x3)*sin(2.*x1))) - 0.4858*(1.0327336 - 0.34006*cos(2.*x1))*sin(2.*x1)*(-1.1102230246251564^-16*cos(x1)*cos(x3) - 1.408*sin(x3))*sin(x3) - 0.34006*(-0.9715999999999999*cos(x1)^2 + 0.12347999999999999*cos(x1)*cos(x3) - 1.9431999999999998*sin(x1)^2)*sin(2.*x1)*(-1.1102230246251564^-16*cos(x1)*cos(x3) - 1.408*sin(x3))*sin(x3) - 0.059986584*sin(x1)*sin(2.*x1)*(0.12347999999999999*sin(x1) + 0.4858*cos(x3)*sin(2.*x1))*sin(x3)^2 + (1.0327336 - 0.34006*cos(2.*x1))*(0.12347999999999999*cos(x1) - 0.9715999999999999*cos(x3))*(cos(x3)*(-0.0005*cos(2.*x1) - 0.701*sin(2.*x1)) - 1.1102230246251564^-16*sin(x1)*sin(x3)) - 0.041990608799999996*sin(x1)*sin(2.*x1)*sin(x3)^2*(cos(x3)*(-0.0005*cos(2.*x1) - 0.701*sin(2.*x1)) - 1.1102230246251564^-16*sin(x1)*sin(x3))) - (1.0327336 - 0.34006*cos(2.*x1))*(0.12347999999999999*cos(x1) - 0.9715999999999999*cos(x3))*(2.0940000000000003 - 0.7010000000000001*cos(2.*x1) + 0.0005*sin(2.*x1))*((1.7510000000000001 + 2.1684043449710084^-19*0) + cos(2.*x1)*((0.3505 - 5.421010862427521^-20*0) + (0.3505 - 5.421010862427521^-20*0)*cos(2.*x3)) + cos(2.*x3)*(0.343 - (0.00025 - 2.8760394919088917^-17*0)*sin(2.*x1)) - (0.00025 - 2.8760394919088917^-17*0)*sin(2.*x1) + 1.1102230246251562^-16*cos(x1)*sin(2.*x3)) + 5.3934634536290106^-17*(1.0327336 - 0.34006*cos(2.*x1))*sin(x1)*sin(2.*x1)*sin(x3)*((1.7510000000000001 + 2.1684043449710084^-19*0) + cos(2.*x1)*((0.3505 - 5.421010862427521^-20*0) + (0.3505 - 5.421010862427521^-20*0)*cos(2.*x3)) + cos(2.*x3)*(0.343 - (0.00025 - 2.8760394919088917^-17*0)*sin(2.*x1)) - (0.00025 - 2.8760394919088917^-17*0)*sin(2.*x1) + 1.1102230246251562^-16*cos(x1)*sin(2.*x3)) + 3.775424417540307^-17*sin(x1)*(-0.9715999999999999*cos(x1)^2 + 0.12347999999999999*cos(x1)*cos(x3) - 1.9431999999999998*sin(x1)^2)*sin(2.*x1)*sin(x3)*((1.7510000000000001 + 2.1684043449710084^-19*0) + cos(2.*x1)*((0.3505 - 5.421010862427521^-20*0) + (0.3505 - 5.421010862427521^-20*0)*cos(2.*x3)) + cos(2.*x3)*(0.343 - (0.00025 - 2.8760394919088917^-17*0)*sin(2.*x1)) - (0.00025 - 2.8760394919088917^-17*0)*sin(2.*x1) + 1.1102230246251562^-16*cos(x1)*sin(2.*x3)) + 0.041990608799999996*sin(x1)*(2.0940000000000003 - 0.7010000000000001*cos(2.*x1) + 0.0005*sin(2.*x1))*sin(2.*x1)*sin(x3)^2*((1.7510000000000001 + 2.1684043449710084^-19*0) + cos(2.*x1)*((0.3505 - 5.421010862427521^-20*0) + (0.3505 - 5.421010862427521^-20*0)*cos(2.*x3)) + cos(2.*x3)*(0.343 - (0.00025 - 2.8760394919088917^-17*0)*sin(2.*x1)) - (0.00025 - 2.8760394919088917^-17*0)*sin(2.*x1) + 1.1102230246251562^-16*cos(x1)*sin(2.*x3)) + 1.1102230246251565^-16*sin(x1)*(-0.9715999999999999*cos(x1)^2 + 0.12347999999999999*cos(x1)*cos(x3) - 1.9431999999999998*sin(x1)^2)*(0.12347999999999999*sin(x1) + 0.4858*cos(x3)*sin(2.*x1))*(-0.12347999999999999*cos(x1)*sin(x3) + (-0.24289999999999998 - 0.24289999999999998*cos(2.*x1))*sin(2.*x3)) + (1.0327336 - 0.34006*cos(2.*x1))*(2.0940000000000003 - 0.7010000000000001*cos(2.*x1) + 0.0005*sin(2.*x1))*(-1.1102230246251564^-16*cos(x1)*cos(x3) - 1.408*sin(x3))*(-0.12347999999999999*cos(x1)*sin(x3) + (-0.24289999999999998 - 0.24289999999999998*cos(2.*x1))*sin(2.*x3)) + 0.12348*sin(x1)*(2.0940000000000003 - 0.7010000000000001*cos(2.*x1) + 0.0005*sin(2.*x1))*(0.12347999999999999*sin(x1) + 0.4858*cos(x3)*sin(2.*x1))*sin(x3)*(-0.12347999999999999*cos(x1)*sin(x3) + (-0.24289999999999998 - 0.24289999999999998*cos(2.*x1))*sin(2.*x3)) - 1.1102230246251565^-16*(1.0327336 - 0.34006*cos(2.*x1))*sin(x1)*(cos(x3)*(-0.0005*cos(2.*x1) - 0.701*sin(2.*x1)) - 1.1102230246251564^-16*sin(x1)*sin(x3))*(-0.12347999999999999*cos(x1)*sin(x3) + (-0.24289999999999998 - 0.24289999999999998*cos(2.*x1))*sin(2.*x3)) + (-1.4574 + 0.4858*cos(2.*x1) + 0.12348*cos(x1)*cos(x3))*(0.4858*(0.12347999999999999 + 0.9715999999999999*cos(x1)*cos(x3))*sin(x1)*sin(2.*x1)*(-1.1102230246251564^-16*cos(x1)*cos(x3) - 1.408*sin(x3))*sin(x3) - (0.12347999999999999*cos(x1) - 0.9715999999999999*cos(x3))*(0.12347999999999999 + 0.9715999999999999*cos(x1)*cos(x3))*sin(x1)*(cos(x3)*(-0.0005*cos(2.*x1) - 0.701*sin(2.*x1)) - 1.1102230246251564^-16*sin(x1)*sin(x3)) + (0.12347999999999999*cos(x1) - 0.9715999999999999*cos(x3))*(-0.9715999999999999*cos(x1)^2 + 0.12347999999999999*cos(x1)*cos(x3) - 1.9431999999999998*sin(x1)^2)*((1.7510000000000001 + 2.1684043449710084^-19*0) + cos(2.*x1)*((0.3505 - 5.421010862427521^-20*0) + (0.3505 - 5.421010862427521^-20*0)*cos(2.*x3)) + cos(2.*x3)*(0.343 - (0.00025 - 2.8760394919088917^-17*0)*sin(2.*x1)) - (0.00025 - 2.8760394919088917^-17*0)*sin(2.*x1) + 1.1102230246251562^-16*cos(x1)*sin(2.*x3)) + 0.059986584*sin(x1)*sin(2.*x1)*sin(x3)^2*((1.7510000000000001 + 2.1684043449710084^-19*0) + cos(2.*x1)*((0.3505 - 5.421010862427521^-20*0) + (0.3505 - 5.421010862427521^-20*0)*cos(2.*x3)) + cos(2.*x3)*(0.343 - (0.00025 - 2.8760394919088917^-17*0)*sin(2.*x1)) - (0.00025 - 2.8760394919088917^-17*0)*sin(2.*x1) + 1.1102230246251562^-16*cos(x1)*sin(2.*x3)) - (-0.9715999999999999*cos(x1)^2 + 0.12347999999999999*cos(x1)*cos(x3) - 1.9431999999999998*sin(x1)^2)*(-1.1102230246251564^-16*cos(x1)*cos(x3) - 1.408*sin(x3))*(-0.12347999999999999*cos(x1)*sin(x3) + (-0.24289999999999998 - 0.24289999999999998*cos(2.*x1))*sin(2.*x3)) - 0.12348*sin(x1)*sin(x3)*(cos(x3)*(-0.0005*cos(2.*x1) - 0.701*sin(2.*x1)) - 1.1102230246251564^-16*sin(x1)*sin(x3))*(-0.12347999999999999*cos(x1)*sin(x3) + (-0.24289999999999998 - 0.24289999999999998*cos(2.*x1))*sin(2.*x3)))) - 0.12348*sin(x1)*sin(x3)*((0.12347999999999999 + 0.9715999999999999*cos(x1)*cos(x3))*(0.8627035999999999 + cos(2.*x1)*(0.17003 - 0.17003*cos(2.*x3)) - 0.17003*cos(2.*x3))*sin(x1)*(2.0940000000000003 - 0.7010000000000001*cos(2.*x1) + 0.0005*sin(2.*x1))*(-1.1102230246251564^-16*cos(x1)*cos(x3) - 1.408*sin(x3)) - 1.1102230246251565^-16*(0.12347999999999999 + 0.9715999999999999*cos(x1)*cos(x3))*(0.8627035999999999 + cos(2.*x1)*(0.17003 - 0.17003*cos(2.*x3)) - 0.17003*cos(2.*x3))*sin(x1)^2*(cos(x3)*(-0.0005*cos(2.*x1) - 0.701*sin(2.*x1)) - 1.1102230246251564^-16*sin(x1)*sin(x3)) + 1.1102230246251565^-16*(0.8627035999999999 + cos(2.*x1)*(0.17003 - 0.17003*cos(2.*x3)) - 0.17003*cos(2.*x3))*sin(x1)*(-0.9715999999999999*cos(x1)^2 + 0.12347999999999999*cos(x1)*cos(x3) - 1.9431999999999998*sin(x1)^2)*((1.7510000000000001 + 2.1684043449710084^-19*0) + cos(2.*x1)*((0.3505 - 5.421010862427521^-20*0) + (0.3505 - 5.421010862427521^-20*0)*cos(2.*x3)) + cos(2.*x3)*(0.343 - (0.00025 - 2.8760394919088917^-17*0)*sin(2.*x1)) - (0.00025 - 2.8760394919088917^-17*0)*sin(2.*x1) + 1.1102230246251562^-16*cos(x1)*sin(2.*x3)) + 0.12348*(0.8627035999999999 + cos(2.*x1)*(0.17003 - 0.17003*cos(2.*x3)) - 0.17003*cos(2.*x3))*sin(x1)*(2.0940000000000003 - 0.7010000000000001*cos(2.*x1) + 0.0005*sin(2.*x1))*sin(x3)*((1.7510000000000001 + 2.1684043449710084^-19*0) + cos(2.*x1)*((0.3505 - 5.421010862427521^-20*0) + (0.3505 - 5.421010862427521^-20*0)*cos(2.*x3)) + cos(2.*x3)*(0.343 - (0.00025 - 2.8760394919088917^-17*0)*sin(2.*x1)) - (0.00025 - 2.8760394919088917^-17*0)*sin(2.*x1) + 1.1102230246251562^-16*cos(x1)*sin(2.*x3)) - (0.12347999999999999*cos(x1) - 0.9715999999999999*cos(x3))*(0.12347999999999999 + 0.9715999999999999*cos(x1)*cos(x3))*sin(x1)*(2.0940000000000003 - 0.7010000000000001*cos(2.*x1) + 0.0005*sin(2.*x1))*(-0.12347999999999999*cos(x1)*sin(x3) - (0.2429 + 2.7105054312137602^-20*0)*(1. + 1.*cos(2.*x1))*sin(2.*x3)) + 5.3934634536290106^-17*(0.12347999999999999 + 0.9715999999999999*cos(x1)*cos(x3))*sin(x1)^2*sin(2.*x1)*sin(x3)*(-0.12347999999999999*cos(x1)*sin(x3) - (0.2429 + 2.7105054312137602^-20*0)*(1. + 1.*cos(2.*x1))*sin(2.*x3)) - 1.1102230246251565^-16*sin(x1)*(-0.9715999999999999*cos(x1)^2 + 0.12347999999999999*cos(x1)*cos(x3) - 1.9431999999999998*sin(x1)^2)*(-0.12347999999999999*cos(x1)*sin(x3) + (-0.24289999999999998 - 0.24289999999999998*cos(2.*x1))*sin(2.*x3))*(-0.12347999999999999*cos(x1)*sin(x3) - (0.2429 + 2.7105054312137602^-20*0)*(1. + 1.*cos(2.*x1))*sin(2.*x3)) - 0.12348*sin(x1)*(2.0940000000000003 - 0.7010000000000001*cos(2.*x1) + 0.0005*sin(2.*x1))*sin(x3)*(-0.12347999999999999*cos(x1)*sin(x3) + (-0.24289999999999998 - 0.24289999999999998*cos(2.*x1))*sin(2.*x3))*(-0.12347999999999999*cos(x1)*sin(x3) - (0.2429 + 2.7105054312137602^-20*0)*(1. + 1.*cos(2.*x1))*sin(2.*x3)) - 0.34006*sin(2.*x1)*sin(x3)*((0.12347999999999999*cos(x1) - 0.9715999999999999*cos(x3))*(2.0940000000000003 - 0.7010000000000001*cos(2.*x1) + 0.0005*sin(2.*x1))*((1.7510000000000001 + 2.1684043449710084^-19*0) + cos(2.*x1)*((0.3505 - 5.421010862427521^-20*0) + (0.3505 - 5.421010862427521^-20*0)*cos(2.*x3)) + cos(2.*x3)*(0.343 - (0.00025 - 2.8760394919088917^-17*0)*sin(2.*x1)) - (0.00025 - 2.8760394919088917^-17*0)*sin(2.*x1) + 1.1102230246251562^-16*cos(x1)*sin(2.*x3)) - 5.3934634536290106^-17*sin(x1)*sin(2.*x1)*sin(x3)*((1.7510000000000001 + 2.1684043449710084^-19*0) + cos(2.*x1)*((0.3505 - 5.421010862427521^-20*0) + (0.3505 - 5.421010862427521^-20*0)*cos(2.*x3)) + cos(2.*x3)*(0.343 - (0.00025 - 2.8760394919088917^-17*0)*sin(2.*x1)) - (0.00025 - 2.8760394919088917^-17*0)*sin(2.*x1) + 1.1102230246251562^-16*cos(x1)*sin(2.*x3)) - (2.0940000000000003 - 0.7010000000000001*cos(2.*x1) + 0.0005*sin(2.*x1))*(-1.1102230246251564^-16*cos(x1)*cos(x3) - 1.408*sin(x3))*(-0.12347999999999999*cos(x1)*sin(x3) + (-0.24289999999999998 - 0.24289999999999998*cos(2.*x1))*sin(2.*x3)) + 1.1102230246251565^-16*sin(x1)*(cos(x3)*(-0.0005*cos(2.*x1) - 0.701*sin(2.*x1)) - 1.1102230246251564^-16*sin(x1)*sin(x3))*(-0.12347999999999999*cos(x1)*sin(x3) + (-0.24289999999999998 - 0.24289999999999998*cos(2.*x1))*sin(2.*x3))) + 0.4858*sin(2.*x1)*sin(x3)*(-0.4858*(0.12347999999999999 + 0.9715999999999999*cos(x1)*cos(x3))*sin(x1)*sin(2.*x1)*(-1.1102230246251564^-16*cos(x1)*cos(x3) - 1.408*sin(x3))*sin(x3) + (0.12347999999999999*cos(x1) - 0.9715999999999999*cos(x3))*(0.12347999999999999 + 0.9715999999999999*cos(x1)*cos(x3))*sin(x1)*(cos(x3)*(-0.0005*cos(2.*x1) - 0.701*sin(2.*x1)) - 1.1102230246251564^-16*sin(x1)*sin(x3)) - (0.12347999999999999*cos(x1) - 0.9715999999999999*cos(x3))*(-0.9715999999999999*cos(x1)^2 + 0.12347999999999999*cos(x1)*cos(x3) - 1.9431999999999998*sin(x1)^2)*((1.7510000000000001 + 2.1684043449710084^-19*0) + cos(2.*x1)*((0.3505 - 5.421010862427521^-20*0) + (0.3505 - 5.421010862427521^-20*0)*cos(2.*x3)) + cos(2.*x3)*(0.343 - (0.00025 - 2.8760394919088917^-17*0)*sin(2.*x1)) - (0.00025 - 2.8760394919088917^-17*0)*sin(2.*x1) + 1.1102230246251562^-16*cos(x1)*sin(2.*x3)) - 0.059986584*sin(x1)*sin(2.*x1)*sin(x3)^2*((1.7510000000000001 + 2.1684043449710084^-19*0) + cos(2.*x1)*((0.3505 - 5.421010862427521^-20*0) + (0.3505 - 5.421010862427521^-20*0)*cos(2.*x3)) + cos(2.*x3)*(0.343 - (0.00025 - 2.8760394919088917^-17*0)*sin(2.*x1)) - (0.00025 - 2.8760394919088917^-17*0)*sin(2.*x1) + 1.1102230246251562^-16*cos(x1)*sin(2.*x3)) + (-0.9715999999999999*cos(x1)^2 + 0.12347999999999999*cos(x1)*cos(x3) - 1.9431999999999998*sin(x1)^2)*(-1.1102230246251564^-16*cos(x1)*cos(x3) - 1.408*sin(x3))*(-0.12347999999999999*cos(x1)*sin(x3) + (-0.24289999999999998 - 0.24289999999999998*cos(2.*x1))*sin(2.*x3)) + 0.12348*sin(x1)*sin(x3)*(cos(x3)*(-0.0005*cos(2.*x1) - 0.701*sin(2.*x1)) - 1.1102230246251564^-16*sin(x1)*sin(x3))*(-0.12347999999999999*cos(x1)*sin(x3) + (-0.24289999999999998 - 0.24289999999999998*cos(2.*x1))*sin(2.*x3))) + (cos(x3)*(-0.0005*cos(2.*x1) - 0.7010000000000001*sin(2.*x1)) - 1.1102230246251565^-16*sin(x1)*sin(x3))*(-((0.8627035999999999 + cos(2.*x1)*(0.17003 - 0.17003*cos(2.*x3)) - 0.17003*cos(2.*x3))*(-0.9715999999999999*cos(x1)^2 + 0.12347999999999999*cos(x1)*cos(x3) - 1.9431999999999998*sin(x1)^2)*(-1.1102230246251564^-16*cos(x1)*cos(x3) - 1.408*sin(x3))) - 0.165201148*sin(2.*x1)^2*(-1.1102230246251564^-16*cos(x1)*cos(x3) - 1.408*sin(x3))*sin(x3)^2 - 0.12348*(0.8627035999999999 + cos(2.*x1)*(0.17003 - 0.17003*cos(2.*x3)) - 0.17003*cos(2.*x3))*sin(x1)*sin(x3)*(cos(x3)*(-0.0005*cos(2.*x1) - 0.701*sin(2.*x1)) - 1.1102230246251564^-16*sin(x1)*sin(x3)) + 0.34006*(0.12347999999999999*cos(x1) - 0.9715999999999999*cos(x3))*sin(2.*x1)*sin(x3)*(cos(x3)*(-0.0005*cos(2.*x1) - 0.701*sin(2.*x1)) - 1.1102230246251564^-16*sin(x1)*sin(x3)) + (0.12347999999999999*cos(x1) - 0.9715999999999999*cos(x3))*(-0.9715999999999999*cos(x1)^2 + 0.12347999999999999*cos(x1)*cos(x3) - 1.9431999999999998*sin(x1)^2)*(-0.12347999999999999*cos(x1)*sin(x3) - (0.2429 + 2.7105054312137602^-20*0)*(1. + 1.*cos(2.*x1))*sin(2.*x3)) + 0.059986584*sin(x1)*sin(2.*x1)*sin(x3)^2*(-0.12347999999999999*cos(x1)*sin(x3) - (0.2429 + 2.7105054312137602^-20*0)*(1. + 1.*cos(2.*x1))*sin(2.*x3)))) + (1.0327336 - 0.34006*cos(2.*x1))*(0. + (-1.1102230246251565^-16*cos(x1)*cos(x3) - 1.4080000000000001*sin(x3))*(-((0.8627035999999999 + cos(2.*x1)*(0.17003 - 0.17003*cos(2.*x3)) - 0.17003*cos(2.*x3))*(2.0940000000000003 - 0.7010000000000001*cos(2.*x1) + 0.0005*sin(2.*x1))*(-1.1102230246251564^-16*cos(x1)*cos(x3) - 1.408*sin(x3))) + 0.23600164*sin(2.*x1)^2*(-1.1102230246251564^-16*cos(x1)*cos(x3) - 1.408*sin(x3))*sin(x3)^2 + 1.1102230246251565^-16*(0.8627035999999999 + cos(2.*x1)*(0.17003 - 0.17003*cos(2.*x3)) - 0.17003*cos(2.*x3))*sin(x1)*(cos(x3)*(-0.0005*cos(2.*x1) - 0.701*sin(2.*x1)) - 1.1102230246251564^-16*sin(x1)*sin(x3)) - 0.4858*(0.12347999999999999*cos(x1) - 0.9715999999999999*cos(x3))*sin(2.*x1)*sin(x3)*(cos(x3)*(-0.0005*cos(2.*x1) - 0.701*sin(2.*x1)) - 1.1102230246251564^-16*sin(x1)*sin(x3)) + (0.12347999999999999*cos(x1) - 0.9715999999999999*cos(x3))*(2.0940000000000003 - 0.7010000000000001*cos(2.*x1) + 0.0005*sin(2.*x1))*(-0.12347999999999999*cos(x1)*sin(x3) - (0.2429 + 2.7105054312137602^-20*0)*(1. + 1.*cos(2.*x1))*sin(2.*x3)) - 5.3934634536290106^-17*sin(x1)*sin(2.*x1)*sin(x3)*(-0.12347999999999999*cos(x1)*sin(x3) - (0.2429 + 2.7105054312137602^-20*0)*(1. + 1.*cos(2.*x1))*sin(2.*x3))) + 1.408*(-((0.8627035999999999 + cos(2.*x1)*(0.17003 - 0.17003*cos(2.*x3)) - 0.17003*cos(2.*x3))*(cos(x3)*(-0.0005*cos(2.*x1) - 0.7010000000000001*sin(2.*x1)) - 1.1102230246251565^-16*sin(x1)*sin(x3))^2) + (0.8627035999999999 + cos(2.*x1)*(0.17003 - 0.17003*cos(2.*x3)) - 0.17003*cos(2.*x3))*(2.0940000000000003 - 0.7010000000000001*cos(2.*x1) + 0.0005*sin(2.*x1))*((1.7510000000000001 + 2.1684043449710084^-19*0) + cos(2.*x1)*((0.3505 - 5.421010862427521^-20*0) + (0.3505 - 5.421010862427521^-20*0)*cos(2.*x3)) + cos(2.*x3)*(0.343 - (0.00025 - 2.8760394919088917^-17*0)*sin(2.*x1)) - (0.00025 - 2.8760394919088917^-17*0)*sin(2.*x1) + 1.1102230246251562^-16*cos(x1)*sin(2.*x3)) - 0.23600164*sin(2.*x1)^2*sin(x3)^2*((1.7510000000000001 + 2.1684043449710084^-19*0) + cos(2.*x1)*((0.3505 - 5.421010862427521^-20*0) + (0.3505 - 5.421010862427521^-20*0)*cos(2.*x3)) + cos(2.*x3)*(0.343 - (0.00025 - 2.8760394919088917^-17*0)*sin(2.*x1)) - (0.00025 - 2.8760394919088917^-17*0)*sin(2.*x1) + 1.1102230246251562^-16*cos(x1)*sin(2.*x3)) + 0.4858*sin(2.*x1)*sin(x3)*(cos(x3)*(-0.0005*cos(2.*x1) - 0.701*sin(2.*x1)) - 1.1102230246251564^-16*sin(x1)*sin(x3))*(-0.12347999999999999*cos(x1)*sin(x3) + (-0.24289999999999998 - 0.24289999999999998*cos(2.*x1))*sin(2.*x3)) + 0.4858*sin(2.*x1)*sin(x3)*(cos(x3)*(-0.0005*cos(2.*x1) - 0.7010000000000001*sin(2.*x1)) - 1.1102230246251565^-16*sin(x1)*sin(x3))*(-0.12347999999999999*cos(x1)*sin(x3) - (0.2429 + 2.7105054312137602^-20*0)*(1. + 1.*cos(2.*x1))*sin(2.*x3)) - (2.0940000000000003 - 0.7010000000000001*cos(2.*x1) + 0.0005*sin(2.*x1))*(-0.12347999999999999*cos(x1)*sin(x3) + (-0.24289999999999998 - 0.24289999999999998*cos(2.*x1))*sin(2.*x3))*(-0.12347999999999999*cos(x1)*sin(x3) - (0.2429 + 2.7105054312137602^-20*0)*(1. + 1.*cos(2.*x1))*sin(2.*x3))))), x4, (((0.12348*cos(x1) - 0.9716*cos(x3))*((0.12347999999999999*cos(x1) - 0.9715999999999999*cos(x3))*(0.12347999999999999*sin(x1) + 0.4858*cos(x3)*sin(2.*x1))*(cos(x3)*(-0.0005*cos(2.*x1) - 0.7010000000000001*sin(2.*x1)) - 1.1102230246251565^-16*sin(x1)*sin(x3)) + 0.34006*sin(2.*x1)*(-1.1102230246251564^-16*cos(x1)*cos(x3) - 1.408*sin(x3))*sin(x3)*(cos(x3)*(-0.0005*cos(2.*x1) - 0.7010000000000001*sin(2.*x1)) - 1.1102230246251565^-16*sin(x1)*sin(x3)) - 3.775424417540307^-17*sin(x1)*sin(2.*x1)*sin(x3)*((1.7510000000000001 + 2.1684043449710084^-19*0) + cos(2.*x1)*((0.3505 - 5.421010862427521^-20*0) + (0.3505 - 5.421010862427521^-20*0)*cos(2.*x3)) + cos(2.*x3)*(0.343 - (0.00025 - 2.8760394919088917^-17*0)*sin(2.*x1)) - (0.00025 - 2.8760394919088917^-17*0)*sin(2.*x1) + 1.1102230246251562^-16*cos(x1)*sin(2.*x3)) - 1.1102230246251565^-16*sin(x1)*(0.12347999999999999*sin(x1) + 0.4858*cos(x3)*sin(2.*x1))*(-0.12347999999999999*cos(x1)*sin(x3) + (-0.24289999999999998 - 0.24289999999999998*cos(2.*x1))*sin(2.*x3))) + (1.1102230246251565^-16*sin(x1)*(-1.1102230246251565^-16*cos(x1)*cos(x3) - 1.4080000000000001*sin(x3)) - 1.408*(cos(x3)*(-0.0005*cos(2.*x1) - 0.7010000000000001*sin(2.*x1)) - 1.1102230246251565^-16*sin(x1)*sin(x3)))*((0.8627035999999999 + cos(2.*x1)*(0.17003 - 0.17003*cos(2.*x3)) - 0.17003*cos(2.*x3))*(0.12347999999999999*sin(x1) + 0.4858*cos(x3)*sin(2.*x1)) + 0.34006*sin(2.*x1)*sin(x3)*(-0.12347999999999999*cos(x1)*sin(x3) - (0.2429 + 2.7105054312137602^-20*0)*(1. + 1.*cos(2.*x1))*sin(2.*x3))) - 0.12348*sin(x1)*sin(x3)*((0.8627035999999999 + cos(2.*x1)*(0.17003 - 0.17003*cos(2.*x3)) - 0.17003*cos(2.*x3))*(-1.1102230246251564^-16*cos(x1)*cos(x3) - 1.408*sin(x3))*(cos(x3)*(-0.0005*cos(2.*x1) - 0.7010000000000001*sin(2.*x1)) - 1.1102230246251565^-16*sin(x1)*sin(x3)) - 1.1102230246251565^-16*(0.8627035999999999 + cos(2.*x1)*(0.17003 - 0.17003*cos(2.*x3)) - 0.17003*cos(2.*x3))*sin(x1)*((1.7510000000000001 + 2.1684043449710084^-19*0) + cos(2.*x1)*((0.3505 - 5.421010862427521^-20*0) + (0.3505 - 5.421010862427521^-20*0)*cos(2.*x3)) + cos(2.*x3)*(0.343 - (0.00025 - 2.8760394919088917^-17*0)*sin(2.*x1)) - (0.00025 - 2.8760394919088917^-17*0)*sin(2.*x1) + 1.1102230246251562^-16*cos(x1)*sin(2.*x3)) - (0.12347999999999999*cos(x1) - 0.9715999999999999*cos(x3))*(cos(x3)*(-0.0005*cos(2.*x1) - 0.7010000000000001*sin(2.*x1)) - 1.1102230246251565^-16*sin(x1)*sin(x3))*(-0.12347999999999999*cos(x1)*sin(x3) - (0.2429 + 2.7105054312137602^-20*0)*(1. + 1.*cos(2.*x1))*sin(2.*x3)) + 1.1102230246251565^-16*sin(x1)*(-0.12347999999999999*cos(x1)*sin(x3) + (-0.24289999999999998 - 0.24289999999999998*cos(2.*x1))*sin(2.*x3))*(-0.12347999999999999*cos(x1)*sin(x3) - (0.2429 + 2.7105054312137602^-20*0)*(1. + 1.*cos(2.*x1))*sin(2.*x3))))*((1.4288690166235203*cos(x1) + 1.6499158227686102*sin(x1))*u1 + 1.6499158227686104*sin(x1)*u2 + 1.6499158227686102*sin(x1)*u3 + 0.68012*sin(2.*x1)*x10*x2 + cos(x1)*(-1.4288690166235203*u3 - 0.12348*sin(x3)*x2^2) - 0.24696*cos(x3)*sin(x1)*x2*x4 - 0.9716000000000001*sin(2.*x1)*x2*x4 - 0.12348*cos(x1)*sin(x3)*x4^2 + ((0.12347999999999998*cos(x1) + 0.9716*cos(x1)^2*cos(x3) - 0.9716*cos(x3)*sin(x1)^2)*x2 - 0.4858*sin(2*x1)*sin(x3)*x4)*x6 + (-0.68012*cos(2.*x1)*sin(x3)*x2 - 0.34006*cos(x3)*sin(2.*x1)*x4)*x8) - (0.12348*cos(x1) - 0.9716*cos(x3))^2*(0.12347999999999999 + 0.9715999999999999*cos(x1)*cos(x3))*sin(x1)*(0.12347999999999999*sin(x1) + 0.4858*cos(x3)*sin(2.*x1))*(-17.304840000000002*cos(x1)*sin(x3) + (-0.8164965809277263*cos(x1) - 0.9428090415820632*sin(x1))*u1 + (0.6123724356957947*cos(x1) - 0.9428090415820637*sin(x1))*u2 + 2.041241452319315*cos(x1)*u3 - 0.9428090415820632*sin(x1)*u3 - 0.9716*sin(2.*x1)*x10*x2 + 1.1102230246251565^-16*cos(x1)*x2^2 + (-1.3877787807814457^-17*cos(x1)*sin(x3)*x10 + (0.001*cos(2.*x1) + 1.4020000000000001*sin(2.*x1))*x2)*x4 + (-1.1102230246251565^-16*cos(x1)*cos(2.*x3) + ((0.343 - 1.4444474582904269^-34*0) + (0.35050000000000003 - 1.6263032587282571^-19*0)*cos(2.*x1) - (0.00025 - 1.3877787807814454^-16*0)*sin(2.*x1))*sin(2.*x3))*x6^2 + (0.34006000000000003*cos(x3)*sin(2.*x1)*x10 + (-0.9716 + 0.9716*cos(2.*x1))*sin(x3)*x2)*x8 + (-0.34006000000000003*cos(2.*x1)*cos(x3)*sin(x3) - 0.17003000000000001*sin(2.*x3))*x8^2 + x6*(0.4858*sin(2.*x1)*sin(x3)*x10 + (cos(x3)*(1.4080000000000001 - 1.4020000000000001*cos(2.*x1) + 0.001*sin(2.*x1)) - 2.220446049250313^-16*cos(x1)*sin(x3))*x2 + 1.1102230246251565^-16*sin(2.*x1)*sin(x3)*x4 + (0.12348*cos(x1)*cos(x3) + (0.4858 + 0.4858*cos(2.*x1))*cos(2.*x3))*x8)) + 1.408*(0.12347999999999999 + 0.9715999999999999*cos(x1)*cos(x3))*(0.8627035999999999 + cos(2.*x1)*(0.17003 - 0.17003*cos(2.*x3)) - 0.17003*cos(2.*x3))*sin(x1)*(0.12347999999999999*sin(x1) + 0.4858*cos(x3)*sin(2.*x1))*(-17.304840000000002*cos(x1)*sin(x3) + (-0.8164965809277263*cos(x1) - 0.9428090415820632*sin(x1))*u1 + (0.6123724356957947*cos(x1) - 0.9428090415820637*sin(x1))*u2 + 2.041241452319315*cos(x1)*u3 - 0.9428090415820632*sin(x1)*u3 - 0.9716*sin(2.*x1)*x10*x2 + 1.1102230246251565^-16*cos(x1)*x2^2 + (-1.3877787807814457^-17*cos(x1)*sin(x3)*x10 + (0.001*cos(2.*x1) + 1.4020000000000001*sin(2.*x1))*x2)*x4 + (-1.1102230246251565^-16*cos(x1)*cos(2.*x3) + ((0.343 - 1.4444474582904269^-34*0) + (0.35050000000000003 - 1.6263032587282571^-19*0)*cos(2.*x1) - (0.00025 - 1.3877787807814454^-16*0)*sin(2.*x1))*sin(2.*x3))*x6^2 + (0.34006000000000003*cos(x3)*sin(2.*x1)*x10 + (-0.9716 + 0.9716*cos(2.*x1))*sin(x3)*x2)*x8 + (-0.34006000000000003*cos(2.*x1)*cos(x3)*sin(x3) - 0.17003000000000001*sin(2.*x3))*x8^2 + x6*(0.4858*sin(2.*x1)*sin(x3)*x10 + (cos(x3)*(1.4080000000000001 - 1.4020000000000001*cos(2.*x1) + 0.001*sin(2.*x1)) - 2.220446049250313^-16*cos(x1)*sin(x3))*x2 + 1.1102230246251565^-16*sin(2.*x1)*sin(x3)*x4 + (0.12348*cos(x1)*cos(x3) + (0.4858 + 0.4858*cos(2.*x1))*cos(2.*x3))*x8)) + (1.0327336 - 0.34006*cos(2.*x1))*(0.8627035999999999 + cos(2.*x1)*(0.17003 - 0.17003*cos(2.*x3)) - 0.17003*cos(2.*x3))*(-1.1102230246251565^-16*cos(x1)*cos(x3) - 1.4080000000000001*sin(x3))^2*(-17.304840000000002*cos(x1)*sin(x3) + (-0.8164965809277263*cos(x1) - 0.9428090415820632*sin(x1))*u1 + (0.6123724356957947*cos(x1) - 0.9428090415820637*sin(x1))*u2 + 2.041241452319315*cos(x1)*u3 - 0.9428090415820632*sin(x1)*u3 - 0.9716*sin(2.*x1)*x10*x2 + 1.1102230246251565^-16*cos(x1)*x2^2 + (-1.3877787807814457^-17*cos(x1)*sin(x3)*x10 + (0.001*cos(2.*x1) + 1.4020000000000001*sin(2.*x1))*x2)*x4 + (-1.1102230246251565^-16*cos(x1)*cos(2.*x3) + ((0.343 - 1.4444474582904269^-34*0) + (0.35050000000000003 - 1.6263032587282571^-19*0)*cos(2.*x1) - (0.00025 - 1.3877787807814454^-16*0)*sin(2.*x1))*sin(2.*x3))*x6^2 + (0.34006000000000003*cos(x3)*sin(2.*x1)*x10 + (-0.9716 + 0.9716*cos(2.*x1))*sin(x3)*x2)*x8 + 